simulink model "FeedBack_Linearization"  (R2021b)
(part 6 of 9)

t2824 = ct{938};
t2825 = ct{939};
t2826 = ct{940};
t2827 = ct{941};
t2828 = ct{942};
t2829 = ct{943};
t283 = ct{944};
t2832 = ct{945};
t2833 = ct{946};
t2837 = ct{947};
t2838 = ct{948};
t2839 = ct{949};
t284 = ct{950};
t2840 = ct{951};
t2841 = ct{952};
t2842 = ct{953};
t2844 = ct{954};
t2845 = ct{955};
t2846 = ct{956};
t2847 = ct{957};
t2848 = ct{958};
t285 = ct{959};
t2852 = ct{960};
t2854 = ct{961};
t2855 = ct{962};
t2857 = ct{963};
t2858 = ct{964};
t286 = ct{965};
t2861 = ct{966};
t2862 = ct{967};
t2864 = ct{968};
t2867 = ct{969};
t2868 = ct{970};
t2869 = ct{971};
t287 = ct{972};
t2871 = ct{973};
t2878 = ct{974};
t288 = ct{975};
t2880 = ct{976};
t2881 = ct{977};
t2882 = ct{978};
t2883 = ct{979};
t2884 = ct{980};
t2885 = ct{981};
t2886 = ct{982};
t2887 = ct{983};
t289 = ct{984};
t2891 = ct{985};
t2895 = ct{986};
t2897 = ct{987};
t2898 = ct{988};
t29 = ct{989};
t290 = ct{990};
t2900 = ct{991};
t2901 = ct{992};
t2903 = ct{993};
t2905 = ct{994};
t2907 = ct{995};
t2908 = ct{996};
t2909 = ct{997};
t2911 = ct{998};
t2912 = ct{999};
t2914 = ct{1000};
t2915 = ct{1001};
t2917 = ct{1002};
t2919 = ct{1003};
t2920 = ct{1004};
t2921 = ct{1005};
t2922 = ct{1006};
t2923 = ct{1007};
t2924 = ct{1008};
t2925 = ct{1009};
t2926 = ct{1010};
t2929 = ct{1011};
t293 = ct{1012};
t2930 = ct{1013};
t2931 = ct{1014};
t2935 = ct{1015};
t2936 = ct{1016};
t2937 = ct{1017};
t2939 = ct{1018};
t2940 = ct{1019};
t2941 = ct{1020};
t2942 = ct{1021};
t2943 = ct{1022};
t2944 = ct{1023};
t2945 = ct{1024};
t2946 = ct{1025};
t2947 = ct{1026};
t2948 = ct{1027};
t2949 = ct{1028};
t295 = ct{1029};
t2950 = ct{1030};
t2952 = ct{1031};
t2953 = ct{1032};
t2954 = ct{1033};
t2955 = ct{1034};
t2956 = ct{1035};
t2957 = ct{1036};
t2959 = ct{1037};
t296 = ct{1038};
t2960 = ct{1039};
t2961 = ct{1040};
t2962 = ct{1041};
t2968 = ct{1042};
t2969 = ct{1043};
t297 = ct{1044};
t2970 = ct{1045};
t2972 = ct{1046};
t2973 = ct{1047};
t2974 = ct{1048};
t2976 = ct{1049};
t298 = ct{1050};
t2980 = ct{1051};
t2981 = ct{1052};
t2982 = ct{1053};
t2985 = ct{1054};
t2989 = ct{1055};
t2990 = ct{1056};
t2991 = ct{1057};
t2992 = ct{1058};
t2993 = ct{1059};
t2994 = ct{1060};
t2995 = ct{1061};
t2996 = ct{1062};
t2997 = ct{1063};
t2998 = ct{1064};
t2999 = ct{1065};
t3 = ct{1066};
t30 = ct{1067};
t3001 = ct{1068};
t3003 = ct{1069};
t3005 = ct{1070};
t3007 = ct{1071};
t3008 = ct{1072};
t3009 = ct{1073};
t301 = ct{1074};
t3011 = ct{1075};
t3013 = ct{1076};
t3016 = ct{1077};
t3018 = ct{1078};
t3020 = ct{1079};
t3021 = ct{1080};
t3022 = ct{1081};
t3023 = ct{1082};
t3025 = ct{1083};
t3026 = ct{1084};
t3030 = ct{1085};
t3031 = ct{1086};
t3032 = ct{1087};
t3035 = ct{1088};
t3037 = ct{1089};
t3038 = ct{1090};
t3039 = ct{1091};
t3042 = ct{1092};
t3045 = ct{1093};
t3049 = ct{1094};
t3051 = ct{1095};
t3052 = ct{1096};
t3055 = ct{1097};
t3056 = ct{1098};
t3057 = ct{1099};
t3059 = ct{1100};
t3060 = ct{1101};
t3062 = ct{1102};
t3064 = ct{1103};
t3065 = ct{1104};
t3066 = ct{1105};
t3067 = ct{1106};
t3068 = ct{1107};
t307 = ct{1108};
t3070 = ct{1109};
t3071 = ct{1110};
t3073 = ct{1111};
t3075 = ct{1112};
t3076 = ct{1113};
t3079 = ct{1114};
t308 = ct{1115};
t3080 = ct{1116};
t3082 = ct{1117};
t3083 = ct{1118};
t3084 = ct{1119};
t3085 = ct{1120};
t3086 = ct{1121};
t3088 = ct{1122};
t309 = ct{1123};
t3090 = ct{1124};
t3092 = ct{1125};
t3093 = ct{1126};
t3094 = ct{1127};
t3096 = ct{1128};
t3097 = ct{1129};
t3098 = ct{1130};
t31 = ct{1131};
t310 = ct{1132};
t3101 = ct{1133};
t3102 = ct{1134};
t3103 = ct{1135};
t3104 = ct{1136};
t3108 = ct{1137};
t311 = ct{1138};
t3112 = ct{1139};
t3113 = ct{1140};
t3114 = ct{1141};
t3115 = ct{1142};
t3116 = ct{1143};
t3118 = ct{1144};
t3119 = ct{1145};
t312 = ct{1146};
t3120 = ct{1147};
t3121 = ct{1148};
t3122 = ct{1149};
t3124 = ct{1150};
t3126 = ct{1151};
t3128 = ct{1152};
t3129 = ct{1153};
t313 = ct{1154};
t3130 = ct{1155};
t3131 = ct{1156};
t3132 = ct{1157};
t3133 = ct{1158};
t3138 = ct{1159};
t3139 = ct{1160};
t3140 = ct{1161};
t3141 = ct{1162};
t3142 = ct{1163};
t3143 = ct{1164};
t3147 = ct{1165};
t3148 = ct{1166};
t3149 = ct{1167};
t3152 = ct{1168};
t3153 = ct{1169};
t3154 = ct{1170};
t3155 = ct{1171};
t3156 = ct{1172};
t3159 = ct{1173};
t3161 = ct{1174};
t3162 = ct{1175};
t3163 = ct{1176};
t3165 = ct{1177};
t3166 = ct{1178};
t3167 = ct{1179};
t3168 = ct{1180};
t317 = ct{1181};
t3170 = ct{1182};
t3171 = ct{1183};
t3172 = ct{1184};
t3175 = ct{1185};
t3176 = ct{1186};
t3179 = ct{1187};
t318 = ct{1188};
t3181 = ct{1189};
t3182 = ct{1190};
t3186 = ct{1191};
t3187 = ct{1192};
t319 = ct{1193};
t3190 = ct{1194};
t3191 = ct{1195};
t3192 = ct{1196};
t3193 = ct{1197};
t3194 = ct{1198};
t3195 = ct{1199};
t3196 = ct{1200};
t32 = ct{1201};
t320 = ct{1202};
t3201 = ct{1203};
t3202 = ct{1204};
t3203 = ct{1205};
t3204 = ct{1206};
t3205 = ct{1207};
t3206 = ct{1208};
t3208 = ct{1209};
t3210 = ct{1210};
t3211 = ct{1211};
t3212 = ct{1212};
t3213 = ct{1213};
t3214 = ct{1214};
t3215 = ct{1215};
t3216 = ct{1216};
t3220 = ct{1217};
t3222 = ct{1218};
t3223 = ct{1219};
t3224 = ct{1220};
t3225 = ct{1221};
t3226 = ct{1222};
t3227 = ct{1223};
t3228 = ct{1224};
t3229 = ct{1225};
t3230 = ct{1226};
t3231 = ct{1227};
t3232 = ct{1228};
t3233 = ct{1229};
t3235 = ct{1230};
t3236 = ct{1231};
t3237 = ct{1232};
t3238 = ct{1233};
t3240 = ct{1234};
t3241 = ct{1235};
t3242 = ct{1236};
t3243 = ct{1237};
t3244 = ct{1238};
t3246 = ct{1239};
t3247 = ct{1240};
t3248 = ct{1241};
t3249 = ct{1242};
t3250 = ct{1243};
t3251 = ct{1244};
t3252 = ct{1245};
t3253 = ct{1246};
t3254 = ct{1247};
t3255 = ct{1248};
t3256 = ct{1249};
t3257 = ct{1250};
t3259 = ct{1251};
t3261 = ct{1252};
t3262 = ct{1253};
t3263 = ct{1254};
t3264 = ct{1255};
t3267 = ct{1256};
t3268 = ct{1257};
t3269 = ct{1258};
t327 = ct{1259};
t3272 = ct{1260};
t3273 = ct{1261};
t3274 = ct{1262};
t3275 = ct{1263};
t3276 = ct{1264};
t3277 = ct{1265};
t3279 = ct{1266};
t328 = ct{1267};
t3280 = ct{1268};
t3281 = ct{1269};
t3282 = ct{1270};
t3284 = ct{1271};
t3285 = ct{1272};
t3286 = ct{1273};
t3287 = ct{1274};
t3288 = ct{1275};
t3289 = ct{1276};
t329 = ct{1277};
t3290 = ct{1278};
t3291 = ct{1279};
t3292 = ct{1280};
t3293 = ct{1281};
t3294 = ct{1282};
t3295 = ct{1283};
t3296 = ct{1284};
t3297 = ct{1285};
t33 = ct{1286};
t330 = ct{1287};
t3300 = ct{1288};
t3301 = ct{1289};
t3302 = ct{1290};
t3304 = ct{1291};
t3306 = ct{1292};
t3307 = ct{1293};
t3309 = ct{1294};
t331 = ct{1295};
t3310 = ct{1296};
t3311 = ct{1297};
t3312 = ct{1298};
t3313 = ct{1299};
t3321 = ct{1300};
t3324 = ct{1301};
t3326 = ct{1302};
t3328 = ct{1303};
t3330 = ct{1304};
t3331 = ct{1305};
t3333 = ct{1306};
t3336 = ct{1307};
t3337 = ct{1308};
t3338 = ct{1309};
t3339 = ct{1310};
t3342 = ct{1311};
t3343 = ct{1312};
t3345 = ct{1313};
t3351 = ct{1314};
t3352 = ct{1315};
t3354 = ct{1316};
t3355 = ct{1317};
t3356 = ct{1318};
t3357 = ct{1319};
t3358 = ct{1320};
t3359 = ct{1321};
t3360 = ct{1322};
t3361 = ct{1323};
t3362 = ct{1324};
t3363 = ct{1325};
t3364 = ct{1326};
t3365 = ct{1327};
t3368 = ct{1328};
t3369 = ct{1329};
t3371 = ct{1330};
t3372 = ct{1331};
t3373 = ct{1332};
t3374 = ct{1333};
t3375 = ct{1334};
t3377 = ct{1335};
t3379 = ct{1336};
t338 = ct{1337};
t3381 = ct{1338};
t3383 = ct{1339};
t3385 = ct{1340};
t3386 = ct{1341};
t3393 = ct{1342};
t3394 = ct{1343};
t3395 = ct{1344};
t3396 = ct{1345};
t3398 = ct{1346};
t3399 = ct{1347};
t34 = ct{1348};
t3400 = ct{1349};
t3403 = ct{1350};
t3404 = ct{1351};
t3406 = ct{1352};
t3407 = ct{1353};
t3408 = ct{1354};
t3409 = ct{1355};
t3411 = ct{1356};
t3415 = ct{1357};
t342 = ct{1358};
t3421 = ct{1359};
t3422 = ct{1360};
t3423 = ct{1361};
t3424 = ct{1362};
t3425 = ct{1363};
t3427 = ct{1364};
t3428 = ct{1365};
t3429 = ct{1366};
t3433 = ct{1367};
t3436 = ct{1368};
t3440 = ct{1369};
t3441 = ct{1370};
t3442 = ct{1371};
t3443 = ct{1372};
t3444 = ct{1373};
t3445 = ct{1374};
t3446 = ct{1375};
t3458 = ct{1376};
t346 = ct{1377};
t3462 = ct{1378};
t3464 = ct{1379};
t3465 = ct{1380};
t3467 = ct{1381};
t3468 = ct{1382};
t347 = ct{1383};
t3473 = ct{1384};
t3474 = ct{1385};
t3476 = ct{1386};
t3477 = ct{1387};
t348 = ct{1388};
t3484 = ct{1389};
t3486 = ct{1390};
t3488 = ct{1391};
t349 = ct{1392};
t3490 = ct{1393};
t3497 = ct{1394};
t35 = ct{1395};
t3502 = ct{1396};
t3503 = ct{1397};
t3504 = ct{1398};
t3510 = ct{1399};
t3512 = ct{1400};
t3514 = ct{1401};
t3519 = ct{1402};
t3520 = ct{1403};
t3521 = ct{1404};
t3522 = ct{1405};
t3523 = ct{1406};
t3525 = ct{1407};
t3538 = ct{1408};
t3539 = ct{1409};
t3540 = ct{1410};
t3541 = ct{1411};
t3542 = ct{1412};
t3543 = ct{1413};
t3546 = ct{1414};
t3547 = ct{1415};
t3553 = ct{1416};
t3562 = ct{1417};
t3572 = ct{1418};
t3573 = ct{1419};
t3574 = ct{1420};
t3576 = ct{1421};
t3578 = ct{1422};
t3579 = ct{1423};
t358 = ct{1424};
t3581 = ct{1425};
t3582 = ct{1426};
t3584 = ct{1427};
t3585 = ct{1428};
t3586 = ct{1429};
t3589 = ct{1430};
t3590 = ct{1431};
t3591 = ct{1432};
t3592 = ct{1433};
t3593 = ct{1434};
t3594 = ct{1435};
t3595 = ct{1436};
t3596 = ct{1437};
t3598 = ct{1438};
t3599 = ct{1439};
t36 = ct{1440};
t3600 = ct{1441};
t3610 = ct{1442};
t3619 = ct{1443};
t3620 = ct{1444};
t3622 = ct{1445};
t3623 = ct{1446};
t3628 = ct{1447};
t3631 = ct{1448};
t3633 = ct{1449};
t3634 = ct{1450};
t3635 = ct{1451};
t3636 = ct{1452};
t3637 = ct{1453};
t3640 = ct{1454};
t3641 = ct{1455};
t3666 = ct{1456};
t3667 = ct{1457};
t3668 = ct{1458};
t3669 = ct{1459};
t3670 = ct{1460};
t3671 = ct{1461};
t3672 = ct{1462};
t3673 = ct{1463};
t3674 = ct{1464};
t3679 = ct{1465};
t37 = ct{1466};
t3723 = ct{1467};
t3726 = ct{1468};
t3779 = ct{1469};
t3780 = ct{1470};
t3781 = ct{1471};
t3786 = ct{1472};
t3811 = ct{1473};
t3812 = ct{1474};
t3816 = ct{1475};
t39 = ct{1476};
t4 = ct{1477};
t40 = ct{1478};
t427 = ct{1479};
t428 = ct{1480};
t429 = ct{1481};
t43 = ct{1482};
t431 = ct{1483};
t432 = ct{1484};
t433 = ct{1485};
t434 = ct{1486};
t435 = ct{1487};
t436 = ct{1488};
t438 = ct{1489};
t439 = ct{1490};
t441 = ct{1491};
t442 = ct{1492};
t443 = ct{1493};
t444 = ct{1494};
t446 = ct{1495};
t448 = ct{1496};
t45 = ct{1497};
t450 = ct{1498};
t451 = ct{1499};
t452 = ct{1500};
t453 = ct{1501};
t455 = ct{1502};
t456 = ct{1503};
t457 = ct{1504};
t458 = ct{1505};
t459 = ct{1506};
t46 = ct{1507};
t460 = ct{1508};
t461 = ct{1509};
t463 = ct{1510};
t464 = ct{1511};
t465 = ct{1512};
t466 = ct{1513};
t467 = ct{1514};
t468 = ct{1515};
t469 = ct{1516};
t483 = ct{1517};
t484 = ct{1518};
t49 = ct{1519};
t494 = ct{1520};
t495 = ct{1521};
t496 = ct{1522};
t5 = ct{1523};
t50 = ct{1524};
t51 = ct{1525};
t510 = ct{1526};
t511 = ct{1527};
t512 = ct{1528};
t515 = ct{1529};
t516 = ct{1530};
t517 = ct{1531};
t518 = ct{1532};
t522 = ct{1533};
t523 = ct{1534};
t524 = ct{1535};
t525 = ct{1536};
t526 = ct{1537};
t527 = ct{1538};
t528 = ct{1539};
t529 = ct{1540};
t530 = ct{1541};
t531 = ct{1542};
t533 = ct{1543};
t534 = ct{1544};
t535 = ct{1545};
t536 = ct{1546};
t537 = ct{1547};
t538 = ct{1548};
t542 = ct{1549};
t543 = ct{1550};
t545 = ct{1551};
t546 = ct{1552};
t547 = ct{1553};
t548 = ct{1554};
t549 = ct{1555};
t55 = ct{1556};
t550 = ct{1557};
t551 = ct{1558};
t552 = ct{1559};
t553 = ct{1560};
t554 = ct{1561};
t556 = ct{1562};
t557 = ct{1563};
t558 = ct{1564};
t561 = ct{1565};
t562 = ct{1566};
t563 = ct{1567};
t564 = ct{1568};
t565 = ct{1569};
t566 = ct{1570};
t567 = ct{1571};
t568 = ct{1572};
t569 = ct{1573};
t57 = ct{1574};
t570 = ct{1575};
t571 = ct{1576};
t572 = ct{1577};
t573 = ct{1578};
t574 = ct{1579};
t575 = ct{1580};
t576 = ct{1581};
t577 = ct{1582};
t578 = ct{1583};
t579 = ct{1584};
t58 = ct{1585};
t580 = ct{1586};
t581 = ct{1587};
t582 = ct{1588};
t583 = ct{1589};
t584 = ct{1590};
t585 = ct{1591};
t586 = ct{1592};
t587 = ct{1593};
t588 = ct{1594};
t589 = ct{1595};
t590 = ct{1596};
t591 = ct{1597};
t592 = ct{1598};
t593 = ct{1599};
t594 = ct{1600};
t595 = ct{1601};
t596 = ct{1602};
t597 = ct{1603};
t598 = ct{1604};
t599 = ct{1605};
t6 = ct{1606};
t600 = ct{1607};
t601 = ct{1608};
t602 = ct{1609};
t603 = ct{1610};
t604 = ct{1611};
t605 = ct{1612};
t606 = ct{1613};
t607 = ct{1614};
t608 = ct{1615};
t609 = ct{1616};
t61 = ct{1617};
t612 = ct{1618};
t613 = ct{1619};
t614 = ct{1620};
t615 = ct{1621};
t616 = ct{1622};
t617 = ct{1623};
t618 = ct{1624};
t619 = ct{1625};
t620 = ct{1626};
t621 = ct{1627};
t622 = ct{1628};
t624 = ct{1629};
t626 = ct{1630};
t629 = ct{1631};
t63 = ct{1632};
t631 = ct{1633};
t632 = ct{1634};
t633 = ct{1635};
t634 = ct{1636};
t635 = ct{1637};
t637 = ct{1638};
t639 = ct{1639};
t64 = ct{1640};
t640 = ct{1641};
t642 = ct{1642};
t643 = ct{1643};
t644 = ct{1644};
t646 = ct{1645};
t647 = ct{1646};
t648 = ct{1647};
t649 = ct{1648};
t650 = ct{1649};
t651 = ct{1650};
t652 = ct{1651};
t653 = ct{1652};
t654 = ct{1653};
t656 = ct{1654};
t657 = ct{1655};
t658 = ct{1656};
t660 = ct{1657};
t661 = ct{1658};
t662 = ct{1659};
t663 = ct{1660};
t664 = ct{1661};
t665 = ct{1662};
t667 = ct{1663};
t67 = ct{1664};
t673 = ct{1665};
t676 = ct{1666};
t677 = ct{1667};
t678 = ct{1668};
t685 = ct{1669};
t686 = ct{1670};
t687 = ct{1671};
t688 = ct{1672};
t689 = ct{1673};
t69 = ct{1674};
t691 = ct{1675};
t692 = ct{1676};
t693 = ct{1677};
t694 = ct{1678};
t696 = ct{1679};
t697 = ct{1680};
t698 = ct{1681};
t7 = ct{1682};
t70 = ct{1683};
t701 = ct{1684};
t702 = ct{1685};
t703 = ct{1686};
t704 = ct{1687};
t705 = ct{1688};
t707 = ct{1689};
t708 = ct{1690};
t71 = ct{1691};
t72 = ct{1692};
t721 = ct{1693};
t722 = ct{1694};
t723 = ct{1695};
t724 = ct{1696};
t725 = ct{1697};
t726 = ct{1698};
t728 = ct{1699};
t729 = ct{1700};
t73 = ct{1701};
t730 = ct{1702};
t731 = ct{1703};
t735 = ct{1704};
t74 = ct{1705};
t740 = ct{1706};
t743 = ct{1707};
t75 = ct{1708};
t754 = ct{1709};
t755 = ct{1710};
t756 = ct{1711};
t757 = ct{1712};
t759 = ct{1713};
t76 = ct{1714};
t760 = ct{1715};
t762 = ct{1716};
t769 = ct{1717};
t77 = ct{1718};
t770 = ct{1719};
t773 = ct{1720};
t774 = ct{1721};
t776 = ct{1722};
t777 = ct{1723};
t778 = ct{1724};
t78 = ct{1725};
t782 = ct{1726};
t785 = ct{1727};
t786 = ct{1728};
t787 = ct{1729};
t788 = ct{1730};
t79 = ct{1731};
t791 = ct{1732};
t792 = ct{1733};
t795 = ct{1734};
t796 = ct{1735};
t797 = ct{1736};
t8 = ct{1737};
t80 = ct{1738};
t800 = ct{1739};
t805 = ct{1740};
t806 = ct{1741};
t81 = ct{1742};
t813 = ct{1743};
t814 = ct{1744};
t815 = ct{1745};
t816 = ct{1746};
t817 = ct{1747};
t818 = ct{1748};
t819 = ct{1749};
t82 = ct{1750};
t827 = ct{1751};
t83 = ct{1752};
t831 = ct{1753};
t834 = ct{1754};
t835 = ct{1755};
t836 = ct{1756};
t837 = ct{1757};
t838 = ct{1758};
t839 = ct{1759};
t84 = ct{1760};
t840 = ct{1761};
t841 = ct{1762};
t842 = ct{1763};
t843 = ct{1764};
t845 = ct{1765};
t846 = ct{1766};
t847 = ct{1767};
t85 = ct{1768};
t853 = ct{1769};
t854 = ct{1770};
t855 = ct{1771};
t856 = ct{1772};
t857 = ct{1773};
t859 = ct{1774};
t86 = ct{1775};
t860 = ct{1776};
t863 = ct{1777};
t864 = ct{1778};
t866 = ct{1779};
t867 = ct{1780};
t87 = ct{1781};
t870 = ct{1782};
t871 = ct{1783};
t873 = ct{1784};
t876 = ct{1785};
t877 = ct{1786};
t878 = ct{1787};
t88 = ct{1788};
t880 = ct{1789};
t881 = ct{1790};
t882 = ct{1791};
t884 = ct{1792};
t885 = ct{1793};
t888 = ct{1794};
t889 = ct{1795};
t89 = ct{1796};
t890 = ct{1797};
t891 = ct{1798};
t896 = ct{1799};
t898 = ct{1800};
t899 = ct{1801};
t9 = ct{1802};
t90 = ct{1803};
t900 = ct{1804};
t902 = ct{1805};
t905 = ct{1806};
t907 = ct{1807};
t908 = ct{1808};
t91 = ct{1809};
t911 = ct{1810};
t92 = ct{1811};
t921 = ct{1812};
t922 = ct{1813};
t926 = ct{1814};
t927 = ct{1815};
t928 = ct{1816};
t930 = ct{1817};
t932 = ct{1818};
t933 = ct{1819};
t935 = ct{1820};
t939 = ct{1821};
t94 = ct{1822};
t940 = ct{1823};
t942 = ct{1824};
t946 = ct{1825};
t948 = ct{1826};
t949 = ct{1827};
t952 = ct{1828};
t958 = ct{1829};
t959 = ct{1830};
t961 = ct{1831};
t963 = ct{1832};
t966 = ct{1833};
t969 = ct{1834};
t97 = ct{1835};
t972 = ct{1836};
t973 = ct{1837};
t974 = ct{1838};
t975 = ct{1839};
t982 = ct{1840};
t983 = ct{1841};
t984 = ct{1842};
t987 = ct{1843};
t988 = ct{1844};
t992 = ct{1845};
t994 = ct{1846};
t999 = ct{1847};
t3752 = t3726.*2.9e-4;
t3753 = t3726.*2.900000000000001e-4;
t3754 = t3726.*2.94e-3;
t3764 = t2424+t2589+t3092+t3093+t3114+t3122;
t3777 = t347+t348+t358+t443+t446+t534+t1786+t1946+t1971+t1976+t2193+t2251+t2270+t2614+t2637+t2647+t3013+t3018;
t3778 = t448+t452+t468+t511+t531+t814+t1119+t1644+t1875+t1897+t1899+t2065+t2237+t2242+t2537+t2543+t2560+t2992+t2994;
t3784 = t588+t592+t593+t1166+t1167+t1194+t1200+t1201+t1203+t1663+t1705+t1759+t1841+t1884+t2028+t2047+t2078+t2486+t2539+t2568+t2596+t2598+t3065+t3068;
t3821 = t483+t484+t495+t496+t549+t550+t576+t582+t584+t585+t1807+t1978+t1982+t1988+t2197+t2310+t2311+t2606+t2629+t2646+t2669+t3021+t3023+t3102+t3103+t3116+t3519+t3520;
t3824 = t2440+t2458+t2459+t2551+t2757+t2771+t2812+t2869+t2885+t2909+t2912+t2915+t2921+t3056+t3062+t3220+t3225+t3240+t3244;
t3825 = t2469+t2470+t2472+t2623+t2748+t2775+t2793+t2898+t2901+t2911+t2920+t2937+t2940+t3049+t3057+t3224+t3228+t3236+t3241;
t3826 = t2409+t2474+t2475+t2506+t2766+t2774+t2833+t2847+t2848+t2905+t2908+t2917+t2919+t3064+t3073+t3223+t3227+t3247+t3251;
t2362 = -t2355;
t2371 = -t2367;
t2511 = -t2504;
t2544 = -t2524;
t2889 = -t2881;
t2894 = -t2883;
t2986 = -t2981;
t3002 = -t2993;
t3004 = -t2996;
t3010 = -t3003;
t3012 = -t3008;
t3033 = -t3030;
t3040 = t8.*t3038;
t3041 = t15.*t3038;
t3047 = t8.*t3045;
t3048 = t15.*t3045;
t3099 = t759+t1014+t1913+t2660;
t3151 = -t3143;
t3164 = -t3152;
t3199 = -t3194;
t3260 = -t3257;
t3265 = -t3263;
t3270 = -t3268;
t3283 = -t3280;
t3298 = -t3296;
t3303 = -t3301;
t3315 = t8.*t3312;
t3316 = t15.*t3312;
t3334 = dq7.*t3333.*2.0;
t3340 = -t3312.*(t653-t838);
t3341 = t3333.*(-3.466000000000001e-2);
t3347 = t3333.*3.466000000000001e-2;
t3348 = dq7.*t3333.*(-4.648e-2);
t3353 = dq7.*t3333.*4.648e-2;
t3366 = -t3360;
t3367 = -t3363;
t3370 = -t3369;
t3378 = -t3375;
t3380 = -t3377;
t3387 = t2161+t3321;
t3388 = t3312.*(t653-t838).*(-3.0e-5);
t3389 = t3312.*(t653-t838).*3.0e-5;
t3390 = t3312.*(t653-t838).*(-5.0e-5);
t3391 = t3312.*(t653-t838).*(-5.000000000000004e-4);
t3392 = t3356.*3.0e-5;
t3397 = t3356.*5.0e-5;
t3402 = t3356.*5.000000000000004e-4;
t3410 = t3360.*2.2e-4;
t3412 = t3360.*2.900000000000001e-4;
t3416 = t3360.*7.950000000000001e-3;
t3418 = t2601.*t3312;
t3426 = t946+t1803+t2514+t3153;
t3430 = t8.*t3423;
t3431 = t15.*t3423;
t3448 = -t3442;
t3450 = -t3445;
t3451 = t3377.*4.000000000000028e-5;
t3452 = t3377.*3.0e-5;
t3460 = t1046+t1797+t2665+t3118;
t3463 = t3377.*2.32e-3;
t3469 = t1038+t1787+t2706+t3128;
t3470 = t1039+t1753+t2718+t3129;
t3472 = t1046+t1797+t2690+t3138;
t3478 = -t3423.*(t88-t617);
t3479 = t3423.*(t88-t617);
t3482 = t1472+t1657+t1658+t2837+t2867;
t3483 = t1488+t1613+t1660+t2838+t2871;
t3487 = -t3436.*(t92-t663);
t3489 = t2816.*t3312;
t3492 = t1584+t1650+t1687+t2858+t2884;
t3495 = t3427.*4.9e-4;
t3496 = t3428.*2.019e-2;
t3505 = t1090+t1858+t2744+t3193;
t3507 = t3441.*4.9e-4;
t3508 = t3428.*1.9738e-1;
t3509 = t3442.*2.019e-2;
t3513 = t3446.*3.466000000000001e-2;
t3515 = t3445.*2.324e-2;
t3516 = t3442.*1.9738e-1;
t3532 = t3421.*(-1.089e-2);
t3533 = t3421.*(-2.9e-4);
t3534 = t3421.*(-2.2e-4);
t3535 = t3421.*1.089e-2;
t3536 = t3421.*2.9e-4;
t3537 = t3421.*2.2e-4;
t3544 = t2000.*t3423;
t3549 = -t3436.*(t1529+t15.*(t92-t663));
t3550 = t3436.*(t1529+t15.*(t92-t663));
t3555 = t3484.*9.999999999999998e-6;
t3558 = t3436.*(t92-t663).*(-3.0e-5);
t3559 = t3484.*2.769999999999999e-3;
t3560 = t3436.*(t92-t663).*3.0e-5;
t3561 = t3484.*1.0e-5;
t3563 = t3436.*(t92-t663).*(-5.0e-5);
t3565 = t3436.*(t92-t663).*(-5.000000000000004e-4);
t3567 = t3436.*(t92-t663).*5.000000000000004e-4;
t3605 = t3547.*4.000000000000028e-5;
t3607 = t3547.*5.0e-5;
t3608 = t3547.*2.81e-3;
t3617 = t1626+t2064+t2824+t3326;
t3618 = t1583+t2067+t2826+t3333;
t3621 = -t3312.*(t1487+t2219-t2864+dq6.*t7.*(t88-t617));
t3626 = t2074.*t3619;
t3627 = t2074.*t3620;
t3629 = t3312.*(t1487+t2219-t2864+dq6.*t7.*(t88-t617)).*(-3.0e-5);
t3630 = t3312.*(t1487+t2219-t2864+dq6.*t7.*(t88-t617)).*(-4.000000000000028e-5);
t3632 = t3312.*(t1487+t2219-t2864+dq6.*t7.*(t88-t617)).*(-2.32e-3);
t3639 = t2627.*t3619;
t3680 = -t3619.*(t884+t1578-t2180+t14.*(t639-t1128-t2181+dq5.*t13.*(t86-t652)));
t3681 = t3619.*(t884+t1578-t2180+t14.*(t639-t1128-t2181+dq5.*t13.*(t86-t652)));
t3682 = -t3620.*(t884+t1578-t2180+t14.*(t639-t1128-t2181+dq5.*t13.*(t86-t652)));
t3683 = t3620.*(t884+t1578-t2180+t14.*(t639-t1128-t2181+dq5.*t13.*(t86-t652)));
t3684 = t922+t1557+t2278+t2882+t2973+t3427;
t3688 = t963+t1606+t2245+t2887+t2969+t3441;
t3737 = t3723.*(-2.2e-4);
t3738 = t3723.*(-2.900000000000001e-4);
t3739 = t3723.*2.2e-4;
t3740 = t3723.*2.900000000000001e-4;
t3741 = t3723.*(-7.950000000000001e-3);
t3742 = t3723.*7.950000000000001e-3;
t3769 = t3619.*t3620;
t3787 = t2711+t2777+t2808+t2954+t2959+t3147+t3167+t3179+t3187;
t3788 = t2675+t2806+t2855+t2930+t2939+t3156+t3176+t3208+t3213;
t3790 = t432+t543+t551+t552+t558+t586+t587+t597+t598+t599+t1341+t1342+t1412+t1416+t1417+t1418+t1694+t1704+t1731+t1936+t1939+t2077+t2098+t2141+t2525+t2538+t2572+t2597+t2603+t3096+t3101;
t3791 = t2821+t3059+t3330+t3338+t3510+t3521;
t3798 = t448+t452+t468+t511+t531+t814+t1119+t1975+t2293+t2313+t2319+t2500+t2505+t2628+t3001+t3007+t3026+t3343+t3354;
t3050 = -t3047;
t3106 = t8.*t3099;
t3107 = t15.*t3099;
t3382 = t2119+t3315;
t3384 = t2140+t3316;
t3413 = -t3410;
t3414 = -t3412;
t3417 = -t3416;
t3419 = -t3418;
t3434 = -t3431;
t3437 = t987+t1806+t2516+t3164;
t3457 = -t3452;
t3480 = t1472+t1658+t2867+t3040;
t3481 = t1488+t1613+t2871+t3041;
t3491 = t1584+t1650+t2858+t3048;
t3493 = -t3489;
t3494 = t1619+t1651+t1652+t2862+t2894;
t3498 = -t3496;
t3500 = t3431.*3.466000000000001e-2;
t3501 = t3430.*2.324e-2;
t3506 = t1062+t1854+t2743+t3199;
t3511 = -t3507;
t3518 = -t3516;
t3526 = t3418.*1.089e-2;
t3527 = t3418.*2.9e-4;
t3528 = t3418.*2.2e-4;
t3545 = -t3544;
t3551 = t3479.*(-9.999999999999998e-6);
t3552 = t3479.*9.999999999999998e-6;
t3554 = t3479.*(-1.0e-5);
t3556 = t3479.*(-2.769999999999999e-3);
t3557 = t3479.*2.769999999999999e-3;
t3564 = -t3561;
t3566 = t3489.*3.0e-5;
t3568 = t3489.*5.0e-5;
t3571 = t3489.*5.000000000000004e-4;
t3601 = t3544.*4.000000000000028e-5;
t3602 = t3544.*5.0e-5;
t3604 = t3544.*2.81e-3;
t3606 = -t3605;
t3609 = -t3608;
t3611 = t3550.*(-2.2e-4);
t3612 = t3550.*(-1.089e-2);
t3613 = t3550.*(-2.9e-4);
t3614 = t3550.*2.2e-4;
t3615 = t3550.*1.089e-2;
t3616 = t3550.*2.9e-4;
t3624 = -t3617.*(t1386+t7.*(t88-t617));
t3625 = -t3618.*(t1386+t7.*(t88-t617));
t3638 = t2576.*t3618;
t3642 = t3617.*(t1386+t7.*(t88-t617)).*(-2.900000000000001e-4);
t3643 = t3618.*(t1386+t7.*(t88-t617)).*(-2.900000000000001e-4);
t3644 = t3617.*(t1386+t7.*(t88-t617)).*(-2.2e-4);
t3645 = t3618.*(t1386+t7.*(t88-t617)).*(-2.2e-4);
t3646 = t3617.*(t1386+t7.*(t88-t617)).*2.900000000000001e-4;
t3647 = t3617.*(t1386+t7.*(t88-t617)).*2.2e-4;
t3648 = t3617.*(t1386+t7.*(t88-t617)).*(-7.950000000000001e-3);
t3649 = t3618.*(t1386+t7.*(t88-t617)).*(-7.950000000000001e-3);
t3650 = t3617.*(t1386+t7.*(t88-t617)).*7.950000000000001e-3;
t3651 = t3626.*2.900000000000001e-4;
t3652 = t3626.*2.2e-4;
t3653 = t3626.*7.950000000000001e-3;
t3654 = t3627.*2.900000000000001e-4;
t3655 = t3627.*2.2e-4;
t3658 = t3627.*7.950000000000001e-3;
t3663 = t3639.*2.900000000000001e-4;
t3664 = t3639.*2.9e-4;
t3665 = t3639.*2.94e-3;
t3676 = t2961+t3340+t3362;
t3677 = t3312.*t3617;
t3678 = t3312.*t3618;
t3685 = t999+t1564+t2280+t2889+t2970+t3428;
t3686 = t8.*t3684;
t3687 = t15.*t3684;
t3689 = t961+t1645+t2233+t2886+t2968+t3448;
t3690 = t8.*t3688;
t3691 = t15.*t3688;
t3700 = t3025+t3379+t3380;
t3701 = t3681.*(-1.089e-2);
t3702 = t3681.*(-2.9e-4);
t3703 = t3681.*(-2.2e-4);
t3704 = t3681.*1.089e-2;
t3705 = t3681.*2.9e-4;
t3706 = t3681.*2.2e-4;
t3707 = t3683.*(-2.2e-4);
t3708 = t3683.*(-2.900000000000001e-4);
t3709 = t3683.*2.2e-4;
t3710 = t3683.*2.900000000000001e-4;
t3711 = t3683.*(-7.950000000000001e-3);
t3712 = t3683.*7.950000000000001e-3;
t3724 = -t3684.*(t1386+t7.*(t88-t617));
t3725 = t2074.*t3688;
t3745 = t3684.*(t1386+t7.*(t88-t617)).*(-4.000000000000028e-5);
t3746 = t3684.*(t1386+t7.*(t88-t617)).*(-3.0e-5);
t3747 = t3684.*(t1386+t7.*(t88-t617)).*(-2.32e-3);
t3766 = t3617.*t3618;
t3773 = t3769.*2.900000000000001e-4;
t3774 = t3769.*2.9e-4;
t3775 = t3769.*2.94e-3;
t3776 = t438+t442+t464+t467+t533+t782+t1274+t1678+t1835+t1877+t1900+t2032+t2195+t2200+t2556+t2578+t2599+t2985+t3002;
t3783 = t2586+t3037+t3115+t3119+t3479+t3484;
t3785 = t2447+t2783+t2839+t2852+t2903+t3130+t3151+t3231+t3233;
t3796 = t438+t442+t464+t467+t533+t782+t1274+t1977+t2249+t2290+t2297+t2485+t2487+t2644+t2976+t2982+t3022+t3345+t3347;
t3818 = t2929+t3182+t3222+t3250+t3259+t3389+t3396+t3463+t3467;
t3820 = t2952+t3191+t3212+t3256+t3267+t3390+t3404+t3451+t3462;
t3438 = t1038+t1787+t2643+t3106;
t3439 = t1039+t1753+t2661+t3107;
t3499 = t1619+t1652+t2862+t3050;
t3529 = -t3526;
t3530 = -t3527;
t3531 = -t3528;
t3569 = -t3568;
t3603 = -t3602;
t3656 = -t3654;
t3657 = -t3655;
t3659 = -t3658;
t3660 = t3638.*2.900000000000001e-4;
t3661 = t3638.*2.9e-4;
t3662 = t3638.*2.94e-3;
t3694 = t3677.*2.2e-4;
t3695 = t3678.*2.2e-4;
t3696 = t3677.*2.900000000000001e-4;
t3697 = t3678.*1.089e-2;
t3698 = t3678.*2.9e-4;
t3699 = t3677.*7.950000000000001e-3;
t3713 = t3686.*3.466000000000001e-2;
t3714 = t3687.*2.324e-2;
t3716 = -t3685.*(t653-t838);
t3717 = t3690.*3.466000000000001e-2;
t3718 = t3691.*2.324e-2;
t3720 = -t3689.*(t614+t13.*(t86-t652));
t3721 = t3689.*(t614+t13.*(t86-t652));
t3727 = t3685.*(t653-t838).*(-3.0e-5);
t3728 = t3685.*(t653-t838).*3.0e-5;
t3729 = t3685.*(t653-t838).*(-5.0e-5);
t3730 = t3685.*(t653-t838).*(-5.000000000000004e-4);
t3731 = t3685.*(t653-t838).*5.000000000000004e-4;
t3736 = t2601.*t3685;
t3743 = t2654.*t3689;
t3748 = t3725.*4.000000000000028e-5;
t3749 = t3725.*3.0e-5;
t3750 = t3725.*2.32e-3;
t3751 = t3113+t3419+t3425;
t3770 = t3766.*2.9e-4;
t3771 = t3766.*2.900000000000001e-4;
t3772 = t3766.*2.94e-3;
t3782 = t3365+t3624+t3627;
t3789 = t3385+t3638+t3639;
t3792 = t1608+t2103+t2846+t3334+t3430+t3687;
t3793 = t1647+t2100+t2845+t3328+t3434+t3686;
t3794 = t1642+t2132+t2880+t3331+t3450+t3691;
t3795 = t1680+t2142+t2878+t3337+t3446+t3690;
t3799 = t2074.*(t2132+t2880+t3331+t3450+t3691-t8.*t22.*(t614+t13.*(t86-t652)));
t3817 = t3108+t3139+t3497+t3512+t3545+t3547;
t3819 = t2946+t3196+t3211+t3253+t3262+t3391+t3408+t3457+t3458;
t3822 = t547+t548+t575+t580+t581+t583+t588+t592+t593+t800+t1424+t1726+t1856+t1898+t1934+t2042+t2198+t2231+t2253+t2558+t2581+t2587+t2602+t2991+t2997+t3066+t3075+t3082+t3495+t3498;
t3823 = t545+t546+t557+t577+t578+t579+t589+t590+t591+t816+t1180+t1683+t1938+t1941+t1954+t2105+t2257+t2286+t2316+t2509+t2555+t2559+t2577+t2990+t2995+t3079+t3080+t3084+t3509+t3511;
t3828 = t3339+t3525+t3621+t3622+t3724+t3725;
t3834 = t2767+t2820+t2907+t3070+t3216+t3237+t3238+t3243+t3246+t3254+t3270+t3273+t3378+t3383+t3552+t3555+t3590+t3600;
t3836 = t2895+t2926+t2947+t3016+t3214+t3226+t3279+t3281+t3292+t3298+t3309+t3311+t3367+t3368+t3553+t3554+t3562+t3564;
t3837 = t2844+t2914+t2922+t3055+t3230+t3242+t3264+t3274+t3283+t3284+t3297+t3303+t3370+t3371+t3557+t3559+t3574+t3586;
t3715 = -t3713;
t3719 = -t3718;
t3732 = t3721.*(-3.0e-5);
t3733 = t3721.*(-5.0e-5);
t3734 = t3721.*5.0e-5;
t3735 = t3721.*(-5.000000000000004e-4);
t3744 = -t3743;
t3755 = t3736.*1.089e-2;
t3756 = t3736.*2.9e-4;
t3757 = t3736.*2.2e-4;
t3758 = t3743.*1.089e-2;
t3759 = t3743.*2.9e-4;
t3760 = t3743.*2.2e-4;
t3797 = -t3792.*(t1386+t7.*(t88-t617));
t3800 = t2576.*t3793;
t3801 = t3792.*(t1386+t7.*(t88-t617)).*(-2.2e-4);
t3802 = t3792.*(t1386+t7.*(t88-t617)).*(-2.900000000000001e-4);
t3803 = t2627.*t3795;
t3804 = t3792.*(t1386+t7.*(t88-t617)).*(-7.950000000000001e-3);
t3805 = t3799.*2.2e-4;
t3806 = t3799.*2.900000000000001e-4;
t3807 = t3799.*7.950000000000001e-3;
t3827 = t3149+t3487+t3493+t3503+t3716+t3721;
t3830 = t3289+t3409+t3473+t3529+t3539+t3647+t3657+t3661+t3664;
t3831 = t3294+t3415+t3474+t3531+t3543+t3650+t3659+t3660+t3663;
t3832 = t3291+t3411+t3477+t3530+t3541+t3646+t3656+t3662+t3665;
t3761 = -t3758;
t3762 = -t3759;
t3763 = -t3760;
t3808 = t3800.*2.9e-4;
t3809 = t3800.*2.900000000000001e-4;
t3810 = t3800.*2.94e-3;
t3813 = t3803.*2.9e-4;
t3814 = t3803.*2.900000000000001e-4;
t3815 = t3803.*2.94e-3;
t3829 = t3523+t3550+t3678+t3681+t3736+t3744;
t3833 = t547+t548+t575+t580+t581+t583+t588+t592+t593+t800+t1424+t1998+t2231+t2288+t2309+t2312+t2510+t2511+t2657+t2980+t2986+t3033+t3090+t3353+t3355+t3500+t3501+t3508+t3714+t3715;
t3835 = t545+t546+t557+t577+t578+t579+t589+t590+t591+t816+t1180+t1997+t2316+t2327+t2333+t2339+t2517+t2544+t2633+t3005+t3010+t3032+t3094+t3351+t3352+t3513+t3515+t3518+t3717+t3719;
t3838 = t3522+t3677+t3683+t3723+t3797+t3799;
t3839 = t3623+t3726+t3766+t3769+t3800+t3803;
t3840 = t3275+t3300+t3302+t3381+t3560+t3566+t3572+t3576+t3579+t3598+t3601+t3606+t3632+t3634+t3728+t3732+t3747+t3750;
t3841 = t3276+t3304+t3307+t3374+t3567+t3571+t3573+t3582+t3585+t3591+t3603+t3607+t3629+t3631+t3731+t3735+t3746+t3749;
t3842 = t3282+t3306+t3310+t3373+t3563+t3569+t3578+t3581+t3584+t3589+t3604+t3609+t3630+t3633+t3729+t3734+t3745+t3748;
t3843 = t3592+t3594+t3615+t3635+t3694+t3697+t3704+t3709+t3739+t3752+t3755+t3761+t3770+t3774+t3801+t3805+t3808+t3813;
t3844 = t3593+t3596+t3616+t3637+t3696+t3698+t3705+t3710+t3740+t3754+t3756+t3762+t3772+t3775+t3802+t3806+t3810+t3815;
t3845 = t3595+t3599+t3614+t3636+t3695+t3699+t3706+t3712+t3742+t3753+t3757+t3763+t3771+t3773+t3804+t3807+t3809+t3814;
et1 = t2627.*(t1386+t7.*(t88-t617)).*7.950000000000001e-3+t2654.*(t1386+t7.*(t88-t617)).*2.2e-4;
et2 = t2074.*t2576.*7.950000000000001e-3+t2074.*t2601.*2.2e-4;
et3 = t2601.*t2627.*2.900000000000001e-4-t2576.*t2654.*2.900000000000001e-4;
et4 = dq2.*t3.*t23.*3.199999999999801e-4+dq2.*t3.*t26.*3.199999999999801e-4;
et5 = dq2.*t10.*t23.*(-5.582083966615414e-19)-dq2.*t10.*t26.*5.582083966615414e-19;
et6 = t88.*1.8866e-1+t281-t617.*1.8866e-1-t653.*2.37e-3+t661.*5.000000000000001e-5;
et7 = t835.*5.000000000000001e-5+t838.*2.37e-3;
et8 = t815.*t2147+t831.*t2164-t2148.*(t88-t617)-t2163.*(t86-t652);
et9 = (t2341+t2445.*4.988e-2-t2463-t2612+t2624-t2796+t2813+t2900+t1066.*(t86-t652).*1.11e-3).*(-1.0./2.0);
et10 = t3.*t23.*1.16152294893368e-19+t3.*t26.*1.16152294893368e-19+t10.*t23.*8.909980864224564e-21;
et11 = t10.*t26.*8.909980864224564e-21;
et12 = -t3196-t3253-t3262+t3406+t3452+t2074.*(t878-t1582+t2184+t7.*(t639-t1128-t2181+dq5.*t13.*(t86-t652))).*3.0e-5+t2196.*(t621-t864).*5.0e-5;
et13 = t3312.*(t653-t838).*5.000000000000004e-4+t1207.*(t642+t896-t1137-t2220).*3.0e-5;
et14 = t831.*t1040-t572.*t2163-t604.*t2147+t1066.*(t88-t617);
et15 = (t2365+t2445.*1.12e-3-t2456+t2536-t2653-t2789+t2803+t2868+t1066.*(t86-t652).*8.8e-4).*(-1.0./2.0);
et16 = t572.*t815.*1.11e-3-t604.*t831.*1.12e-3;
et17 = t815.*t831.*4.988e-2-t572.*(t88-t617).*1.12e-3;
et18 = t604.*(t86-t652).*1.11e-3-(t88-t617).*(t86-t652).*4.988e-2;
et19 = t1206.*(t614+t13.*(t86-t652)).*1.2e-4+t831.*t1206.*4.466636216449161e-20;
et20 = (t614+t13.*(t86-t652)).*(t88-t617).*(-9.999999999999998e-6)+t1295.*(t88-t617).*4.466636216449161e-20;
et21 = t831.*(t653-t838).*(-9.999999999999998e-6)-t1295.*(t653-t838).*1.2e-4;
et22 = t29.*(-3.818e-2)+t70.*2.0e-4+t85.*3.818e-2-t88.*5.267999999999999e-2+t281;
et23 = t612.*2.0e-4+t617.*5.267999999999999e-2;
et24 = t32.*3.818e-2+t76.*3.818e-2-t79.*5.267999999999999e-2+t86.*2.0e-4+t271;
et25 = t652.*(-2.0e-4)-t660.*5.267999999999999e-2;
et26 = -t3291+t3365.*2.900000000000001e-4+t3527+t3642+t3654-t3662-t3665+t2654.*(t884+t1578-t2180+t14.*(t639-t1128-t2181+dq5.*t13.*(t86-t652))).*2.9e-4;
et27 = t3336.*(t8.*(t92-t663)+t15.*(t621-t864)).*2.94e-3;
et28 = t571.*t572.*7.299999999999999e-4-t604.*t605.*7.299999999999999e-4;
et29 = t2.*t10.*t571.*7.000000000000022e-5-t9.*t10.*t572.*7.000000000000001e-5;
et30 = t2.*t10.*t604.*(-7.000000000000001e-5)+t9.*t10.*t605.*7.000000000000022e-5;
et31 = dq2.*t3.*t23.*5.582083966615414e-19+dq2.*t3.*t26.*5.582083966615414e-19-dq2.*t10.*t23.*1.0e-4;
et32 = dq2.*t10.*t26.*(-1.0e-4);
et33 = t79.*1.8866e-1+t271+t614.*2.37e-3-t619.*5.000000000000001e-5+t660.*1.8866e-1;
et34 = t6.*(t86-t652).*5.000000000000001e-5+t13.*(t86-t652).*2.37e-3;
et35 = t2000.*(t884+t1578-t2180+t14.*(t639-t1128-t2181+dq5.*t13.*(t86-t652))).*2.32e-3-t3312.*(t614+t13.*(t86-t652)).*3.0e-5;
et36 = t2832.*(t1386+t7.*(t88-t617)).*3.0e-5+t2000.*t2832.*4.000000000000028e-5;
et37 = t2035.*t2816.*(-4.000000000000028e-5)+t2074.*t2816.*3.0e-5;
et38 = t2035.*t3312.*(-2.32e-3)+(t653-t838).*(t878-t1582+t2184+t7.*(t639-t1128-t2181+dq5.*t13.*(t86-t652))).*4.000000000000028e-5;
et39 = (t653-t838).*(t884+t1578-t2180+t14.*(t639-t1128-t2181+dq5.*t13.*(t86-t652))).*3.0e-5;
et40 = (t614+t13.*(t86-t652)).*(t1487+t2219-t2864+dq6.*t7.*(t88-t617)).*4.000000000000028e-5+t2074.*(t1487+t2219-t2864+dq6.*t7.*(t88-t617)).*2.32e-3;
et41 = (t1386+t7.*(t88-t617)).*(t878-t1582+t2184+t7.*(t639-t1128-t2181+dq5.*t13.*(t86-t652))).*(-2.32e-3);
et42 = t2000.*(t614+t13.*(t86-t652)).*4.000000000000028e-5+t2035.*(t1386+t7.*(t88-t617)).*2.32e-3;
et43 = t2000.*t2074.*2.32e-3-t2035.*(t653-t838).*4.000000000000028e-5;
et44 = t2074.*(t653-t838).*3.0e-5+(t614+t13.*(t86-t652)).*(t1386+t7.*(t88-t617)).*3.0e-5;
et45 = t1206.*(t614+t13.*(t86-t652)).*(-9.999999999999998e-6)+t831.*t1206.*1.0e-5;
et46 = (t614+t13.*(t86-t652)).*(t88-t617).*2.769999999999999e-3+t1295.*(t88-t617).*1.0e-5;
et47 = t831.*(t653-t838).*2.769999999999999e-3+t1295.*(t653-t838).*9.999999999999998e-6;
et48 = t572.*t815.*8.8e-4-t604.*t831.*3.844e-2;
et49 = t815.*t831.*1.12e-3-t572.*(t88-t617).*3.844e-2;
et50 = t604.*(t86-t652).*8.8e-4-(t88-t617).*(t86-t652).*1.12e-3;
et51 = -t3289+t3365.*2.2e-4+t3526+t3644+t3655-t3661-t3664+t2654.*(t884+t1578-t2180+t14.*(t639-t1128-t2181+dq5.*t13.*(t86-t652))).*1.089e-2;
et52 = t3336.*(t8.*(t92-t663)+t15.*(t621-t864)).*2.9e-4;
et53 = -t2844-t2914-t2922+t3052+t3229-t3264+t3269+t3280-t3284+t3295+t3301+t3369+t3556-t3559+t3433.*(t614+t13.*(t86-t652)).*9.999999999999998e-6;
et54 = t2832.*(t639-t1128-t2181+dq5.*t13.*(t86-t652)).*9.999999999999998e-6+t2974.*(t92-t663).*9.999999999999998e-6;
et55 = t3422.*(t653-t838).*9.999999999999998e-6;
et56 = t2891+t2923+t2941+t3011-t3226+t3277-t3279-t3292+t3296-t3311+t3363+t3479.*1.0e-5+t3561+t3433.*(t614+t13.*(t86-t652)).*4.466636216449161e-20;
et57 = t2147.*(t639-t1128-t2181+dq5.*t13.*(t86-t652)).*2.840000000000012e-3+t2832.*(t639-t1128-t2181+dq5.*t13.*(t86-t652)).*4.466636216449161e-20;
et58 = t2974.*(t92-t663).*4.466636216449161e-20+t3422.*(t653-t838).*4.466636216449161e-20;
et59 = t831.*t1040.*8.8e-4-t815.*t1066.*1.144e-2;
et60 = t572.*t2163.*(-8.8e-4)+t572.*t2164.*1.144e-2;
et61 = t604.*t2147.*(-8.8e-4)+t604.*t2148.*1.144e-2;
et62 = t815.*t2147.*1.11e-3+t831.*t2164.*1.11e-3;
et63 = t1066.*(t88-t617).*8.8e-4-t1040.*(t86-t652).*1.144e-2;
et64 = t2148.*(t88-t617).*(-1.11e-3)-t2163.*(t86-t652).*1.11e-3;
et65 = t571.*t572.*(-7.000000000000001e-5)+t604.*t605.*7.000000000000001e-5;
et66 = t2.*t10.*t571.*4.999999999999997e-5+t9.*t10.*t572.*2.23e-3;
et67 = t2.*t10.*t604.*2.23e-3+t9.*t10.*t605.*4.999999999999997e-5;
et68 = t2000.*(t884+t1578-t2180+t14.*(t639-t1128-t2181+dq5.*t13.*(t86-t652))).*3.0e-5-t3312.*(t614+t13.*(t86-t652)).*5.000000000000004e-4;
et69 = t2832.*(t1386+t7.*(t88-t617)).*5.000000000000004e-4-t2000.*t2832.*5.0e-5;
et70 = t2035.*t2816.*5.0e-5+t2074.*t2816.*5.000000000000004e-4;
et71 = t2035.*t3312.*(-3.0e-5)-(t653-t838).*(t878-t1582+t2184+t7.*(t639-t1128-t2181+dq5.*t13.*(t86-t652))).*5.0e-5;
et72 = (t653-t838).*(t884+t1578-t2180+t14.*(t639-t1128-t2181+dq5.*t13.*(t86-t652))).*5.000000000000004e-4;
et73 = (t614+t13.*(t86-t652)).*(t1487+t2219-t2864+dq6.*t7.*(t88-t617)).*(-5.0e-5)+t2074.*(t1487+t2219-t2864+dq6.*t7.*(t88-t617)).*3.0e-5;
et74 = (t1386+t7.*(t88-t617)).*(t878-t1582+t2184+t7.*(t639-t1128-t2181+dq5.*t13.*(t86-t652))).*(-3.0e-5);
et75 = t3.*t23.*5.582083966615414e-19+t3.*t26.*5.582083966615414e-19+t10.*t23.*3.199999999999801e-4;
et76 = t10.*t26.*3.199999999999801e-4;
et77 = t231.*5.582083966615414e-19+t232.*5.582083966615414e-19+t622.*3.199999999999801e-4;
et78 = t688.*(-8.909980864224564e-21)+t701.*8.909980864224564e-21+t707.*3.199999999999801e-4;
et79 = t769.*8.909980864224564e-21+t770.*8.909980864224564e-21-t845.*3.199999999999801e-4;
et80 = t867.*3.199999999999801e-4-t873.*8.909980864224564e-21-t905.*8.909980864224564e-21;
et81 = t3.*t10.*t17.*1.781996172844913e-20;
et82 = -t3294+t3365.*7.950000000000001e-3+t3528+t3648+t3658-t3660-t3663+t2654.*(t884+t1578-t2180+t14.*(t639-t1128-t2181+dq5.*t13.*(t86-t652))).*2.2e-4;
et83 = t3336.*(t8.*(t92-t663)+t15.*(t621-t864)).*2.900000000000001e-4;
et84 = t281+t434+t740+t1386.*1.9738e-1-t1604.*3.466000000000001e-2-t2044.*3.466000000000001e-2+t2046.*2.324e-2;
et85 = t7.*(t88-t617).*1.9738e-1-t8.*(t653-t838).*2.324e-2;
et86 = t271+t428+t757+t860.*1.9738e-1-t1526.*1.9738e-1+t1635.*3.466000000000001e-2+t2080.*3.466000000000001e-2;
et87 = t2081.*(-2.324e-2)+t8.*(t614+t13.*(t86-t652)).*2.324e-2;
et88 = t39.*t571.*7.000000000000022e-5-t45.*t572.*7.000000000000001e-5;
et89 = t50.*t572.*(-7.000000000000001e-5)-t61.*t571.*7.000000000000022e-5;
et90 = t39.*t604.*(-7.000000000000001e-5)+t45.*t605.*7.000000000000022e-5;
et91 = t50.*t605.*7.000000000000022e-5+t61.*t604.*7.000000000000001e-5;
et92 = t604.*t1020.*(-7.299999999999999e-4)-t571.*t1066.*7.299999999999999e-4;
et93 = t572.*t1067.*(-7.299999999999999e-4)+t605.*t1040.*7.299999999999999e-4;
et94 = t9.*t10.*t1020.*7.000000000000022e-5+t2.*t10.*t1040.*7.000000000000001e-5;
et95 = t2.*t10.*t1067.*(-7.000000000000022e-5)+t9.*t10.*t1066.*7.000000000000001e-5;
et96 = t2000.*(t884+t1578-t2180+t14.*(t639-t1128-t2181+dq5.*t13.*(t86-t652))).*4.000000000000028e-5+t3312.*(t614+t13.*(t86-t652)).*5.0e-5;
et97 = t2832.*(t1386+t7.*(t88-t617)).*(-5.0e-5)+t2000.*t2832.*2.81e-3;
et98 = t2035.*t2816.*(-2.81e-3)-t2074.*t2816.*5.0e-5;
et99 = t2035.*t3312.*(-4.000000000000028e-5)+(t653-t838).*(t878-t1582+t2184+t7.*(t639-t1128-t2181+dq5.*t13.*(t86-t652))).*2.81e-3;
et100 = (t653-t838).*(t884+t1578-t2180+t14.*(t639-t1128-t2181+dq5.*t13.*(t86-t652))).*(-5.0e-5);
et101 = (t614+t13.*(t86-t652)).*(t1487+t2219-t2864+dq6.*t7.*(t88-t617)).*2.81e-3+t2074.*(t1487+t2219-t2864+dq6.*t7.*(t88-t617)).*4.000000000000028e-5;
et102 = (t1386+t7.*(t88-t617)).*(t878-t1582+t2184+t7.*(t639-t1128-t2181+dq5.*t13.*(t86-t652))).*(-4.000000000000028e-5);
et103 = t2000.*(t614+t13.*(t86-t652)).*(-5.0e-5)+t2035.*(t1386+t7.*(t88-t617)).*3.0e-5;
et104 = t2000.*t2074.*3.0e-5+t2035.*(t653-t838).*5.0e-5;
et105 = t2074.*(t653-t838).*5.000000000000004e-4+(t614+t13.*(t86-t652)).*(t1386+t7.*(t88-t617)).*5.000000000000004e-4;
et106 = t2163.*(t614+t13.*(t86-t652)).*1.0e-5+t2828.*(t614+t13.*(t86-t652)).*4.466636216449161e-20;
et107 = t1206.*t2147.*2.840000000000012e-3+t1295.*t2163.*2.840000000000012e-3;
et108 = t831.*t2816.*(-1.0e-5)+t831.*t2828.*2.840000000000012e-3;
et109 = t1206.*t2832.*(-4.466636216449161e-20)+t1295.*t2816.*4.466636216449161e-20;
et110 = (t88-t617).*(t639-t1128-t2181+dq5.*t13.*(t86-t652)).*2.840000000000012e-3-(t653-t838).*(t639-t1128-t2181+dq5.*t13.*(t86-t652)).*4.466636216449161e-20;
et111 = t2832.*(t88-t617).*(-1.0e-5)+t2147.*(t653-t838).*1.0e-5;
et112 = t2576.*(t884+t1578-t2180+t14.*(t639-t1128-t2181+dq5.*t13.*(t86-t652))).*2.900000000000001e-4;
et113 = t2601.*(t884+t1578-t2180+t14.*(t639-t1128-t2181+dq5.*t13.*(t86-t652))).*2.9e-4+t3619.*(t1386+t7.*(t88-t617)).*2.9e-4;
et114 = t3620.*(t1386+t7.*(t88-t617)).*(-2.900000000000001e-4)-t2074.*t3617.*2.900000000000001e-4;
et115 = t2074.*t3618.*2.9e-4-t2627.*t3312.*2.900000000000001e-4;
et116 = t2654.*t3312.*(-2.9e-4)-t2576.*t3619.*2.94e-3;
et117 = t2601.*t3620.*(-2.94e-3)+t2627.*t3618.*2.94e-3;
et118 = t2654.*t3617.*2.94e-3;
et119 = -t434+t653.*2.75e-2+t686-t838.*2.75e-2-t1374.*4.9e-4+t1386.*2.019e-2-t9.*t10.*(2.1e+1./5.0e+1);
et120 = t7.*(t88-t617).*2.019e-2+t14.*(t88-t617).*4.9e-4;
et121 = t39.*t571.*2.19e-3+t45.*t572.*4.999999999999997e-5;
et122 = t50.*t572.*4.999999999999997e-5-t61.*t571.*2.19e-3;
et123 = t39.*t604.*4.999999999999997e-5+t45.*t605.*2.19e-3;
et124 = t50.*t605.*2.19e-3-t61.*t604.*4.999999999999997e-5;
et125 = t604.*t1020.*(-7.000000000000022e-5)-t571.*t1066.*7.000000000000022e-5;
et126 = t572.*t1067.*(-7.000000000000022e-5)+t605.*t1040.*7.000000000000022e-5;
et127 = t9.*t10.*t1020.*2.19e-3-t2.*t10.*t1040.*4.999999999999997e-5;
et128 = t2.*t10.*t1067.*(-2.19e-3)-t9.*t10.*t1066.*4.999999999999997e-5;
et129 = t2163.*(t614+t13.*(t86-t652)).*2.769999999999999e-3-t2828.*(t614+t13.*(t86-t652)).*9.999999999999998e-6;
et130 = t1206.*t2147.*1.0e-5+t1295.*t2163.*1.0e-5;
et131 = t831.*t2816.*(-2.769999999999999e-3)+t831.*t2828.*1.0e-5;
et132 = t1206.*t2832.*9.999999999999998e-6-t1295.*t2816.*9.999999999999998e-6;
et133 = (t88-t617).*(t639-t1128-t2181+dq5.*t13.*(t86-t652)).*1.0e-5+(t653-t838).*(t639-t1128-t2181+dq5.*t13.*(t86-t652)).*9.999999999999998e-6;
et134 = t2832.*(t88-t617).*(-2.769999999999999e-3)+t2147.*(t653-t838).*2.769999999999999e-3;
et135 = t571.*t572.*7.000000000000022e-5-t604.*t605.*7.000000000000022e-5;
et136 = t2.*t10.*t571.*2.19e-3+t9.*t10.*t572.*4.999999999999997e-5;
et137 = t2.*t10.*t604.*4.999999999999997e-5+t9.*t10.*t605.*2.19e-3;
et138 = t2765+t2818-t2907+t3067+t3215+t3235-t3238-t3246+t3268-t3273+t3375+t3551-t3555+t3433.*(t614+t13.*(t86-t652)).*1.2e-4+t2147.*(t639-t1128-t2181+dq5.*t13.*(t86-t652)).*4.466636216449161e-20;
et139 = t2832.*(t639-t1128-t2181+dq5.*t13.*(t86-t652)).*1.2e-4+t2974.*(t92-t663).*1.2e-4;
et140 = t3422.*(t653-t838).*1.2e-4;
et141 = t2576.*(t884+t1578-t2180+t14.*(t639-t1128-t2181+dq5.*t13.*(t86-t652))).*2.2e-4;
et142 = t2601.*(t884+t1578-t2180+t14.*(t639-t1128-t2181+dq5.*t13.*(t86-t652))).*1.089e-2+t3619.*(t1386+t7.*(t88-t617)).*1.089e-2;
et143 = t3620.*(t1386+t7.*(t88-t617)).*(-2.2e-4)-t2074.*t3617.*2.2e-4;
et144 = t2074.*t3618.*1.089e-2-t2627.*t3312.*2.2e-4;
et145 = t2654.*t3312.*(-1.089e-2)-t2576.*t3619.*2.9e-4;
et146 = t2601.*t3620.*(-2.9e-4)+t2627.*t3618.*2.9e-4;
et147 = t2654.*t3617.*2.9e-4;
et148 = t32.*3.492e-2+t35.*2.25e-3-t73.*2.25e-3+t76.*3.492e-2;
et149 = t2.*t10.*3.9348e-1;
et150 = t29.*3.492e-2+t31.*2.25e-3+t77.*2.25e-3-t85.*3.492e-2;
et151 = t9.*t10.*(-3.9348e-1);
et152 = t231.*1.0e-4+t232.*1.0e-4;
et153 = t622.*5.582083966615414e-19-t688.*1.16152294893368e-19+t701.*1.16152294893368e-19;
et154 = t707.*5.582083966615414e-19+t769.*1.16152294893368e-19+t770.*1.16152294893368e-19;
et155 = t845.*(-5.582083966615414e-19)+t867.*5.582083966615414e-19-t873.*1.16152294893368e-19;
et156 = t905.*(-1.16152294893368e-19)+t3.*t10.*t17.*2.32304589786736e-19;
C = ft_8({dq1,dq2,dq3,dq4,dq5,dq6,dq7,et1,et10,et100,et101,et102,et103,et104,et105,et106,et107,et108,et109,et11,et110,et111,et112,et113,et114,et115,et116,et117,et118,et119,et12,et120,et121,et122,et123,et124,et125,et126,et127,et128,et129,et13,et130,et131,et132,et133,et134,et135,et136,et137,et138,et139,et14,et140,et141,et142,et143,et144,et145,et146,et147,et148,et149,et15,et150,et151,et152,et153,et154,et155,et156,et16,et17,et18,et19,et2,et20,et21,et22,et23,et24,et25,et26,et27,et28,et29,et3,et30,et31,et32,et33,et34,et35,et36,et37,et38,et39,et4,et40,et41,et42,et43,et44,et45,et46,et47,et48,et49,et5,et50,et51,et52,et53,et54,et55,et56,et57,et58,et59,et6,et60,et61,et62,et63,et64,et65,et66,et67,et68,et69,et7,et70,et71,et72,et73,et74,et75,et76,et77,et78,et79,et8,et80,et81,et82,et83,et84,et85,et86,et87,et88,et89,et9,et90,et91,et92,et93,et94,et95,et96,et97,et98,et99,t10,t1001,t1003,t1004,t1007,t1008,t1012,t1015,t1016,t1017,t1018,t1020,t1021,t1022,t1023,t1024,t1025,t1026,t1034,t1036,t1040,t1041,t1044,t105,t1051,t1052,t1053,t1054,t1055,t1056,t1058,t1059,t1060,t1066,t1067,t1069,t107,t1070,t1072,t1075,t1077,t1079,t1081,t1088,t1093,t1094,t1096,t1097,t11,t1110,t1113,t1114,t1115,t112,t1123,t1125,t1126,t1128,t1130,t1132,t1136,t1137,t1138,t114,t1142,t1143,t1146,t1159,t1161,t1172,t1174,t1175,t1177,t1178,t1179,t1189,t119,t1190,t12,t1206,t1207,t1209,t1211,t1212,t1213,t1214,t1215,t1217,t1218,t1219,t122,t1220,t1226,t1231,t1232,t1256,t1267,t1268,t1269,t1273,t1275,t1286,t1295,t1296,t1299,t13,t130,t1304,t1312,t1313,t1315,t1329,t1330,t1339,t1346,t1347,t1350,t1351,t1352,t1360,t1368,t1369,t137,t1374,t1375,t1386,t1387,t1389,t139,t1391,t14,t1423,t1424,t1431,t1435,t144,t1441,t1449,t1455,t1456,t1462,t1467,t1487,t1489,t149,t1497,t1498,t15,t1506,t151,t1513,t1515,t1516,t152,t1526,t1528,t1529,t1543,t1546,t1553,t1554,t1565,t1569,t1574,t1577,t1578,t1579,t1581,t1582,t1591,t16,t160,t1601,t1603,t1604,t1605,t1616,t1622,t1625,t1627,t1633,t1634,t1635,t1636,t1638,t1643,t1644,t1648,t1649,t165,t1654,t1655,t1657,t1658,t1660,t1661,t1662,t1667,t1668,t1672,t1675,t1679,t1681,t1682,t1685,t1686,t1687,t1688,t1697,t17,t1700,t1701,t1702,t1707,t171,t1710,t1711,t1715,t1717,t1718,t1719,t1720,t1721,t1723,t1725,t1726,t1729,t1732,t1734,t1735,t1736,t1737,t1738,t1740,t1742,t1743,t1745,t1746,t1748,t1749,t175,t1750,t1751,t1752,t1753,t1755,t1760,t1762,t1765,t1766,t1769,t1770,t1771,t1772,t1773,t1774,t1775,t1776,t1778,t1779,t1780,t1782,t1790,t1791,t1792,t1795,t1798,t1799,t180,t1800,t1801,t1802,t1804,t1805,t1806,t1811,t1812,t1813,t1814,t1816,t1817,t1819,t182,t1822,t1823,t1830,t1834,t1836,t1837,t1839,t1840,t1842,t1843,t1846,t1849,t185,t1850,t1851,t1852,t1853,t1855,t1856,t1859,t186,t1860,t1861,t1863,t1864,t1865,t1866,t1867,t187,t1871,t1872,t1873,t1874,t1875,t1876,t1880,t1881,t1883,t1885,t1886,t1888,t1889,t189,t1890,t1892,t1893,t1896,t1898,t1901,t1902,t1903,t1905,t1907,t1908,t1909,t1911,t1912,t1913,t1914,t1917,t1918,t1919,t1924,t1927,t1928,t1931,t1932,t1934,t1940,t1942,t1944,t1945,t1949,t1950,t1951,t1952,t1953,t1955,t1957,t1959,t1960,t1962,t1963,t1969,t1970,t1974,t1976,t1980,t1984,t1985,t1986,t1993,t2,t2000,t2001,t2002,t2003,t2006,t2008,t2009,t2010,t2011,t2018,t2022,t2026,t2029,t2033,t2034,t2035,t2036,t2041,t2042,t2044,t2045,t2046,t2049,t2051,t2054,t2056,t2058,t2060,t2065,t2066,t2071,t2072,t2073,t2074,t2075,t2076,t208,t2080,t2081,t2085,t2088,t2089,t2090,t2095,t2096,t2108,t2109,t2111,t2115,t2119,t2125,t2130,t2139,t2147,t2148,t2149,t2151,t2152,t2163,t2164,t2165,t2171,t2173,t2177,t2179,t2180,t2181,t2182,t2183,t2184,t2187,t2196,t2198,t2203,t2205,t2206,t2207,t2208,t221,t2212,t2215,t2217,t2219,t2220,t2224,t2227,t2228,t223,t2231,t2240,t2246,t2253,t2256,t2258,t2259,t2261,t2262,t2263,t2264,t2266,t2269,t2289,t2296,t23,t230,t2300,t2301,t231,t2315,t232,t2323,t2326,t2330,t234,t2341,t2343,t235,t2350,t2351,t2352,t2355,t2356,t2357,t2358,t2359,t236,t2360,t2362,t2363,t2365,t2366,t2367,t2369,t237,t2370,t2371,t2372,t2374,t2375,t2376,t2379,t238,t2380,t2382,t2383,t2384,t2385,t2387,t2388,t239,t2392,t2393,t2395,t2399,t24,t240,t2400,t2402,t2404,t2407,t241,t2411,t2418,t242,t2429,t243,t2435,t2439,t244,t2443,t2444,t2445,t2447,t2455,t2456,t2460,t2462,t2463,t2464,t2466,t2467,t2471,t2473,t2477,t2482,t2483,t2488,t2494,t2496,t25,t250,t2501,t2503,t2507,t251,t2513,t2514,t2516,t252,t2521,t2522,t2523,t253,t2533,t2534,t2536,t2537,t254,t2541,t2554,t2558,t2560,t2561,t2563,t2569,t2570,t2571,t2576,t258,t2581,t2584,t2585,t2587,t259,t2590,t2591,t26,t2601,t2602,t2604,t2609,t2610,t2611,t2612,t2613,t2614,t2615,t2617,t2618,t2620,t2621,t2622,t2624,t2627,t2630,t2631,t2634,t2635,t2637,t2638,t2640,t2641,t2642,t2643,t2647,t2648,t2651,t2652,t2653,t2654,t2655,t2656,t2659,t2661,t2662,t2663,t2664,t2665,t2666,t2667,t267,t2670,t2671,t2672,t2674,t2675,t2677,t2679,t268,t2680,t2681,t2684,t2685,t2687,t2689,t269,t2690,t2691,t2692,t2693,t2694,t2697,t2698,t2699,t27,t270,t2700,t2701,t2703,t2707,t2708,t271,t2710,t2711,t2714,t2717,t2718,t272,t2720,t2721,t2722,t2723,t2726,t2727,t2728,t2729,t273,t2732,t2734,t2735,t2737,t2738,t2739,t274,t2740,t2741,t2742,t2743,t2744,t2747,t275,t2751,t2753,t2754,t2756,t276,t2765,t277,t2776,t2780,t2781,t2783,t2788,t2789,t279,t2790,t2791,t2792,t2794,t2795,t2796,t2797,t2798,t2799,t28,t280,t2801,t2803,t2804,t2807,t2810,t2811,t2813,t2814,t2816,t2817,t2818,t282,t2823,t2825,t2827,t2828,t2829,t283,t2832,t2837,t2838,t2839,t284,t2840,t2841,t2842,t2844,t285,t2854,t2857,t286,t2861,t2864,t2868,t287,t288,t2883,t2884,t289,t2891,t2897,t29,t290,t2900,t2907,t2914,t2922,t2923,t2924,t2925,t293,t2930,t2931,t2935,t2936,t2939,t2941,t2942,t2943,t2944,t2945,t2946,t2948,t2949,t295,t2950,t2953,t2954,t2955,t2956,t2957,t296,t2960,t2961,t2962,t297,t2972,t2974,t298,t2989,t2991,t2996,t2997,t2998,t2999,t3,t30,t3008,t3009,t301,t3011,t3020,t3031,t3035,t3038,t3039,t3040,t3041,t3042,t3045,t3047,t3048,t3051,t3052,t3060,t3066,t3067,t307,t3071,t3075,t3076,t308,t3082,t3083,t3085,t3086,t3088,t309,t3092,t3097,t3098,t3099,t31,t310,t3104,t3106,t3107,t311,t3112,t3113,t312,t3120,t3121,t3122,t3124,t3126,t3128,t3129,t313,t3130,t3131,t3132,t3133,t3140,t3141,t3142,t3143,t3148,t3152,t3153,t3154,t3155,t3159,t3161,t3162,t3163,t3165,t3166,t3168,t317,t3170,t3171,t3172,t3175,t3179,t318,t3181,t3186,t319,t3190,t3192,t3193,t3194,t3195,t3196,t32,t320,t3201,t3202,t3203,t3204,t3205,t3206,t3210,t3215,t3226,t3229,t3232,t3235,t3238,t3246,t3248,t3249,t3252,t3253,t3255,t3257,t3260,t3261,t3262,t3263,t3264,t3268,t3269,t327,t3272,t3273,t3277,t3279,t328,t3280,t3284,t3285,t3286,t3287,t3288,t3289,t329,t3290,t3291,t3292,t3293,t3294,t3295,t3296,t33,t330,t3301,t331,t3311,t3312,t3313,t3315,t3316,t3321,t3324,t3336,t3340,t3342,t3356,t3357,t3358,t3359,t3360,t3361,t3362,t3363,t3364,t3365,t3366,t3369,t3372,t3375,t3377,t338,t3382,t3384,t3386,t3388,t3392,t3393,t3394,t3395,t3397,t3398,t3399,t34,t3400,t3402,t3403,t3406,t3407,t3411,t3413,t3414,t3417,t3418,t342,t3421,t3422,t3424,t3426,t3429,t3433,t3436,t3437,t3438,t3440,t3443,t3444,t3452,t346,t3460,t3464,t3465,t3468,t3470,t3476,t3479,t3480,t3481,t3482,t3483,t3486,t3488,t3489,t349,t3490,t3491,t3492,t3495,t3498,t35,t3502,t3504,t3506,t3514,t3526,t3527,t3528,t3535,t3536,t3537,t3538,t3540,t3542,t3544,t3546,t3547,t3551,t3555,t3556,t3559,t3561,t36,t3610,t3617,t3618,t3619,t3620,t3625,t3626,t3627,t3628,t3640,t3641,t3642,t3643,t3644,t3645,t3646,t3648,t3649,t3651,t3652,t3653,t3654,t3655,t3658,t3660,t3661,t3662,t3663,t3664,t3665,t3666,t3667,t3668,t3669,t3670,t3671,t3672,t3673,t3674,t3679,t3685,t37,t3720,t3751,t3776,t3779,t3780,t3781,t3782,t3783,t3784,t3786,t3788,t3789,t3790,t3796,t3798,t3811,t3812,t3816,t3818,t3820,t3821,t3823,t3824,t3825,t3826,t3828,t3829,t3833,t3835,t3838,t3839,t3840,t3841,t3842,t3843,t3844,t3845,t39,t4,t40,t427,t428,t429,t43,t431,t433,t435,t436,t439,t441,t444,t448,t45,t450,t451,t452,t453,t455,t456,t457,t458,t459,t46,t460,t461,t463,t465,t466,t469,t49,t494,t5,t50,t51,t510,t512,t515,t516,t517,t518,t522,t523,t524,t525,t526,t527,t528,t529,t530,t535,t536,t537,t538,t542,t547,t548,t55,t553,t554,t556,t561,t562,t563,t564,t565,t566,t567,t568,t569,t57,t570,t571,t572,t573,t574,t58,t580,t581,t583,t594,t595,t596,t6,t600,t601,t602,t603,t604,t605,t606,t607,t608,t609,t61,t612,t613,t614,t615,t616,t617,t618,t619,t620,t621,t622,t624,t626,t629,t63,t631,t632,t633,t634,t635,t637,t639,t64,t640,t642,t643,t644,t646,t647,t648,t649,t650,t651,t652,t653,t654,t656,t657,t658,t660,t661,t662,t663,t664,t665,t667,t67,t673,t676,t677,t678,t685,t687,t688,t689,t69,t691,t692,t693,t694,t696,t697,t698,t7,t70,t701,t702,t703,t704,t705,t707,t708,t71,t72,t721,t722,t723,t724,t725,t726,t728,t729,t73,t730,t731,t735,t74,t743,t75,t754,t755,t756,t757,t76,t760,t762,t769,t77,t770,t773,t774,t776,t777,t778,t78,t785,t786,t787,t788,t79,t791,t792,t795,t796,t797,t8,t80,t800,t805,t806,t81,t813,t815,t817,t818,t819,t82,t827,t83,t831,t834,t835,t836,t837,t838,t839,t84,t840,t841,t842,t843,t845,t846,t847,t85,t853,t854,t855,t856,t857,t859,t86,t860,t863,t864,t866,t867,t87,t870,t871,t873,t876,t877,t878,t88,t880,t881,t882,t884,t885,t888,t889,t89,t890,t891,t896,t898,t899,t9,t90,t900,t902,t905,t907,t908,t91,t911,t92,t921,t926,t927,t928,t930,t932,t933,t935,t939,t94,t940,t942,t948,t949,t952,t958,t959,t966,t969,t97,t972,t973,t974,t975,t982,t983,t984,t987,t988,t992,t994});
end
function C = ft_8(ct)
dq1 = ct{1};
dq2 = ct{2};
dq3 = ct{3};
dq4 = ct{4};
dq5 = ct{5};
dq6 = ct{6};
dq7 = ct{7};
et1 = ct{8};
et10 = ct{9};
et100 = ct{10};
et101 = ct{11};
et102 = ct{12};
et103 = ct{13};
et104 = ct{14};
et105 = ct{15};
et106 = ct{16};
et107 = ct{17};
et108 = ct{18};
et109 = ct{19};
et11 = ct{20};
et110 = ct{21};
et111 = ct{22};
et112 = ct{23};
et113 = ct{24};
et114 = ct{25};
et115 = ct{26};
et116 = ct{27};
et117 = ct{28};
et118 = ct{29};
et119 = ct{30};
et12 = ct{31};
et120 = ct{32};
et121 = ct{33};
et122 = ct{34};
et123 = ct{35};
et124 = ct{36};
et125 = ct{37};
et126 = ct{38};
et127 = ct{39};
et128 = ct{40};
et129 = ct{41};
et13 = ct{42};
et130 = ct{43};
et131 = ct{44};
et132 = ct{45};
et133 = ct{46};
et134 = ct{47};
et135 = ct{48};
et136 = ct{49};
et137 = ct{50};
et138 = ct{51};
et139 = ct{52};
et14 = ct{53};
et140 = ct{54};
et141 = ct{55};
et142 = ct{56};
et143 = ct{57};
et144 = ct{58};
et145 = ct{59};
et146 = ct{60};
et147 = ct{61};
et148 = ct{62};
et149 = ct{63};
et15 = ct{64};
et150 = ct{65};
et151 = ct{66};
et152 = ct{67};
et153 = ct{68};
et154 = ct{69};
et155 = ct{70};
et156 = ct{71};
et16 = ct{72};
et17 = ct{73};
et18 = ct{74};
et19 = ct{75};
et2 = ct{76};
et20 = ct{77};
et21 = ct{78};
et22 = ct{79};
et23 = ct{80};
et24 = ct{81};
et25 = ct{82};
et26 = ct{83};
et27 = ct{84};
et28 = ct{85};
et29 = ct{86};
et3 = ct{87};
et30 = ct{88};
et31 = ct{89};
et32 = ct{90};
et33 = ct{91};
et34 = ct{92};
et35 = ct{93};
et36 = ct{94};
et37 = ct{95};
et38 = ct{96};
et39 = ct{97};
et4 = ct{98};
et40 = ct{99};
et41 = ct{100};
et42 = ct{101};
et43 = ct{102};
et44 = ct{103};
et45 = ct{104};
et46 = ct{105};
et47 = ct{106};
et48 = ct{107};
et49 = ct{108};
et5 = ct{109};
et50 = ct{110};
et51 = ct{111};
et52 = ct{112};
et53 = ct{113};
et54 = ct{114};
et55 = ct{115};
et56 = ct{116};
et57 = ct{117};
et58 = ct{118};
et59 = ct{119};
et6 = ct{120};
et60 = ct{121};
et61 = ct{122};
et62 = ct{123};
et63 = ct{124};
et64 = ct{125};
et65 = ct{126};
et66 = ct{127};
et67 = ct{128};
et68 = ct{129};
et69 = ct{130};
et7 = ct{131};
et70 = ct{132};
et71 = ct{133};
et72 = ct{134};
et73 = ct{135};
et74 = ct{136};
et75 = ct{137};
et76 = ct{138};
et77 = ct{139};
et78 = ct{140};
et79 = ct{141};
et8 = ct{142};
et80 = ct{143};
et81 = ct{144};
et82 = ct{145};
et83 = ct{146};
et84 = ct{147};
et85 = ct{148};
et86 = ct{149};
et87 = ct{150};
et88 = ct{151};
et89 = ct{152};
et9 = ct{153};
et90 = ct{154};
et91 = ct{155};
et92 = ct{156};
et93 = ct{157};
et94 = ct{158};
et95 = ct{159};
et96 = ct{160};
et97 = ct{161};
et98 = ct{162};
et99 = ct{163};
t10 = ct{164};
t1001 = ct{165};
t1003 = ct{166};
t1004 = ct{167};
t1007 = ct{168};
t1008 = ct{169};
t1012 = ct{170};
t1015 = ct{171};
t1016 = ct{172};
t1017 = ct{173};
t1018 = ct{174};
t1020 = ct{175};
t1021 = ct{176};
t1022 = ct{177};
t1023 = ct{178};
t1024 = ct{179};
t1025 = ct{180};
t1026 = ct{181};
t1034 = ct{182};
t1036 = ct{183};
t1040 = ct{184};
t1041 = ct{185};
t1044 = ct{186};
t105 = ct{187};
t1051 = ct{188};
t1052 = ct{189};
t1053 = ct{190};
t1054 = ct{191};
t1055 = ct{192};
t1056 = ct{193};
t1058 = ct{194};
t1059 = ct{195};
t1060 = ct{196};
t1066 = ct{197};
t1067 = ct{198};
t1069 = ct{199};
t107 = ct{200};
t1070 = ct{201};
t1072 = ct{202};
t1075 = ct{203};
t1077 = ct{204};
t1079 = ct{205};
t1081 = ct{206};
t1088 = ct{207};
t1093 = ct{208};
t1094 = ct{209};
t1096 = ct{210};
t1097 = ct{211};
t11 = ct{212};
t1110 = ct{213};
t1113 = ct{214};
t1114 = ct{215};
t1115 = ct{216};
t112 = ct{217};
t1123 = ct{218};
t1125 = ct{219};
t1126 = ct{220};
t1128 = ct{221};
t1130 = ct{222};
t1132 = ct{223};
t1136 = ct{224};
t1137 = ct{225};
t1138 = ct{226};
t114 = ct{227};
t1142 = ct{228};
t1143 = ct{229};
t1146 = ct{230};
t1159 = ct{231};
t1161 = ct{232};
t1172 = ct{233};
t1174 = ct{234};
t1175 = ct{235};
t1177 = ct{236};
t1178 = ct{237};
t1179 = ct{238};
t1189 = ct{239};
t119 = ct{240};
t1190 = ct{241};
t12 = ct{242};
t1206 = ct{243};
t1207 = ct{244};
t1209 = ct{245};
t1211 = ct{246};
t1212 = ct{247};
t1213 = ct{248};
t1214 = ct{249};
t1215 = ct{250};
t1217 = ct{251};
t1218 = ct{252};
t1219 = ct{253};
t122 = ct{254};
t1220 = ct{255};
t1226 = ct{256};
t1231 = ct{257};
t1232 = ct{258};
t1256 = ct{259};
t1267 = ct{260};
t1268 = ct{261};
t1269 = ct{262};
t1273 = ct{263};
t1275 = ct{264};
t1286 = ct{265};
t1295 = ct{266};
t1296 = ct{267};
t1299 = ct{268};
t13 = ct{269};
t130 = ct{270};
t1304 = ct{271};
t1312 = ct{272};
t1313 = ct{273};
t1315 = ct{274};
t1329 = ct{275};
t1330 = ct{276};
t1339 = ct{277};
t1346 = ct{278};
t1347 = ct{279};
t1350 = ct{280};
t1351 = ct{281};
t1352 = ct{282};
t1360 = ct{283};
t1368 = ct{284};
t1369 = ct{285};
t137 = ct{286};
t1374 = ct{287};
t1375 = ct{288};
t1386 = ct{289};
t1387 = ct{290};
t1389 = ct{291};
t139 = ct{292};
t1391 = ct{293};
t14 = ct{294};
t1423 = ct{295};
t1424 = ct{296};
t1431 = ct{297};
t1435 = ct{298};
t144 = ct{299};
t1441 = ct{300};
t1449 = ct{301};
t1455 = ct{302};
t1456 = ct{303};
t1462 = ct{304};
t1467 = ct{305};
t1487 = ct{306};
t1489 = ct{307};
t149 = ct{308};
t1497 = ct{309};
t1498 = ct{310};
t15 = ct{311};
t1506 = ct{312};
t151 = ct{313};
t1513 = ct{314};
t1515 = ct{315};
t1516 = ct{316};
t152 = ct{317};
t1526 = ct{318};
t1528 = ct{319};
t1529 = ct{320};
t1543 = ct{321};
t1546 = ct{322};
t1553 = ct{323};
t1554 = ct{324};
t1565 = ct{325};
t1569 = ct{326};
t1574 = ct{327};
t1577 = ct{328};
t1578 = ct{329};
t1579 = ct{330};
t1581 = ct{331};
t1582 = ct{332};
t1591 = ct{333};
t16 = ct{334};
t160 = ct{335};
t1601 = ct{336};
t1603 = ct{337};
t1604 = ct{338};
t1605 = ct{339};
t1616 = ct{340};
t1622 = ct{341};
t1625 = ct{342};
t1627 = ct{343};
t1633 = ct{344};
t1634 = ct{345};
t1635 = ct{346};
t1636 = ct{347};
t1638 = ct{348};
t1643 = ct{349};
t1644 = ct{350};
t1648 = ct{351};
t1649 = ct{352};
t165 = ct{353};
t1654 = ct{354};
t1655 = ct{355};
t1657 = ct{356};
t1658 = ct{357};
t1660 = ct{358};
t1661 = ct{359};
t1662 = ct{360};
t1667 = ct{361};
t1668 = ct{362};
t1672 = ct{363};
t1675 = ct{364};
t1679 = ct{365};
t1681 = ct{366};
t1682 = ct{367};
t1685 = ct{368};
t1686 = ct{369};
t1687 = ct{370};
t1688 = ct{371};
t1697 = ct{372};
t17 = ct{373};
t1700 = ct{374};
t1701 = ct{375};
t1702 = ct{376};
t1707 = ct{377};
t171 = ct{378};
t1710 = ct{379};
t1711 = ct{380};
t1715 = ct{381};
t1717 = ct{382};
t1718 = ct{383};
t1719 = ct{384};
t1720 = ct{385};
t1721 = ct{386};
t1723 = ct{387};
t1725 = ct{388};
t1726 = ct{389};
t1729 = ct{390};
t1732 = ct{391};
t1734 = ct{392};
t1735 = ct{393};
t1736 = ct{394};
t1737 = ct{395};
t1738 = ct{396};
t1740 = ct{397};
t1742 = ct{398};
t1743 = ct{399};
t1745 = ct{400};
t1746 = ct{401};
t1748 = ct{402};
t1749 = ct{403};
t175 = ct{404};
t1750 = ct{405};
t1751 = ct{406};
t1752 = ct{407};
t1753 = ct{408};
t1755 = ct{409};
t1760 = ct{410};
t1762 = ct{411};
t1765 = ct{412};
t1766 = ct{413};
t1769 = ct{414};
t1770 = ct{415};
t1771 = ct{416};
t1772 = ct{417};
t1773 = ct{418};
t1774 = ct{419};
t1775 = ct{420};
t1776 = ct{421};
t1778 = ct{422};
t1779 = ct{423};
t1780 = ct{424};
t1782 = ct{425};
t1790 = ct{426};
t1791 = ct{427};
t1792 = ct{428};
t1795 = ct{429};
t1798 = ct{430};
t1799 = ct{431};
t180 = ct{432};
t1800 = ct{433};
t1801 = ct{434};
t1802 = ct{435};
t1804 = ct{436};
t1805 = ct{437};
t1806 = ct{438};
t1811 = ct{439};
t1812 = ct{440};
t1813 = ct{441};
t1814 = ct{442};
t1816 = ct{443};
t1817 = ct{444};
t1819 = ct{445};
t182 = ct{446};
t1822 = ct{447};
t1823 = ct{448};
t1830 = ct{449};
t1834 = ct{450};
t1836 = ct{451};
t1837 = ct{452};
t1839 = ct{453};
t1840 = ct{454};
t1842 = ct{455};
t1843 = ct{456};
t1846 = ct{457};
t1849 = ct{458};
t185 = ct{459};
t1850 = ct{460};
t1851 = ct{461};
t1852 = ct{462};
t1853 = ct{463};
t1855 = ct{464};
t1856 = ct{465};
t1859 = ct{466};
t186 = ct{467};
t1860 = ct{468};
t1861 = ct{469};
t1863 = ct{470};
t1864 = ct{471};
t1865 = ct{472};
t1866 = ct{473};
t1867 = ct{474};
t187 = ct{475};
t1871 = ct{476};
t1872 = ct{477};
t1873 = ct{478};
t1874 = ct{479};
t1875 = ct{480};
t1876 = ct{481};
t1880 = ct{482};
t1881 = ct{483};
t1883 = ct{484};
t1885 = ct{485};
t1886 = ct{486};
t1888 = ct{487};
t1889 = ct{488};
t189 = ct{489};
t1890 = ct{490};
t1892 = ct{491};
t1893 = ct{492};
t1896 = ct{493};
t1898 = ct{494};
t1901 = ct{495};
t1902 = ct{496};
t1903 = ct{497};
t1905 = ct{498};
t1907 = ct{499};
t1908 = ct{500};
t1909 = ct{501};
t1911 = ct{502};
t1912 = ct{503};
t1913 = ct{504};
t1914 = ct{505};
t1917 = ct{506};
t1918 = ct{507};
t1919 = ct{508};
t1924 = ct{509};
t1927 = ct{510};
t1928 = ct{511};
t1931 = ct{512};
t1932 = ct{513};
t1934 = ct{514};
t1940 = ct{515};
t1942 = ct{516};
t1944 = ct{517};
t1945 = ct{518};
t1949 = ct{519};
t1950 = ct{520};
t1951 = ct{521};
t1952 = ct{522};
t1953 = ct{523};
t1955 = ct{524};
t1957 = ct{525};
t1959 = ct{526};
t1960 = ct{527};
t1962 = ct{528};
t1963 = ct{529};
t1969 = ct{530};
t1970 = ct{531};
t1974 = ct{532};
t1976 = ct{533};
t1980 = ct{534};
t1984 = ct{535};
t1985 = ct{536};
t1986 = ct{537};
t1993 = ct{538};
t2 = ct{539};
t2000 = ct{540};
t2001 = ct{541};
t2002 = ct{542};
t2003 = ct{543};
t2006 = ct{544};
t2008 = ct{545};
t2009 = ct{546};
t2010 = ct{547};
t2011 = ct{548};
t2018 = ct{549};
t2022 = ct{550};
t2026 = ct{551};
t2029 = ct{552};
t2033 = ct{553};
t2034 = ct{554};
t2035 = ct{555};
t2036 = ct{556};
t2041 = ct{557};
t2042 = ct{558};
t2044 = ct{559};
t2045 = ct{560};
t2046 = ct{561};
t2049 = ct{562};
t2051 = ct{563};
t2054 = ct{564};
t2056 = ct{565};
t2058 = ct{566};
t2060 = ct{567};
t2065 = ct{568};
t2066 = ct{569};
t2071 = ct{570};
t2072 = ct{571};
t2073 = ct{572};
t2074 = ct{573};
t2075 = ct{574};
t2076 = ct{575};
t208 = ct{576};
t2080 = ct{577};
t2081 = ct{578};
t2085 = ct{579};
t2088 = ct{580};
t2089 = ct{581};
t2090 = ct{582};
t2095 = ct{583};
t2096 = ct{584};
t2108 = ct{585};
t2109 = ct{586};
t2111 = ct{587};
t2115 = ct{588};
t2119 = ct{589};
t2125 = ct{590};
t2130 = ct{591};
t2139 = ct{592};
t2147 = ct{593};
t2148 = ct{594};
t2149 = ct{595};
t2151 = ct{596};
t2152 = ct{597};
t2163 = ct{598};
t2164 = ct{599};
t2165 = ct{600};
t2171 = ct{601};
t2173 = ct{602};
t2177 = ct{603};
t2179 = ct{604};
t2180 = ct{605};
t2181 = ct{606};
t2182 = ct{607};
t2183 = ct{608};
t2184 = ct{609};
t2187 = ct{610};
t2196 = ct{611};
t2198 = ct{612};
t2203 = ct{613};
t2205 = ct{614};
t2206 = ct{615};
t2207 = ct{616};
t2208 = ct{617};
t221 = ct{618};
t2212 = ct{619};
t2215 = ct{620};
t2217 = ct{621};
t2219 = ct{622};
t2220 = ct{623};
t2224 = ct{624};
t2227 = ct{625};
t2228 = ct{626};
t223 = ct{627};
t2231 = ct{628};
t2240 = ct{629};
t2246 = ct{630};
t2253 = ct{631};
t2256 = ct{632};
t2258 = ct{633};
t2259 = ct{634};
t2261 = ct{635};
t2262 = ct{636};
t2263 = ct{637};
t2264 = ct{638};
t2266 = ct{639};
t2269 = ct{640};
t2289 = ct{641};
t2296 = ct{642};
t23 = ct{643};
t230 = ct{644};
t2300 = ct{645};
t2301 = ct{646};
t231 = ct{647};
t2315 = ct{648};
t232 = ct{649};
t2323 = ct{650};
t2326 = ct{651};
t2330 = ct{652};
t234 = ct{653};
t2341 = ct{654};
t2343 = ct{655};
t235 = ct{656};
t2350 = ct{657};
t2351 = ct{658};
t2352 = ct{659};
t2355 = ct{660};
t2356 = ct{661};
t2357 = ct{662};
t2358 = ct{663};
t2359 = ct{664};
t236 = ct{665};
t2360 = ct{666};
t2362 = ct{667};
t2363 = ct{668};
t2365 = ct{669};
t2366 = ct{670};
t2367 = ct{671};
t2369 = ct{672};
t237 = ct{673};
t2370 = ct{674};
t2371 = ct{675};
t2372 = ct{676};
t2374 = ct{677};
t2375 = ct{678};
t2376 = ct{679};
t2379 = ct{680};
t238 = ct{681};
t2380 = ct{682};
t2382 = ct{683};
t2383 = ct{684};
t2384 = ct{685};
t2385 = ct{686};
t2387 = ct{687};
t2388 = ct{688};
t239 = ct{689};
t2392 = ct{690};
t2393 = ct{691};
t2395 = ct{692};
t2399 = ct{693};
t24 = ct{694};
t240 = ct{695};
t2400 = ct{696};
t2402 = ct{697};
t2404 = ct{698};
t2407 = ct{699};
t241 = ct{700};
t2411 = ct{701};
t2418 = ct{702};
t242 = ct{703};
t2429 = ct{704};
t243 = ct{705};
t2435 = ct{706};
t2439 = ct{707};
t244 = ct{708};
t2443 = ct{709};
t2444 = ct{710};
t2445 = ct{711};
t2447 = ct{712};
t2455 = ct{713};
t2456 = ct{714};
t2460 = ct{715};
t2462 = ct{716};
t2463 = ct{717};
t2464 = ct{718};
t2466 = ct{719};
t2467 = ct{720};
t2471 = ct{721};
t2473 = ct{722};
t2477 = ct{723};
t2482 = ct{724};
t2483 = ct{725};
t2488 = ct{726};
t2494 = ct{727};
t2496 = ct{728};
t25 = ct{729};
t250 = ct{730};
t2501 = ct{731};
t2503 = ct{732};
t2507 = ct{733};
t251 = ct{734};
t2513 = ct{735};
t2514 = ct{736};
t2516 = ct{737};
t252 = ct{738};
t2521 = ct{739};
t2522 = ct{740};
t2523 = ct{741};
t253 = ct{742};
t2533 = ct{743};
t2534 = ct{744};
t2536 = ct{745};
t2537 = ct{746};
t254 = ct{747};
t2541 = ct{748};
t2554 = ct{749};
t2558 = ct{750};
t2560 = ct{751};
t2561 = ct{752};
t2563 = ct{753};
t2569 = ct{754};
t2570 = ct{755};
t2571 = ct{756};
t2576 = ct{757};
t258 = ct{758};
t2581 = ct{759};
t2584 = ct{760};
t2585 = ct{761};
t2587 = ct{762};
t259 = ct{763};
t2590 = ct{764};
t2591 = ct{765};
t26 = ct{766};
t2601 = ct{767};
t2602 = ct{768};
t2604 = ct{769};
t2609 = ct{770};
t2610 = ct{771};
t2611 = ct{772};
t2612 = ct{773};
t2613 = ct{774};
t2614 = ct{775};
t2615 = ct{776};
t2617 = ct{777};
t2618 = ct{778};
t2620 = ct{779};
t2621 = ct{780};
t2622 = ct{781};
t2624 = ct{782};
t2627 = ct{783};
t2630 = ct{784};
t2631 = ct{785};
t2634 = ct{786};
t2635 = ct{787};
t2637 = ct{788};
t2638 = ct{789};
t2640 = ct{790};
t2641 = ct{791};
t2642 = ct{792};
t2643 = ct{793};
t2647 = ct{794};
t2648 = ct{795};
t2651 = ct{796};
t2652 = ct{797};
t2653 = ct{798};
t2654 = ct{799};
t2655 = ct{800};
t2656 = ct{801};
t2659 = ct{802};
t2661 = ct{803};
t2662 = ct{804};
t2663 = ct{805};
t2664 = ct{806};
t2665 = ct{807};
t2666 = ct{808};
t2667 = ct{809};
t267 = ct{810};
t2670 = ct{811};
t2671 = ct{812};
t2672 = ct{813};
t2674 = ct{814};
t2675 = ct{815};
t2677 = ct{816};
t2679 = ct{817};
t268 = ct{818};
t2680 = ct{819};
t2681 = ct{820};
t2684 = ct{821};
t2685 = ct{822};
t2687 = ct{823};
t2689 = ct{824};
t269 = ct{825};
t2690 = ct{826};
t2691 = ct{827};
t2692 = ct{828};
t2693 = ct{829};
t2694 = ct{830};
t2697 = ct{831};
t2698 = ct{832};
t2699 = ct{833};
t27 = ct{834};
t270 = ct{835};
t2700 = ct{836};
t2701 = ct{837};
t2703 = ct{838};
t2707 = ct{839};
t2708 = ct{840};
t271 = ct{841};
t2710 = ct{842};
t2711 = ct{843};
t2714 = ct{844};
t2717 = ct{845};
t2718 = ct{846};
t272 = ct{847};
t2720 = ct{848};
t2721 = ct{849};
t2722 = ct{850};
t2723 = ct{851};
t2726 = ct{852};
t2727 = ct{853};
t2728 = ct{854};
t2729 = ct{855};
t273 = ct{856};
t2732 = ct{857};
t2734 = ct{858};
t2735 = ct{859};
t2737 = ct{860};
t2738 = ct{861};
t2739 = ct{862};
t274 = ct{863};
t2740 = ct{864};
t2741 = ct{865};
t2742 = ct{866};
t2743 = ct{867};
t2744 = ct{868};
t2747 = ct{869};
t275 = ct{870};
t2751 = ct{871};
t2753 = ct{872};
t2754 = ct{873};
t2756 = ct{874};
t276 = ct{875};
t2765 = ct{876};
t277 = ct{877};
t2776 = ct{878};
t2780 = ct{879};
t2781 = ct{880};
t2783 = ct{881};
t2788 = ct{882};
t2789 = ct{883};
t279 = ct{884};
t2790 = ct{885};
t2791 = ct{886};
t2792 = ct{887};
t2794 = ct{888};
t2795 = ct{889};
t2796 = ct{890};
t2797 = ct{891};
t2798 = ct{892};
t2799 = ct{893};
t28 = ct{894};
t280 = ct{895};
t2801 = ct{896};
t2803 = ct{897};
t2804 = ct{898};
t2807 = ct{899};
t2810 = ct{900};
t2811 = ct{901};
t2813 = ct{902};
t2814 = ct{903};
t2816 = ct{904};
t2817 = ct{905};
t2818 = ct{906};
t282 = ct{907};
t2823 = ct{908};
t2825 = ct{909};
t2827 = ct{910};
t2828 = ct{911};
t2829 = ct{912};
t283 = ct{913};
t2832 = ct{914};
t2837 = ct{915};
t2838 = ct{916};
t2839 = ct{917};
t284 = ct{918};
t2840 = ct{919};
t2841 = ct{920};
t2842 = ct{921};
t2844 = ct{922};
t285 = ct{923};
t2854 = ct{924};
t2857 = ct{925};
t286 = ct{926};
t2861 = ct{927};
t2864 = ct{928};
t2868 = ct{929};
t287 = ct{930};
t288 = ct{931};
t2883 = ct{932};
t2884 = ct{933};
t289 = ct{934};
t2891 = ct{935};
t2897 = ct{936};
t29 = ct{937};
t290 = ct{938};
t2900 = ct{939};
t2907 = ct{940};
t2914 = ct{941};
t2922 = ct{942};
t2923 = ct{943};
t2924 = ct{944};
t2925 = ct{945};
t293 = ct{946};
t2930 = ct{947};
t2931 = ct{948};
t2935 = ct{949};
t2936 = ct{950};
t2939 = ct{951};
t2941 = ct{952};
t2942 = ct{953};
t2943 = ct{954};
t2944 = ct{955};
t2945 = ct{956};
t2946 = ct{957};
t2948 = ct{958};
t2949 = ct{959};
t295 = ct{960};
t2950 = ct{961};
t2953 = ct{962};
t2954 = ct{963};
t2955 = ct{964};
t2956 = ct{965};
t2957 = ct{966};
t296 = ct{967};
t2960 = ct{968};
t2961 = ct{969};
t2962 = ct{970};
t297 = ct{971};
t2972 = ct{972};
t2974 = ct{973};
t298 = ct{974};
t2989 = ct{975};
t2991 = ct{976};
t2996 = ct{977};
t2997 = ct{978};
t2998 = ct{979};
t2999 = ct{980};
t3 = ct{981};
t30 = ct{982};
t3008 = ct{983};
t3009 = ct{984};
t301 = ct{985};
t3011 = ct{986};
t3020 = ct{987};
t3031 = ct{988};
t3035 = ct{989};
t3038 = ct{990};
t3039 = ct{991};
t3040 = ct{992};
t3041 = ct{993};
t3042 = ct{994};
t3045 = ct{995};
t3047 = ct{996};
t3048 = ct{997};
t3051 = ct{998};
t3052 = ct{999};
t3060 = ct{1000};
t3066 = ct{1001};
t3067 = ct{1002};
t307 = ct{1003};
t3071 = ct{1004};
t3075 = ct{1005};
t3076 = ct{1006};
t308 = ct{1007};
t3082 = ct{1008};
t3083 = ct{1009};
t3085 = ct{1010};
t3086 = ct{1011};
t3088 = ct{1012};
t309 = ct{1013};
t3092 = ct{1014};
t3097 = ct{1015};
t3098 = ct{1016};
t3099 = ct{1017};
t31 = ct{1018};
t310 = ct{1019};
t3104 = ct{1020};
t3106 = ct{1021};
t3107 = ct{1022};
t311 = ct{1023};
t3112 = ct{1024};
t3113 = ct{1025};
t312 = ct{1026};
t3120 = ct{1027};
t3121 = ct{1028};
t3122 = ct{1029};
t3124 = ct{1030};
t3126 = ct{1031};
t3128 = ct{1032};
t3129 = ct{1033};
t313 = ct{1034};
t3130 = ct{1035};
t3131 = ct{1036};
t3132 = ct{1037};
t3133 = ct{1038};
t3140 = ct{1039};
t3141 = ct{1040};
t3142 = ct{1041};
t3143 = ct{1042};
t3148 = ct{1043};
t3152 = ct{1044};
t3153 = ct{1045};
t3154 = ct{1046};
t3155 = ct{1047};
t3159 = ct{1048};
t3161 = ct{1049};
t3162 = ct{1050};
t3163 = ct{1051};
t3165 = ct{1052};
t3166 = ct{1053};
t3168 = ct{1054};
t317 = ct{1055};
t3170 = ct{1056};
t3171 = ct{1057};
t3172 = ct{1058};
t3175 = ct{1059};
t3179 = ct{1060};
t318 = ct{1061};
t3181 = ct{1062};
t3186 = ct{1063};
t319 = ct{1064};
t3190 = ct{1065};
t3192 = ct{1066};
t3193 = ct{1067};
t3194 = ct{1068};
t3195 = ct{1069};
t3196 = ct{1070};
t32 = ct{1071};
t320 = ct{1072};
t3201 = ct{1073};
t3202 = ct{1074};
t3203 = ct{1075};
t3204 = ct{1076};
t3205 = ct{1077};
t3206 = ct{1078};
t3210 = ct{1079};
t3215 = ct{1080};
t3226 = ct{1081};
t3229 = ct{1082};
t3232 = ct{1083};
t3235 = ct{1084};
t3238 = ct{1085};
t3246 = ct{1086};
t3248 = ct{1087};
t3249 = ct{1088};
t3252 = ct{1089};
t3253 = ct{1090};
t3255 = ct{1091};
t3257 = ct{1092};
t3260 = ct{1093};
t3261 = ct{1094};
t3262 = ct{1095};
t3263 = ct{1096};
t3264 = ct{1097};
t3268 = ct{1098};
t3269 = ct{1099};
t327 = ct{1100};
t3272 = ct{1101};
t3273 = ct{1102};
t3277 = ct{1103};
t3279 = ct{1104};
t328 = ct{1105};
t3280 = ct{1106};
t3284 = ct{1107};
t3285 = ct{1108};
t3286 = ct{1109};
t3287 = ct{1110};
t3288 = ct{1111};
t3289 = ct{1112};
t329 = ct{1113};
t3290 = ct{1114};
t3291 = ct{1115};
t3292 = ct{1116};
t3293 = ct{1117};
t3294 = ct{1118};
t3295 = ct{1119};
t3296 = ct{1120};
t33 = ct{1121};
t330 = ct{1122};
t3301 = ct{1123};
t331 = ct{1124};
t3311 = ct{1125};
t3312 = ct{1126};
t3313 = ct{1127};
t3315 = ct{1128};
t3316 = ct{1129};
t3321 = ct{1130};
t3324 = ct{1131};
t3336 = ct{1132};
t3340 = ct{1133};
t3342 = ct{1134};
t3356 = ct{1135};
t3357 = ct{1136};
t3358 = ct{1137};
t3359 = ct{1138};
t3360 = ct{1139};
t3361 = ct{1140};
t3362 = ct{1141};
t3363 = ct{1142};
t3364 = ct{1143};
t3365 = ct{1144};
t3366 = ct{1145};
t3369 = ct{1146};
t3372 = ct{1147};
t3375 = ct{1148};
t3377 = ct{1149};
t338 = ct{1150};
t3382 = ct{1151};
t3384 = ct{1152};
t3386 = ct{1153};
t3388 = ct{1154};
t3392 = ct{1155};
t3393 = ct{1156};
t3394 = ct{1157};
t3395 = ct{1158};
t3397 = ct{1159};
t3398 = ct{1160};
t3399 = ct{1161};
t34 = ct{1162};
t3400 = ct{1163};
t3402 = ct{1164};
t3403 = ct{1165};
t3406 = ct{1166};
t3407 = ct{1167};
t3411 = ct{1168};
t3413 = ct{1169};
t3414 = ct{1170};
t3417 = ct{1171};
t3418 = ct{1172};
t342 = ct{1173};
t3421 = ct{1174};
t3422 = ct{1175};
t3424 = ct{1176};
t3426 = ct{1177};
t3429 = ct{1178};
t3433 = ct{1179};
t3436 = ct{1180};
t3437 = ct{1181};
t3438 = ct{1182};
t3440 = ct{1183};
t3443 = ct{1184};
t3444 = ct{1185};
t3452 = ct{1186};
t346 = ct{1187};
t3460 = ct{1188};
t3464 = ct{1189};
t3465 = ct{1190};
t3468 = ct{1191};
t3470 = ct{1192};
t3476 = ct{1193};
t3479 = ct{1194};
t3480 = ct{1195};
t3481 = ct{1196};
t3482 = ct{1197};
t3483 = ct{1198};
t3486 = ct{1199};
t3488 = ct{1200};
t3489 = ct{1201};
t349 = ct{1202};
t3490 = ct{1203};
t3491 = ct{1204};
t3492 = ct{1205};
t3495 = ct{1206};
t3498 = ct{1207};
t35 = ct{1208};
t3502 = ct{1209};
t3504 = ct{1210};
t3506 = ct{1211};
t3514 = ct{1212};
t3526 = ct{1213};
t3527 = ct{1214};
t3528 = ct{1215};
t3535 = ct{1216};
t3536 = ct{1217};
t3537 = ct{1218};
t3538 = ct{1219};
t3540 = ct{1220};
t3542 = ct{1221};
t3544 = ct{1222};
t3546 = ct{1223};
t3547 = ct{1224};
t3551 = ct{1225};
t3555 = ct{1226};
t3556 = ct{1227};
t3559 = ct{1228};
t3561 = ct{1229};
t36 = ct{1230};
t3610 = ct{1231};
t3617 = ct{1232};
t3618 = ct{1233};
t3619 = ct{1234};
t3620 = ct{1235};
t3625 = ct{1236};
t3626 = ct{1237};
t3627 = ct{1238};
t3628 = ct{1239};
t3640 = ct{1240};
t3641 = ct{1241};
t3642 = ct{1242};
t3643 = ct{1243};
t3644 = ct{1244};
t3645 = ct{1245};
t3646 = ct{1246};
t3648 = ct{1247};
t3649 = ct{1248};
t3651 = ct{1249};
t3652 = ct{1250};
t3653 = ct{1251};
t3654 = ct{1252};
t3655 = ct{1253};
t3658 = ct{1254};
t3660 = ct{1255};
t3661 = ct{1256};
t3662 = ct{1257};
t3663 = ct{1258};
t3664 = ct{1259};
t3665 = ct{1260};
t3666 = ct{1261};
t3667 = ct{1262};
t3668 = ct{1263};
t3669 = ct{1264};
t3670 = ct{1265};
t3671 = ct{1266};
t3672 = ct{1267};
t3673 = ct{1268};
t3674 = ct{1269};
t3679 = ct{1270};
t3685 = ct{1271};
t37 = ct{1272};
t3720 = ct{1273};
t3751 = ct{1274};
t3776 = ct{1275};
t3779 = ct{1276};
t3780 = ct{1277};
t3781 = ct{1278};
t3782 = ct{1279};
t3783 = ct{1280};
t3784 = ct{1281};
t3786 = ct{1282};
t3788 = ct{1283};
t3789 = ct{1284};
t3790 = ct{1285};
t3796 = ct{1286};
t3798 = ct{1287};
t3811 = ct{1288};
t3812 = ct{1289};
t3816 = ct{1290};
t3818 = ct{1291};
t3820 = ct{1292};
t3821 = ct{1293};
t3823 = ct{1294};
t3824 = ct{1295};
t3825 = ct{1296};
t3826 = ct{1297};
t3828 = ct{1298};
t3829 = ct{1299};
t3833 = ct{1300};
t3835 = ct{1301};
t3838 = ct{1302};
t3839 = ct{1303};
t3840 = ct{1304};
t3841 = ct{1305};
t3842 = ct{1306};
t3843 = ct{1307};
t3844 = ct{1308};
t3845 = ct{1309};
t39 = ct{1310};
t4 = ct{1311};
t40 = ct{1312};
t427 = ct{1313};
t428 = ct{1314};
t429 = ct{1315};
t43 = ct{1316};
t431 = ct{1317};
t433 = ct{1318};
t435 = ct{1319};
t436 = ct{1320};
t439 = ct{1321};
t441 = ct{1322};
t444 = ct{1323};
t448 = ct{1324};
t45 = ct{1325};
t450 = ct{1326};
t451 = ct{1327};
t452 = ct{1328};
t453 = ct{1329};
t455 = ct{1330};
t456 = ct{1331};
t457 = ct{1332};
t458 = ct{1333};
t459 = ct{1334};
t46 = ct{1335};
t460 = ct{1336};
t461 = ct{1337};
t463 = ct{1338};
t465 = ct{1339};
t466 = ct{1340};
t469 = ct{1341};
t49 = ct{1342};
t494 = ct{1343};
t5 = ct{1344};
t50 = ct{1345};
t51 = ct{1346};
t510 = ct{1347};
t512 = ct{1348};
t515 = ct{1349};
t516 = ct{1350};
t517 = ct{1351};
t518 = ct{1352};
t522 = ct{1353};
t523 = ct{1354};
t524 = ct{1355};
t525 = ct{1356};
t526 = ct{1357};
t527 = ct{1358};
t528 = ct{1359};
t529 = ct{1360};
t530 = ct{1361};
t535 = ct{1362};
t536 = ct{1363};
t537 = ct{1364};
t538 = ct{1365};
t542 = ct{1366};
t547 = ct{1367};
t548 = ct{1368};
t55 = ct{1369};
t553 = ct{1370};
t554 = ct{1371};
t556 = ct{1372};
t561 = ct{1373};
t562 = ct{1374};
t563 = ct{1375};
t564 = ct{1376};
t565 = ct{1377};
t566 = ct{1378};
t567 = ct{1379};
t568 = ct{1380};
t569 = ct{1381};
t57 = ct{1382};
t570 = ct{1383};
t571 = ct{1384};
t572 = ct{1385};
t573 = ct{1386};
t574 = ct{1387};
t58 = ct{1388};
t580 = ct{1389};
t581 = ct{1390};
t583 = ct{1391};
t594 = ct{1392};
t595 = ct{1393};
t596 = ct{1394};
t6 = ct{1395};
t600 = ct{1396};
t601 = ct{1397};
t602 = ct{1398};
t603 = ct{1399};
t604 = ct{1400};
t605 = ct{1401};
t606 = ct{1402};
t607 = ct{1403};
t608 = ct{1404};
t609 = ct{1405};
t61 = ct{1406};
t612 = ct{1407};
t613 = ct{1408};
t614 = ct{1409};
t615 = ct{1410};
t616 = ct{1411};
t617 = ct{1412};
t618 = ct{1413};
t619 = ct{1414};
t620 = ct{1415};
t621 = ct{1416};
t622 = ct{1417};
t624 = ct{1418};
t626 = ct{1419};
t629 = ct{1420};
t63 = ct{1421};
t631 = ct{1422};
t632 = ct{1423};
t633 = ct{1424};
t634 = ct{1425};
t635 = ct{1426};
t637 = ct{1427};
t639 = ct{1428};
t64 = ct{1429};
t640 = ct{1430};
t642 = ct{1431};
t643 = ct{1432};
t644 = ct{1433};
t646 = ct{1434};
t647 = ct{1435};
t648 = ct{1436};
t649 = ct{1437};
t650 = ct{1438};
t651 = ct{1439};
t652 = ct{1440};
t653 = ct{1441};
t654 = ct{1442};
t656 = ct{1443};
t657 = ct{1444};
t658 = ct{1445};
t660 = ct{1446};
t661 = ct{1447};
t662 = ct{1448};
t663 = ct{1449};
t664 = ct{1450};
t665 = ct{1451};
t667 = ct{1452};
t67 = ct{1453};
t673 = ct{1454};
t676 = ct{1455};
t677 = ct{1456};
t678 = ct{1457};
t685 = ct{1458};
t687 = ct{1459};
t688 = ct{1460};
t689 = ct{1461};
t69 = ct{1462};
t691 = ct{1463};
t692 = ct{1464};
t693 = ct{1465};
t694 = ct{1466};
t696 = ct{1467};
t697 = ct{1468};
t698 = ct{1469};
t7 = ct{1470};
t70 = ct{1471};
t701 = ct{1472};
t702 = ct{1473};
t703 = ct{1474};
t704 = ct{1475};
t705 = ct{1476};
t707 = ct{1477};
t708 = ct{1478};
t71 = ct{1479};
t72 = ct{1480};
t721 = ct{1481};
t722 = ct{1482};
t723 = ct{1483};
t724 = ct{1484};
t725 = ct{1485};
t726 = ct{1486};
t728 = ct{1487};
t729 = ct{1488};
t73 = ct{1489};
t730 = ct{1490};
t731 = ct{1491};
t735 = ct{1492};
t74 = ct{1493};
t743 = ct{1494};
t75 = ct{1495};
t754 = ct{1496};
t755 = ct{1497};
t756 = ct{1498};
t757 = ct{1499};
t76 = ct{1500};
t760 = ct{1501};
t762 = ct{1502};
t769 = ct{1503};
t77 = ct{1504};
t770 = ct{1505};
t773 = ct{1506};
t774 = ct{1507};
t776 = ct{1508};
t777 = ct{1509};
t778 = ct{1510};
t78 = ct{1511};
t785 = ct{1512};
t786 = ct{1513};
t787 = ct{1514};
t788 = ct{1515};
t79 = ct{1516};
t791 = ct{1517};
t792 = ct{1518};
t795 = ct{1519};
t796 = ct{1520};
t797 = ct{1521};
t8 = ct{1522};
t80 = ct{1523};
t800 = ct{1524};
t805 = ct{1525};
t806 = ct{1526};
t81 = ct{1527};
t813 = ct{1528};
t815 = ct{1529};
t817 = ct{1530};
t818 = ct{1531};
t819 = ct{1532};
t82 = ct{1533};
t827 = ct{1534};
t83 = ct{1535};
t831 = ct{1536};
t834 = ct{1537};
t835 = ct{1538};
t836 = ct{1539};
t837 = ct{1540};
t838 = ct{1541};
t839 = ct{1542};
t84 = ct{1543};
t840 = ct{1544};
t841 = ct{1545};
t842 = ct{1546};
t843 = ct{1547};
t845 = ct{1548};
t846 = ct{1549};
t847 = ct{1550};
t85 = ct{1551};
t853 = ct{1552};
t854 = ct{1553};
t855 = ct{1554};
t856 = ct{1555};
t857 = ct{1556};
t859 = ct{1557};
t86 = ct{1558};
t860 = ct{1559};
t863 = ct{1560};
t864 = ct{1561};
t866 = ct{1562};
t867 = ct{1563};
t87 = ct{1564};
t870 = ct{1565};
t871 = ct{1566};
t873 = ct{1567};
t876 = ct{1568};
t877 = ct{1569};
t878 = ct{1570};
t88 = ct{1571};
t880 = ct{1572};
t881 = ct{1573};
t882 = ct{1574};
t884 = ct{1575};
t885 = ct{1576};
t888 = ct{1577};
t889 = ct{1578};
t89 = ct{1579};
t890 = ct{1580};
t891 = ct{1581};
t896 = ct{1582};
t898 = ct{1583};
t899 = ct{1584};
t9 = ct{1585};
t90 = ct{1586};
t900 = ct{1587};
t902 = ct{1588};
t905 = ct{1589};
t907 = ct{1590};
t908 = ct{1591};
t91 = ct{1592};
t911 = ct{1593};
t92 = ct{1594};
t921 = ct{1595};
t926 = ct{1596};
t927 = ct{1597};
t928 = ct{1598};
t930 = ct{1599};
t932 = ct{1600};
t933 = ct{1601};
t935 = ct{1602};
t939 = ct{1603};
t94 = ct{1604};
t940 = ct{1605};
t942 = ct{1606};
t948 = ct{1607};
t949 = ct{1608};
t952 = ct{1609};
t958 = ct{1610};
t959 = ct{1611};
t966 = ct{1612};
t969 = ct{1613};
t97 = ct{1614};
t972 = ct{1615};
t973 = ct{1616};
t974 = ct{1617};
t975 = ct{1618};
t982 = ct{1619};
t983 = ct{1620};
t984 = ct{1621};
t987 = ct{1622};
t988 = ct{1623};
t992 = ct{1624};
t994 = ct{1625};
et157 = t271+t428+t614.*2.75e-2+t757-t860.*2.019e-2-t863.*4.9e-4-t1515.*4.9e-4;
et158 = t1526.*2.019e-2+t13.*(t86-t652).*2.75e-2;
et159 = dq2.*t3.*t23.*8.909980864224564e-21+dq2.*t3.*t26.*8.909980864224564e-21-dq2.*t10.*t23.*1.16152294893368e-19;
et160 = dq2.*t10.*t26.*(-1.16152294893368e-19);
et161 = t2627.*(t1386+t7.*(t88-t617)).*2.2e-4+t2654.*(t1386+t7.*(t88-t617)).*1.089e-2;
et162 = t2074.*t2576.*2.2e-4+t2074.*t2601.*1.089e-2;
et163 = t2601.*t2627.*2.9e-4-t2576.*t2654.*2.9e-4;
et164 = t2000.*(t614+t13.*(t86-t652)).*2.81e-3+t2035.*(t1386+t7.*(t88-t617)).*4.000000000000028e-5;
et165 = t2000.*t2074.*4.000000000000028e-5-t2035.*(t653-t838).*2.81e-3;
et166 = t2074.*(t653-t838).*(-5.0e-5)-(t614+t13.*(t86-t652)).*(t1386+t7.*(t88-t617)).*5.0e-5;
et167 = t3.*t23.*1.0e-4+t3.*t26.*1.0e-4;
et168 = t10.*t23.*5.582083966615414e-19+t10.*t26.*5.582083966615414e-19;
et169 = t2163.*(t614+t13.*(t86-t652)).*(-9.999999999999998e-6)+t2828.*(t614+t13.*(t86-t652)).*1.2e-4;
et170 = t1206.*t2147.*4.466636216449161e-20+t1295.*t2163.*4.466636216449161e-20+t831.*t2816.*9.999999999999998e-6;
et171 = t831.*t2828.*4.466636216449161e-20-t1206.*t2832.*1.2e-4;
et172 = t1295.*t2816.*1.2e-4+(t88-t617).*(t639-t1128-t2181+dq5.*t13.*(t86-t652)).*4.466636216449161e-20;
et173 = (t653-t838).*(t639-t1128-t2181+dq5.*t13.*(t86-t652)).*(-1.2e-4)+t2832.*(t88-t617).*9.999999999999998e-6;
et174 = t2147.*(t653-t838).*(-9.999999999999998e-6);
et175 = t2576.*(t884+t1578-t2180+t14.*(t639-t1128-t2181+dq5.*t13.*(t86-t652))).*7.950000000000001e-3;
et176 = t2601.*(t884+t1578-t2180+t14.*(t639-t1128-t2181+dq5.*t13.*(t86-t652))).*2.2e-4+t3619.*(t1386+t7.*(t88-t617)).*2.2e-4;
et177 = t3620.*(t1386+t7.*(t88-t617)).*(-7.950000000000001e-3)-t2074.*t3617.*7.950000000000001e-3;
et178 = t2074.*t3618.*2.2e-4-t2627.*t3312.*7.950000000000001e-3;
et179 = t2654.*t3312.*(-2.2e-4)-t2576.*t3619.*2.900000000000001e-4;
et180 = t2601.*t3620.*(-2.900000000000001e-4)+t2627.*t3618.*2.900000000000001e-4;
et181 = t2654.*t3617.*2.900000000000001e-4;
et182 = t1206.*(t614+t13.*(t86-t652)).*4.466636216449161e-20+t831.*t1206.*2.840000000000012e-3;
et183 = (t614+t13.*(t86-t652)).*(t88-t617).*1.0e-5+t1295.*(t88-t617).*2.840000000000012e-3;
et184 = t831.*(t653-t838).*1.0e-5-t1295.*(t653-t838).*4.466636216449161e-20;
et185 = t831.*t1040.*3.844e-2-t815.*t1066.*8.8e-4;
et186 = t572.*t2163.*(-3.844e-2)+t572.*t2164.*8.8e-4;
et187 = t604.*t2147.*(-3.844e-2)+t604.*t2148.*8.8e-4;
et188 = t815.*t2147.*1.12e-3+t831.*t2164.*1.12e-3;
et189 = t1066.*(t88-t617).*3.844e-2-t1040.*(t86-t652).*8.8e-4;
et190 = t2148.*(t88-t617).*(-1.12e-3)-t2163.*(t86-t652).*1.12e-3;
et191 = -t2711+t2801-t2954+t2956-t3179+t3181+t2165.*(t92-t663).*4.466636216449161e-20+t2816.*(t88-t617).*1.0e-5;
et192 = t2828.*(t653-t838).*4.466636216449161e-20;
et193 = t39.*t571.*4.999999999999997e-5+t45.*t572.*2.23e-3;
et194 = t50.*t572.*2.23e-3-t61.*t571.*4.999999999999997e-5;
et195 = t39.*t604.*2.23e-3+t45.*t605.*4.999999999999997e-5;
et196 = t50.*t605.*4.999999999999997e-5-t61.*t604.*2.23e-3;
et197 = t604.*t1020.*7.000000000000001e-5+t571.*t1066.*7.000000000000001e-5;
et198 = t572.*t1067.*7.000000000000001e-5-t605.*t1040.*7.000000000000001e-5;
et199 = t9.*t10.*t1020.*4.999999999999997e-5-t2.*t10.*t1040.*2.23e-3;
et200 = t2.*t10.*t1067.*(-4.999999999999997e-5)-t9.*t10.*t1066.*2.23e-3;
et201 = t572.*t815.*1.144e-2-t604.*t831.*8.8e-4;
et202 = t815.*t831.*1.11e-3-t572.*(t88-t617).*8.8e-4;
et203 = t604.*(t86-t652).*1.144e-2-(t88-t617).*(t86-t652).*1.11e-3;
et204 = t2828.*(t614+t13.*(t86-t652))-t1206.*t2832+t1295.*t2816-(t653-t838).*(t639-t1128-t2181+dq5.*t13.*(t86-t652));
et205 = (-t2447-t2783-t2839+t2841+t3126+t3143+t3232+t2165.*(t92-t663).*1.2e-4+t2828.*(t653-t838).*1.2e-4)./2.0;
et206 = t2627.*(t1386+t7.*(t88-t617)).*2.900000000000001e-4+t2654.*(t1386+t7.*(t88-t617)).*2.9e-4;
et207 = t2074.*t2576.*2.900000000000001e-4+t2074.*t2601.*2.9e-4;
et208 = t2601.*t2627.*2.94e-3-t2576.*t2654.*2.94e-3;
et209 = t815.*t1066-t572.*t2164-t604.*t2148+t1040.*(t86-t652);
et210 = (t2388+t2445.*1.11e-3-t2467+t2496-t2693-t2798+t2810+t2829+t1066.*(t86-t652).*1.144e-2)./2.0;
et211 = t831.*t1040.*1.12e-3-t815.*t1066.*1.11e-3;
et212 = t572.*t2163.*(-1.12e-3)+t572.*t2164.*1.11e-3;
et213 = t604.*t2147.*(-1.12e-3)+t604.*t2148.*1.11e-3;
et214 = t815.*t2147.*4.988e-2+t831.*t2164.*4.988e-2;
et215 = t1066.*(t88-t617).*1.12e-3-t1040.*(t86-t652).*1.11e-3;
et216 = t2148.*(t88-t617).*(-4.988e-2)-t2163.*(t86-t652).*4.988e-2;
et217 = t3838.*(et1+et2+et3).*(-1.0./2.0)+(t1025.*(et4+et5))./2.0-t3248.*(t9.*(-3.55e-3)+t2.*t3.*7.669999999999999e-3+t2.*t10.*1.6669e-1).*4.50275;
et218 = t3249.*(t2.*3.55e-3+t3.*t9.*7.669999999999999e-3+t9.*t10.*1.6669e-1).*4.50275+t3786.*(et6+et7).*(3.41e+2./1.0e+2)+et8.*et9+(t3826.*(t815.*t831-(t88-t617).*(t86-t652)))./2.0-(t2756.*(et10+et11))./2.0;
et219 = (-t3312.*(t614+t13.*(t86-t652))+t2832.*(t1386+t7.*(t88-t617))+t2074.*t2816+(t653-t838).*(t884+t1578-t2180+t14.*(t639-t1128-t2181+dq5.*t13.*(t86-t652)))).*(et12+et13).*(-1.0./2.0)+et14.*et15+((t2056-t2360-t2788-t2807+t3051+t2962.*(t88-t617)).*(et16+et17+et18))./2.0-((et19+et20+et21).*(t2817+t3324+t3433.*(t614+t13.*(t86-t652))+t2832.*(t639-t1128-t2181+dq5.*t13.*(t86-t652))+t2974.*(t92-t663)+t3422.*(t653-t838)))./2.0+t3781.*(et22+et23).*2.61155;
et220 = t3780.*(et24+et25).*(-2.61155)-(t3668.*(t604.*t1020+t571.*t1066+t572.*t1067-t605.*t1040))./2.0+((t2576.*t3619+t2601.*t3620-t2627.*t3618-t2654.*t3617).*(et26+et27))./2.0-(t3818.*(t2000.*(t884+t1578-t2180+t14.*(t639-t1128-t2181+dq5.*t13.*(t86-t652)))-t2035.*t3312+t2074.*(t1487+t2219-t2864+dq6.*t7.*(t88-t617))-(t1386+t7.*(t88-t617)).*(t878-t1582+t2184+t7.*(t639-t1128-t2181+dq5.*t13.*(t86-t652)))))./2.0-(t3372.*(et28+et29+et30))./2.0+(t624.*(et31+et32))./2.0-t3784.*(et33+et34).*(3.41e+2./1.0e+2);
et221 = (t3377+t2074.*(t878-t1582+t2184+t7.*(t639-t1128-t2181+dq5.*t13.*(t86-t652)))+t1207.*(t642+t896-t1137-t2220)).*(et35+et36+et37+et38+et39+et40+et41).*(-1.0./2.0)-(t3828.*(et42+et43+et44))./2.0-(t3783.*(et45+et46+et47))./2.0+(t3666.*(et48+et49+et50))./2.0-((t2601.*(t884+t1578-t2180+t14.*(t639-t1128-t2181+dq5.*t13.*(t86-t652)))+t3619.*(t1386+t7.*(t88-t617))+t2074.*t3618-t2654.*t3312).*(et51+et52))./2.0+(((t614+t13.*(t86-t652)).*(t88-t617)+t831.*(t653-t838)).*(et53+et54+et55))./2.0;
et222 = (t831.*t1206+t1295.*(t88-t617)).*(et56+et57+et58).*(-1.0./2.0)-((t859-t1791+t1066.*(t86-t652)).*(et59+et60+et61+et62+et63+et64))./2.0+(t3364.*(et65+et66+et67))./2.0-((-t2961+t3358+t3312.*(t653-t838)).*(et68+et69+et70+et71+et72+et73+et74))./2.0-(t2296.*(et75+et76))./2.0+(t3440.*(dq2.*t3.*t23+dq2.*t3.*t26))./2.0-(t3443.*(dq2.*t10.*t23+dq2.*t10.*t26))./2.0-((t10.*t23+t10.*t26).*(et77+et78+et79+et80+et81))./2.0-(t3788.*(t2163.*(t614+t13.*(t86-t652))-t831.*t2816-t2832.*(t88-t617)+t2147.*(t653-t838)))./2.0;
et223 = ((-t2576.*(t884+t1578-t2180+t14.*(t639-t1128-t2181+dq5.*t13.*(t86-t652)))+t3620.*(t1386+t7.*(t88-t617))+t2074.*t3617+t2627.*t3312).*(et82+et83))./2.0+t3835.*(et84+et85).*3.5432e-1-t3833.*(et86+et87).*3.5432e-1-(t2533.*(et88+et89+et90+et91+et92+et93+et94+et95))./2.0-(t3610.*(et96+et97+et98+et99+et100+et101+et102))./2.0-((et103+et104+et105).*(t3140+t3489+t3720+t2832.*(t884+t1578-t2180+t14.*(t639-t1128-t2181+dq5.*t13.*(t86-t652)))+t3436.*(t92-t663)+t3685.*(t653-t838)))./2.0-(t3272.*(et106+et107+et108+et109+et110+et111))./2.0;
et224 = (t3789.*(et112+et113+et114+et115+et116+et117+et118))./2.0-(t3840.*(t2035.*(t1386+t7.*(t88-t617))+t2000.*t2074))./2.0-(t3845.*(t2627.*(t1386+t7.*(t88-t617))+t2074.*t2576))./2.0-(t3843.*(t2654.*(t1386+t7.*(t88-t617))+t2074.*t2601))./2.0-t3823.*(et119+et120).*3.38795+(t1866.*(et121+et122+et123+et124+et125+et126+et127+et128))./2.0+((t2370-t2949+t2816.*(t88-t617)).*(et129+et130+et131+et132+et133+et134))./2.0-(t2943.*(et135+et136+et137))./2.0-((t1206.*(t614+t13.*(t86-t652))-t1295.*(t653-t838)).*(et138+et139+et140))./2.0;
et225 = (-t3113+t3418+t2654.*(t884+t1578-t2180+t14.*(t639-t1128-t2181+dq5.*t13.*(t86-t652)))).*(et141+et142+et143+et144+et145+et146+et147).*(-1.0./2.0)+t3673.*(et148+et149).*2.4552-t3672.*(et150+et151).*2.4552-(t3841.*(t2074.*(t653-t838)+(t614+t13.*(t86-t652)).*(t1386+t7.*(t88-t617))))./2.0+(t3812.*(t9.*t10.*t572+t2.*t10.*t604))./2.0-(t3816.*(t2.*t10.*t571+t9.*t10.*t605))./2.0-((t3.*t23+t3.*t26).*(et152+et153+et154+et155+et156))./2.0;
et226 = t3820.*(t2000.*t2832-t2035.*t2816+(t653-t838).*(t878-t1582+t2184+t7.*(t639-t1128-t2181+dq5.*t13.*(t86-t652)))+(t614+t13.*(t86-t652)).*(t1487+t2219-t2864+dq6.*t7.*(t88-t617))).*(-1.0./2.0)-(t3811.*(t571.*t572-t604.*t605))./2.0-(t3844.*(t2601.*t2627-t2576.*t2654))./2.0-(et157+et158).*(t221.*(2.1e+1./5.0e+1)+t223.*(2.1e+1./5.0e+1)-t542+t547+t548-t554+t580+t581+t583+t800+t1424+t1726+t1856+t1898+t1934+t2042+t2198+t2231+t2253+t2558+t2581+t2587+t2602+t2991+t2997+t3066+t3075+t3082+t3495+t3498).*3.38795;
et227 = t3669.*(t39.*t571+t45.*t605+t50.*t605+t185.*t571+t9.*t10.*t1020-t2.*t10.*t1067).*(-1.0./2.0)+(t3667.*(t45.*t572+t50.*t572+t39.*t604+t185.*t604-t2.*t10.*t1040-t9.*t10.*t1066))./2.0+(t1256.*(et159+et160))./2.0-(t3829.*(et161+et162+et163))./2.0-((t3502+t3544-t3547+t2972.*(t621-t864)+t2196.*(t642+t896-t1137-t2220)+t2816.*(t1487+t2219-t2864+dq6.*t7.*(t88-t617))).*(et164+et165+et166))./2.0-(t3842.*(t2000.*(t614+t13.*(t86-t652))-t2035.*(t653-t838)))./2.0-(t702.*(et167+et168))./2.0+((t3031+t2165.*(t92-t663)+t2828.*(t653-t838)).*(et169+et170+et171+et172+et173+et174))./2.0;
et228 = t3782.*(et175+et176+et177+et178+et179+et180+et181).*(-1.0./2.0)-((t2407+t2563+t3085-t3092-t3122+t2147.*(t639-t1128-t2181+dq5.*t13.*(t86-t652))).*(et182+et183+et184))./2.0+(t3060.*(et185+et186+et187+et188+et189+et190))./2.0+((t1206.*t2147+t1295.*t2163+t831.*t2828+(t88-t617).*(t639-t1128-t2181+dq5.*t13.*(t86-t652))).*(et191+et192))./2.0-(t2384.*(et193+et194+et195+et196+et197+et198+et199+et200))./2.0-(t3546.*(et201+et202+et203))./2.0+et204.*et205-(t3839.*(et206+et207+et208))./2.0-(t3824.*(t604.*t831+t572.*(t88-t617)))./2.0+(t3825.*(t572.*t815+t604.*(t86-t652)))./2.0+et209.*et210-(t3192.*(et211+et212+et213+et214+et215+et216))./2.0;
et229 = t16.*cos(t1026).*sin(t1026).*5.8743807581e-5+t16.*cos(t1058).*sin(t1058).*5.8743807581e-5;
et230 = -t3196-t3253-t3262+t3406+t3452+t2074.*(t878-t1582+t2184+t7.*(t639-t1128-t2181+dq5.*t13.*(t86-t652))).*3.0e-5+t2196.*(t621-t864).*5.0e-5;
et231 = t3312.*(t653-t838).*5.000000000000004e-4+t1207.*(t642+t896-t1137-t2220).*3.0e-5;
et232 = t450+t453+t469+t510+t530+t596+t854.*2.75e-2-t973+t1455+t1740+t1775+t1782+t1909.*2.019e-2+t1913.*4.9e-4-t1918.*2.75e-2+t1974+t1986;
et233 = t2640.*(-4.9e-4)+t2642.*2.019e-2;
et234 = -t3291+t3365.*2.900000000000001e-4+t3527+t3642+t3654-t3662-t3665+t2654.*(t884+t1578-t2180+t14.*(t639-t1128-t2181+dq5.*t13.*(t86-t652))).*2.9e-4;
et235 = t3336.*(t8.*(t92-t663)+t15.*(t621-t864)).*2.94e-3;
et236 = t3205+t2000.*(t284+t287+t290-t329-t805-t1951).*2.81e-3+t1681.*(t884+t1578-t2180+t14.*(t639-t1128-t2181+dq5.*t13.*(t86-t652))).*4.000000000000028e-5;
et237 = t3124.*(t614+t13.*(t86-t652)).*5.0e-5-t3121.*(t1386+t7.*(t88-t617)).*4.000000000000028e-5;
et238 = t1296.*t2196.*5.0e-5-t1654.*t2816.*5.0e-5;
et239 = t1649.*t2832.*5.0e-5+t2035.*t2671.*2.81e-3;
et240 = t1685.*t3312.*(-4.000000000000028e-5)-(t243-t786).*(t878-t1582+t2184+t7.*(t639-t1128-t2181+dq5.*t13.*(t86-t652))).*2.81e-3;
et241 = t2854.*(t92-t663).*5.0e-5+t2177.*(t621-t864).*2.81e-3;
et242 = t3120.*(t653-t838).*5.0e-5-(t665+t7.*(t90-t615)).*(t631-t885+t1132-t2224).*4.000000000000028e-5;
et243 = t817.*(t642+t896-t1137-t2220).*(-2.81e-3)-t2074.*(t755+t1012-t1905-t2692).*4.000000000000028e-5;
et244 = (t252-t791).*(t1487+t2219-t2864+dq6.*t7.*(t88-t617)).*(-2.81e-3);
et245 = -t3294+t3365.*7.950000000000001e-3+t3528+t3648+t3658-t3660-t3663+t2654.*(t884+t1578-t2180+t14.*(t639-t1128-t2181+dq5.*t13.*(t86-t652))).*2.2e-4;
et246 = t3336.*(t8.*(t92-t663)+t15.*(t621-t864)).*2.900000000000001e-4;
et247 = t1217+t51.*t607+t58.*t607+t633.*t1040-t632.*t1066-t572.*t1852-t604.*t1896;
et248 = (t2365+t2445.*1.12e-3-t2456+t2536-t2653-t2789+t2803+t2868+t1066.*(t86-t652).*8.8e-4).*(-1.0./2.0);
et249 = t573.*t574.*(-1.12e-3)-t572.*t632.*3.844e-2;
et250 = t604.*t633.*3.844e-2+t676.*t831.*1.12e-3;
et251 = t677.*(t88-t617).*1.12e-3+t3.*t11.*t606.*8.8e-4;
et252 = t10.*t11.*t607.*(-3.844e-2)+t10.*t35.*t815.*8.8e-4;
et253 = t10.*t31.*(t86-t652).*8.8e-4;
et254 = t4.*t27.*(-4.999999999999997e-5)+t11.*t24.*2.23e-3;
et255 = t11.*t23.*t27.*2.23e-3+t11.*t26.*t27.*2.23e-3;
et256 = t3.*t9.*t571.*(-4.999999999999997e-5)+t2.*t3.*t605.*4.999999999999997e-5;
et257 = t10.*t29.*t572.*7.000000000000001e-5-t10.*t32.*t604.*7.000000000000001e-5;
et258 = t3.*t4.*t10.*t11.*(-7.000000000000001e-5);
et259 = -t2630.*(t614+t13.*(t86-t652))+t817.*t2165-(t243-t786).*(t639-t1128-t2181+dq5.*t13.*(t86-t652))+t2149.*(t92-t663)+t2828.*(t252-t791)+t2609.*(t653-t838);
et260 = (-t2447-t2783-t2839+t2841+t3126+t3143+t3232+t2165.*(t92-t663).*1.2e-4+t2828.*(t653-t838).*1.2e-4).*(-1.0./2.0);
et261 = t2471+t2622-t569.*t574.*1.11e-3+t603.*t606.*1.11e-3;
et262 = t815.*t818.*1.11e-3-t607.*t1069.*4.988e-2;
et263 = t677.*t1040.*(-1.11e-3)+t676.*t1066.*1.11e-3;
et264 = t572.*t1823.*1.12e-3+t604.*t1860.*1.12e-3;
et265 = t831.*t1855.*4.988e-2+t632.*t2148.*4.988e-2;
et266 = t633.*t2164.*4.988e-2+t842.*(t86-t652).*1.11e-3;
et267 = t1864.*(t88-t617).*4.988e-2-t3.*t11.*t1070.*1.12e-3;
et268 = t10.*t31.*t2147.*1.12e-3+t10.*t35.*t2163.*1.12e-3;
et269 = t34.*1.8866e-1-t81.*1.8866e-1+t83.*2.37e-3-t90.*5.000000000000001e-5+t105;
et270 = t615.*5.000000000000001e-5+t620.*2.37e-3;
et271 = t74.*1.8866e-1+t241.*1.8866e-1-t243.*2.37e-3+t251.*5.000000000000001e-5+t267;
et272 = t785.*5.000000000000001e-5+t786.*2.37e-3;
et273 = t80.*1.8866e-1+t250.*1.8866e-1-t252.*2.37e-3+t258.*5.000000000000001e-5+t272;
et274 = t787.*5.000000000000001e-5+t791.*2.37e-3;
et275 = t2471+t2622+t43.*t606.*1.11e-3-t51.*t607.*1.12e-3;
et276 = t58.*t607.*(-1.12e-3)-t64.*t606.*1.11e-3;
et277 = t137.*t815.*1.11e-3+t144.*t815.*1.11e-3;
et278 = t151.*t815.*1.11e-3+t574.*t1070.*4.988e-2;
et279 = t633.*t1040.*(-1.12e-3)+t632.*t1066.*1.12e-3;
et280 = t572.*t1852.*1.12e-3+t604.*t1896.*1.12e-3;
et281 = t831.*t1885.*4.988e-2+t676.*t2147.*4.988e-2;
et282 = t677.*t2163.*4.988e-2+t112.*(t86-t652).*1.11e-3;
et283 = t119.*(t86-t652).*1.11e-3-t171.*(t86-t652).*1.11e-3;
et284 = t1892.*(t88-t617).*4.988e-2+t3.*t11.*t1069.*1.11e-3;
et285 = t10.*t31.*t2148.*1.11e-3+t10.*t35.*t2164.*1.11e-3;
et286 = -t2844-t2914-t2922+t3052+t3229-t3264+t3269+t3280-t3284+t3295+t3301+t3369+t3556-t3559+t3433.*(t614+t13.*(t86-t652)).*9.999999999999998e-6;
et287 = t2832.*(t639-t1128-t2181+dq5.*t13.*(t86-t652)).*9.999999999999998e-6+t2974.*(t92-t663).*9.999999999999998e-6;
et288 = t3422.*(t653-t838).*9.999999999999998e-6;
et289 = t243.*(-2.75e-2)+t267+t427+t553-t722.*2.019e-2-t723.*4.9e-4+t786.*2.75e-2;
et290 = t1003.*4.9e-4-t1004.*2.019e-2;
et291 = t252.*(-2.75e-2)+t272+t429+t556-t724.*2.019e-2-t728.*4.9e-4+t791.*2.75e-2;
et292 = t1007.*4.9e-4-t1008.*2.019e-2;
et293 = t2060-t10.*t51.*9.999999999999995e-5-t11.*t208.*7.000000000000022e-5;
et294 = t37.*t571.*(-2.19e-3)+t63.*t571.*2.19e-3;
et295 = t46.*t605.*(-2.19e-3)-t49.*t605.*2.19e-3;
et296 = t97.*t572.*(-7.000000000000022e-5)+t107.*t604.*7.000000000000022e-5;
et297 = t139.*t572.*7.000000000000022e-5+t114.*t604.*7.000000000000022e-5;
et298 = t149.*t572.*7.000000000000022e-5-t175.*t604.*7.000000000000022e-5;
et299 = dq3.*t4.*t24.*4.999999999999997e-5+dq3.*t11.*t27.*2.19e-3;
et300 = t4.*t11.*t69.*7.000000000000022e-5+t10.*t23.*t51.*9.999999999999995e-5;
et301 = t10.*t26.*t51.*9.999999999999995e-5+t2.*t3.*t1020.*2.19e-3;
et302 = t3.*t9.*t1067.*2.19e-3-t10.*t32.*t1040.*7.000000000000022e-5;
et303 = t10.*t29.*t1066.*7.000000000000022e-5+dq3.*t3.*t10.*t25.*7.000000000000022e-5;
et304 = dq3.*t3.*t10.*t28.*(-7.000000000000022e-5)+dq3.*t4.*t23.*t27.*4.999999999999997e-5;
et305 = dq3.*t4.*t26.*t27.*4.999999999999997e-5;
et306 = t2060-t10.*t569.*4.999999999999997e-5+t3.*t603.*4.999999999999997e-5;
et307 = t571.*t600.*(-2.19e-3)-t568.*t605.*2.19e-3;
et308 = t572.*t840.*7.000000000000022e-5+t604.*t841.*7.000000000000022e-5;
et309 = t10.*t11.*t570.*(-7.000000000000022e-5)+t10.*t32.*t567.*2.19e-3;
et310 = t3.*t11.*t602.*7.000000000000022e-5+t10.*t29.*t601.*2.19e-3;
et311 = t9.*t10.*t818.*4.999999999999997e-5+t2.*t10.*t842.*4.999999999999997e-5;
et312 = t3.*t9.*t1040.*(-4.999999999999997e-5)+t10.*t31.*t1020.*7.000000000000022e-5;
et313 = t2.*t3.*t1066.*4.999999999999997e-5+t10.*t35.*t1067.*7.000000000000022e-5;
et314 = t2443+t2780+t2897+t2672.*(t614+t13.*(t86-t652)).*1.2e-4+t632.*(t639-t1128-t2181+dq5.*t13.*(t86-t652)).*4.466636216449161e-20;
et315 = (t88-t617).*(t284+t287+t290-t329-t805-t1951).*(-9.999999999999998e-6)+t817.*t1070.*9.999999999999998e-6;
et316 = t607.*t2165.*4.466636216449161e-20-t1206.*t1896.*4.466636216449161e-20-t1295.*t1852.*4.466636216449161e-20;
et317 = t633.*t2828.*(-4.466636216449161e-20)+t831.*t2671.*9.999999999999998e-6;
et318 = t940.*t2832.*(-1.2e-4)+t959.*t2816.*1.2e-4;
et319 = t2196.*(t90-t615).*1.2e-4-t2147.*(t243-t786).*9.999999999999998e-6;
et320 = t2163.*(t252-t791).*(-9.999999999999998e-6)-t2659.*(t653-t838).*1.2e-4;
et321 = t273.*2.0e-4+t275.*2.0e-4+t282.*5.267999999999999e-2+t285.*5.267999999999999e-2;
et322 = t312.*(-2.0e-4)-t328.*5.267999999999999e-2+t469+t530+t1299+t1347+t1350+t1351+t1389+t1391+t1431+t1441+t1543+t1546+t1605;
et323 = t270.*(-2.0e-4)-t274.*5.267999999999999e-2+t283.*2.0e-4+t288.*2.0e-4;
et324 = t307.*5.267999999999999e-2+t311.*5.267999999999999e-2+t535+t536+t1312+t1313+t1315+t1352+t1467+t1497+t1498+t1506+t1553+t1554+t1577;
et325 = -t3289+t3365.*2.2e-4+t3526+t3644+t3655-t3661-t3664+t2654.*(t884+t1578-t2180+t14.*(t639-t1128-t2181+dq5.*t13.*(t86-t652))).*1.089e-2;
et326 = t3336.*(t8.*(t92-t663)+t15.*(t621-t864)).*2.9e-4;
et327 = t450+t453+t469+t510+t530-t561-t562+t566+t596+t1837-t1952.*1.9738e-1+t2034-t2045+t2355+t2367-t2680.*1.9738e-1+t2718.*2.324e-2;
et328 = t3128.*(-3.466000000000001e-2)+t3129.*2.324e-2+t15.*(t284+t287+t290-t329-t805-t1951).*3.466000000000001e-2;
et329 = dq7.*t8.*(t252-t791).*3.466000000000001e-2;
et330 = t2717+t2776+t2794-t2672.*(t614+t13.*(t86-t652)).*4.466636216449161e-20-t632.*(t639-t1128-t2181+dq5.*t13.*(t86-t652)).*2.840000000000012e-3;
et331 = (t88-t617).*(t284+t287+t290-t329-t805-t1951).*(-1.0e-5)+t817.*t1070.*1.0e-5;
et332 = t607.*t2165.*(-2.840000000000012e-3)+t1206.*t1896.*2.840000000000012e-3;
et333 = t1295.*t1852.*2.840000000000012e-3+t633.*t2828.*2.840000000000012e-3;
et334 = t831.*t2671.*1.0e-5+t940.*t2832.*4.466636216449161e-20-t959.*t2816.*4.466636216449161e-20;
et335 = t2196.*(t90-t615).*(-4.466636216449161e-20)-t2147.*(t243-t786).*1.0e-5;
et336 = t2163.*(t252-t791).*(-1.0e-5)+t2659.*(t653-t838).*4.466636216449161e-20;
et337 = t94+t105+t494+t658.*1.9738e-1+t834.*2.324e-2+t837.*3.466000000000001e-2+t1634.*3.466000000000001e-2;
et338 = t15.*(t665+t7.*(t90-t615)).*(-2.324e-2)-t14.*(t90-t615).*1.9738e-1;
et339 = t2009+t10.*t569.*2.23e-3-t3.*t603.*2.23e-3;
et340 = t571.*t600.*4.999999999999997e-5+t568.*t605.*4.999999999999997e-5;
et341 = t572.*t840.*7.000000000000001e-5+t604.*t841.*7.000000000000001e-5;
et342 = t10.*t11.*t570.*(-7.000000000000001e-5)-t10.*t32.*t567.*4.999999999999997e-5;
et343 = t3.*t11.*t602.*7.000000000000001e-5-t10.*t29.*t601.*4.999999999999997e-5;
et344 = t9.*t10.*t818.*(-2.23e-3)-t2.*t10.*t842.*2.23e-3;
et345 = t3.*t9.*t1040.*2.23e-3+t10.*t31.*t1020.*7.000000000000001e-5;
et346 = t2.*t3.*t1066.*(-2.23e-3)+t10.*t35.*t1067.*7.000000000000001e-5;
et347 = t284.*2.75e-2+t287.*2.75e-2+t290.*2.75e-2+t450+t453+t469+t510+t530-t561-t562+t566+t596+t1455+t1740+t1775+t1782-t1951.*2.75e-2;
et348 = t1952.*2.019e-2+t1955.*4.9e-4+t1974+t1986+t2680.*2.019e-2-t2685.*4.9e-4;
et349 = t573.*t574.*(-1.11e-3)-t572.*t632.*8.8e-4;
et350 = t604.*t633.*8.8e-4+t676.*t831.*1.11e-3;
et351 = t677.*(t88-t617).*1.11e-3+t3.*t11.*t606.*1.144e-2;
et352 = t10.*t11.*t607.*(-8.8e-4)+t10.*t35.*t815.*1.144e-2;
et353 = t10.*t31.*(t86-t652).*1.144e-2;
et354 = t34.*(-5.267999999999999e-2)+t36.*2.0e-4+t75.*2.0e-4+t81.*5.267999999999999e-2+t105;
et355 = t3.*t11.*3.818e-2;
et356 = -t3206+t2000.*(t284+t287+t290-t329-t805-t1951).*5.0e-5-t1681.*(t884+t1578-t2180+t14.*(t639-t1128-t2181+dq5.*t13.*(t86-t652))).*3.0e-5;
et357 = t3124.*(t614+t13.*(t86-t652)).*5.000000000000004e-4+t3121.*(t1386+t7.*(t88-t617)).*3.0e-5;
et358 = t1296.*t2196.*5.000000000000004e-4-t1654.*t2816.*5.000000000000004e-4;
et359 = t1649.*t2832.*5.000000000000004e-4+t2035.*t2671.*5.0e-5;
et360 = t1685.*t3312.*3.0e-5-(t243-t786).*(t878-t1582+t2184+t7.*(t639-t1128-t2181+dq5.*t13.*(t86-t652))).*5.0e-5;
et361 = t2854.*(t92-t663).*5.000000000000004e-4+t2177.*(t621-t864).*5.0e-5;
et362 = t3120.*(t653-t838).*5.000000000000004e-4+(t665+t7.*(t90-t615)).*(t631-t885+t1132-t2224).*3.0e-5;
et363 = t817.*(t642+t896-t1137-t2220).*(-5.0e-5)+t2074.*(t755+t1012-t1905-t2692).*3.0e-5;
et364 = (t252-t791).*(t1487+t2219-t2864+dq6.*t7.*(t88-t617)).*(-5.0e-5);
et365 = t282.*1.8866e-1-t284.*2.37e-3+t285.*1.8866e-1-t287.*2.37e-3-t290.*2.37e-3;
et366 = t308.*5.000000000000001e-5+t310.*5.000000000000001e-5+t313.*5.000000000000001e-5-t328.*1.8866e-1+t459+t538+t1138+t1174+t1177+t1232+t1346+t1513+t1725+t1813;
et367 = t1949.*5.000000000000001e-5+t1951.*2.37e-3;
et368 = t274.*(-1.8866e-1)+t276.*2.37e-3+t277.*2.37e-3-t286.*5.000000000000001e-5;
et369 = t289.*(-5.000000000000001e-5)+t307.*1.8866e-1-t309.*2.37e-3+t311.*1.8866e-1;
et370 = t327.*5.000000000000001e-5+t465+t466+t1142+t1143+t1146+t1275+t1423+t1565+t1752+t1790-t1944.*5.000000000000001e-5-t1945.*2.37e-3;
et371 = -t3196-t3253-t3262+t3406+t3452+t2074.*(t878-t1582+t2184+t7.*(t639-t1128-t2181+dq5.*t13.*(t86-t652))).*3.0e-5+t2196.*(t621-t864).*5.0e-5;
et372 = t3312.*(t653-t838).*5.000000000000004e-4+t1207.*(t642+t896-t1137-t2220).*3.0e-5;
et373 = t2765+t2818-t2907+t3067+t3215+t3235-t3238-t3246+t3268-t3273+t3375+t3551-t3555+t3433.*(t614+t13.*(t86-t652)).*1.2e-4+t2147.*(t639-t1128-t2181+dq5.*t13.*(t86-t652)).*4.466636216449161e-20;
et374 = t2832.*(t639-t1128-t2181+dq5.*t13.*(t86-t652)).*1.2e-4+t2974.*(t92-t663).*1.2e-4;
et375 = t3422.*(t653-t838).*1.2e-4;
et376 = -t1980+t10.*t569.*7.000000000000001e-5-t3.*t603.*7.000000000000001e-5;
et377 = t571.*t600.*(-7.000000000000022e-5)-t568.*t605.*7.000000000000022e-5;
et378 = t572.*t840.*7.299999999999999e-4+t604.*t841.*7.299999999999999e-4;
et379 = t10.*t11.*t570.*(-7.299999999999999e-4)+t10.*t32.*t567.*7.000000000000022e-5;
et380 = t3.*t11.*t602.*7.299999999999999e-4+t10.*t29.*t601.*7.000000000000022e-5;
et381 = t9.*t10.*t818.*(-7.000000000000001e-5)-t2.*t10.*t842.*7.000000000000001e-5;
et382 = t3.*t9.*t1040.*7.000000000000001e-5+t10.*t31.*t1020.*7.299999999999999e-4;
et383 = t2.*t3.*t1066.*(-7.000000000000001e-5)+t10.*t35.*t1067.*7.299999999999999e-4;
et384 = t940.*(t614+t13.*(t86-t652)).*(-9.999999999999998e-6)+t573.*t817.*2.769999999999999e-3;
et385 = t607.*t827.*1.0e-5-t633.*t1206.*1.0e-5;
et386 = t632.*t1295.*1.0e-5+t831.*(t243-t786).*2.769999999999999e-3;
et387 = t959.*(t653-t838).*9.999999999999998e-6+(t90-t615).*(t92-t663).*9.999999999999998e-6;
et388 = (t88-t617).*(t252-t791).*2.769999999999999e-3;
et389 = t2473+t2494+t43.*t606.*1.144e-2-t51.*t607.*8.8e-4;
et390 = t58.*t607.*(-8.8e-4)-t64.*t606.*1.144e-2;
et391 = t137.*t815.*1.144e-2+t144.*t815.*1.144e-2;
et392 = t151.*t815.*1.144e-2+t574.*t1070.*1.11e-3;
et393 = t633.*t1040.*(-8.8e-4)+t632.*t1066.*8.8e-4;
et394 = t572.*t1852.*8.8e-4+t604.*t1896.*8.8e-4;
et395 = t831.*t1885.*1.11e-3+t676.*t2147.*1.11e-3;
et396 = t677.*t2163.*1.11e-3+t112.*(t86-t652).*1.144e-2;
et397 = t119.*(t86-t652).*1.144e-2-t171.*(t86-t652).*1.144e-2;
et398 = t1892.*(t88-t617).*1.11e-3+t3.*t11.*t1069.*1.144e-2;
et399 = t10.*t31.*t2148.*1.144e-2+t10.*t35.*t2164.*1.144e-2;
et400 = t4.*t27.*7.000000000000022e-5+t11.*t24.*7.000000000000001e-5;
et401 = t11.*t23.*t27.*7.000000000000001e-5+t11.*t26.*t27.*7.000000000000001e-5;
et402 = t3.*t9.*t571.*7.000000000000022e-5-t2.*t3.*t605.*7.000000000000022e-5;
et403 = t10.*t29.*t572.*7.299999999999999e-4-t10.*t32.*t604.*7.299999999999999e-4;
et404 = t3.*t4.*t10.*t11.*(-7.299999999999999e-4);
et405 = t1296.*(t1529+t15.*(t92-t663)).*(-2.2e-4)-t2075.*(t8.*(t92-t663)+t15.*(t621-t864)).*2.900000000000001e-4;
et406 = t1207.*t2036.*7.950000000000001e-3+t1654.*t2601.*2.2e-4;
et407 = t1649.*t2654.*(-2.2e-4)+t2074.*t2343.*7.950000000000001e-3;
et408 = t2323.*t2576.*(-2.900000000000001e-4)+t2326.*t2627.*2.900000000000001e-4;
et409 = (t1386+t7.*(t88-t617)).*(t1745+t8.*(t252-t791)).*7.950000000000001e-3;
et410 = t2473+t2494-t569.*t574.*1.144e-2+t603.*t606.*1.144e-2;
et411 = t815.*t818.*1.144e-2-t607.*t1069.*1.11e-3;
et412 = t677.*t1040.*(-1.144e-2)+t676.*t1066.*1.144e-2;
et413 = t572.*t1823.*8.8e-4+t604.*t1860.*8.8e-4;
et414 = t831.*t1855.*1.11e-3+t632.*t2148.*1.11e-3;
et415 = t633.*t2164.*1.11e-3+t842.*(t86-t652).*1.144e-2;
et416 = t1864.*(t88-t617).*1.11e-3-t3.*t11.*t1070.*8.8e-4;
et417 = t10.*t31.*t2147.*8.8e-4+t10.*t35.*t2163.*8.8e-4;
et418 = -t2009-t10.*t51.*4.46e-3+t11.*t208.*7.000000000000001e-5;
et419 = t37.*t571.*(-4.999999999999997e-5)+t63.*t571.*4.999999999999997e-5;
et420 = t46.*t605.*(-4.999999999999997e-5)-t49.*t605.*4.999999999999997e-5;
et421 = t97.*t572.*7.000000000000001e-5-t107.*t604.*7.000000000000001e-5;
et422 = t139.*t572.*(-7.000000000000001e-5)-t114.*t604.*7.000000000000001e-5;
et423 = t149.*t572.*(-7.000000000000001e-5)+t175.*t604.*7.000000000000001e-5;
et424 = dq3.*t4.*t24.*2.23e-3+dq3.*t11.*t27.*4.999999999999997e-5;
et425 = t4.*t11.*t69.*(-7.000000000000001e-5)+t10.*t23.*t51.*4.46e-3;
et426 = t10.*t26.*t51.*4.46e-3+t2.*t3.*t1020.*4.999999999999997e-5;
et427 = t3.*t9.*t1067.*4.999999999999997e-5+t10.*t32.*t1040.*7.000000000000001e-5;
et428 = t10.*t29.*t1066.*(-7.000000000000001e-5)-dq3.*t3.*t10.*t25.*7.000000000000001e-5;
et429 = dq3.*t3.*t10.*t28.*7.000000000000001e-5+dq3.*t4.*t23.*t27.*2.23e-3;
et430 = dq3.*t4.*t26.*t27.*2.23e-3;
et431 = t1207.*(t665+t7.*(t90-t615)).*(-2.32e-3)-t1649.*(t614+t13.*(t86-t652)).*3.0e-5;
et432 = t1685.*(t1386+t7.*(t88-t617)).*2.32e-3+t1681.*t2074.*2.32e-3;
et433 = t1296.*(t92-t663).*(-3.0e-5)+t817.*(t621-t864).*4.000000000000028e-5;
et434 = t2000.*(t252-t791).*(-4.000000000000028e-5)+t2035.*(t243-t786).*4.000000000000028e-5;
et435 = t1654.*(t653-t838).*3.0e-5;
et436 = -t3394+t3465-t2343.*(t884+t1578-t2180+t14.*(t639-t1128-t2181+dq5.*t13.*(t86-t652))).*2.2e-4+t2854.*(t1529+t15.*(t92-t663)).*1.089e-2;
et437 = t3470.*(t1386+t7.*(t88-t617)).*2.2e-4+t3312.*(t1745+t8.*(t252-t791)).*2.2e-4;
et438 = t1296.*t3336.*1.089e-2+t1649.*t3619.*1.089e-2;
et439 = t1654.*t3618.*(-1.089e-2)+t2601.*t3120.*1.089e-2;
et440 = t2654.*t3124.*1.089e-2-t2323.*t3617.*2.9e-4;
et441 = t2326.*t3620.*2.9e-4+t2576.*(t1755-t3128+t15.*(t284+t287+t290-t329-t805-t1951)+dq7.*t8.*(t252-t791)).*2.9e-4;
et442 = t2075.*(t958-t2263+dq7.*t1601+t15.*(t642+t896-t1137-t2220)).*(-2.9e-4)+t2074.*(t1036+t1771-t2690+t15.*(t755+t1012-t1905-t2692)).*2.2e-4;
et443 = t2627.*(t1034-t1750+t2691+t8.*(t755+t1012-t1905-t2692)).*2.9e-4-t2036.*(t631-t885+t1132-t2224).*2.2e-4;
et444 = -t2711+t2801-t2954+t2956-t3179+t3181+t2165.*(t92-t663).*4.466636216449161e-20+t2816.*(t88-t617).*1.0e-5;
et445 = t2828.*(t653-t838).*4.466636216449161e-20;
et446 = t83.*2.75e-2+t94+t105+t494+t620.*2.75e-2-t658.*2.019e-2-t665.*4.9e-4;
et447 = t7.*(t90-t615).*(-4.9e-4)+t14.*(t90-t615).*2.019e-2;
et448 = t2464+t2534-t569.*t574.*8.8e-4+t603.*t606.*8.8e-4;
et449 = t815.*t818.*8.8e-4-t607.*t1069.*1.12e-3;
et450 = t677.*t1040.*(-8.8e-4)+t676.*t1066.*8.8e-4;
et451 = t572.*t1823.*3.844e-2+t604.*t1860.*3.844e-2;
et452 = t831.*t1855.*1.12e-3+t632.*t2148.*1.12e-3;
et453 = t633.*t2164.*1.12e-3+t842.*(t86-t652).*8.8e-4;
et454 = t1864.*(t88-t617).*1.12e-3-t3.*t11.*t1070.*3.844e-2;
et455 = t10.*t31.*t2147.*3.844e-2+t10.*t35.*t2163.*3.844e-2;
et456 = t940.*(t614+t13.*(t86-t652)).*4.466636216449161e-20+t573.*t817.*1.0e-5;
et457 = t607.*t827.*2.840000000000012e-3-t633.*t1206.*2.840000000000012e-3;
et458 = t632.*t1295.*2.840000000000012e-3+t831.*(t243-t786).*1.0e-5;
et459 = t959.*(t653-t838).*(-4.466636216449161e-20)-(t90-t615).*(t92-t663).*4.466636216449161e-20;
et460 = (t88-t617).*(t252-t791).*1.0e-5;
et461 = t573.*t574.*(-4.988e-2)-t572.*t632.*1.12e-3;
et462 = t604.*t633.*1.12e-3+t676.*t831.*4.988e-2;
et463 = t677.*(t88-t617).*4.988e-2+t3.*t11.*t606.*1.11e-3;
et464 = t10.*t11.*t607.*(-1.12e-3)+t10.*t35.*t815.*1.11e-3;
et465 = t10.*t31.*(t86-t652).*1.11e-3;
et466 = t2717+t2776+t2794-t2630.*(t614+t13.*(t86-t652)).*4.466636216449161e-20-t607.*t2196.*1.0e-5+t817.*t2165.*4.466636216449161e-20;
et467 = t1206.*t1860.*2.840000000000012e-3+t940.*t2147.*2.840000000000012e-3;
et468 = t1295.*t1823.*2.840000000000012e-3+t959.*t2163.*2.840000000000012e-3;
et469 = t633.*t2816.*1.0e-5+t831.*t2631.*1.0e-5;
et470 = t632.*t2832.*(-1.0e-5)-(t243-t786).*(t639-t1128-t2181+dq5.*t13.*(t86-t652)).*4.466636216449161e-20;
et471 = t1070.*(t90-t615).*(-2.840000000000012e-3)+t2610.*(t88-t617).*1.0e-5;
et472 = t2828.*(t252-t791).*4.466636216449161e-20+t2609.*(t653-t838).*4.466636216449161e-20;
et473 = -t3291+t3365.*2.900000000000001e-4+t3527+t3642+t3654-t3662-t3665+t2654.*(t884+t1578-t2180+t14.*(t639-t1128-t2181+dq5.*t13.*(t86-t652))).*2.9e-4;
et474 = t3336.*(t8.*(t92-t663)+t15.*(t621-t864)).*2.94e-3;
et475 = t1207.*(t665+t7.*(t90-t615)).*3.0e-5+t1649.*(t614+t13.*(t86-t652)).*5.000000000000004e-4;
et476 = t1685.*(t1386+t7.*(t88-t617)).*(-3.0e-5)-t1681.*t2074.*3.0e-5;
et477 = t1296.*(t92-t663).*5.000000000000004e-4+t817.*(t621-t864).*5.0e-5;
et478 = t2000.*(t252-t791).*(-5.0e-5)+t2035.*(t243-t786).*5.0e-5;
et479 = t1654.*(t653-t838).*(-5.000000000000004e-4);
et480 = t3286+t3393-t2326.*(t884+t1578-t2180+t14.*(t639-t1128-t2181+dq5.*t13.*(t86-t652))).*2.9e-4-t3618.*(t1745+t8.*(t252-t791)).*2.94e-3;
et481 = t3313.*(t8.*(t92-t663)+t15.*(t621-t864)).*2.94e-3-(t1386+t7.*(t88-t617)).*(t1753+t2661+t3107-dq7.*t15.*(t252-t791)).*2.900000000000001e-4;
et482 = t1649.*t3620.*(-2.900000000000001e-4)+t1654.*t3617.*2.900000000000001e-4;
et483 = t2036.*t3336.*(-2.94e-3)+t2074.*t3460.*2.900000000000001e-4;
et484 = t2323.*t3312.*2.9e-4-t2601.*t3098.*2.9e-4;
et485 = t2654.*t3104.*(-2.9e-4)+t2343.*t3619.*2.94e-3;
et486 = t2576.*t3438.*2.94e-3+t1296.*(t958-t2263+dq7.*t1601+t15.*(t642+t896-t1137-t2220)).*2.900000000000001e-4;
et487 = t2627.*(t1034-t1750+t2667+t8.*(t755+t1012-t1873-t2664)).*(-2.94e-3)+t2075.*(t631-t885+t1132-t2224).*2.9e-4;
et488 = -t3289+t3365.*2.2e-4+t3526+t3644+t3655-t3661-t3664+t2654.*(t884+t1578-t2180+t14.*(t639-t1128-t2181+dq5.*t13.*(t86-t652))).*1.089e-2;
et489 = t3336.*(t8.*(t92-t663)+t15.*(t621-t864)).*2.9e-4;
et490 = t3287+t3399-t2326.*(t884+t1578-t2180+t14.*(t639-t1128-t2181+dq5.*t13.*(t86-t652))).*2.2e-4-t3618.*(t1745+t8.*(t252-t791)).*2.900000000000001e-4;
et491 = t3313.*(t8.*(t92-t663)+t15.*(t621-t864)).*2.900000000000001e-4-(t1386+t7.*(t88-t617)).*(t1753+t2661+t3107-dq7.*t15.*(t252-t791)).*7.950000000000001e-3;
et492 = t1649.*t3620.*(-7.950000000000001e-3)+t1654.*t3617.*7.950000000000001e-3;
et493 = t2036.*t3336.*(-2.900000000000001e-4)+t2074.*t3460.*7.950000000000001e-3;
et494 = t2323.*t3312.*2.2e-4-t2601.*t3098.*2.2e-4;
et495 = t2654.*t3104.*(-2.2e-4)+t2343.*t3619.*2.900000000000001e-4;
et496 = t2576.*t3438.*2.900000000000001e-4+t1296.*(t958-t2263+dq7.*t1601+t15.*(t642+t896-t1137-t2220)).*7.950000000000001e-3;
et497 = t2627.*(t1034-t1750+t2667+t8.*(t755+t1012-t1873-t2664)).*(-2.900000000000001e-4)+t2075.*(t631-t885+t1132-t2224).*2.2e-4;
et498 = -t1217+t572.*t1823+t604.*t1860-t3.*t11.*t1070+t10.*t31.*t2147+t10.*t35.*t2163;
et499 = (t2365+t2445.*1.12e-3-t2456+t2536-t2653-t2789+t2803+t2868+t1066.*(t86-t652).*8.8e-4).*(-1.0./2.0);
et500 = -t569.*t574+t603.*t606+t815.*t818-t677.*t1040+t676.*t1066+t842.*(t86-t652);
et501 = (t2388+t2445.*1.11e-3-t2467+t2496-t2693-t2798+t2810+t2829+t1066.*(t86-t652).*1.144e-2).*(-1.0./2.0);
et502 = t2924-t3210-t2000.*(t284+t287+t290-t329-t805-t1951).*4.000000000000028e-5-t1681.*(t884+t1578-t2180+t14.*(t639-t1128-t2181+dq5.*t13.*(t86-t652))).*2.32e-3;
et503 = t3124.*(t614+t13.*(t86-t652)).*3.0e-5+t3121.*(t1386+t7.*(t88-t617)).*2.32e-3;
et504 = t1296.*t2196.*3.0e-5-t1654.*t2816.*3.0e-5;
et505 = t1649.*t2832.*3.0e-5-t2035.*t2671.*4.000000000000028e-5;
et506 = t1685.*t3312.*2.32e-3+(t243-t786).*(t878-t1582+t2184+t7.*(t639-t1128-t2181+dq5.*t13.*(t86-t652))).*4.000000000000028e-5;
et507 = t2854.*(t92-t663).*3.0e-5+t3120.*(t653-t838).*3.0e-5;
et508 = (t665+t7.*(t90-t615)).*(t631-t885+t1132-t2224).*2.32e-3+t817.*(t642+t896-t1137-t2220).*4.000000000000028e-5;
et509 = t2074.*(t755+t1012-t1905-t2692).*2.32e-3+(t252-t791).*(t1487+t2219-t2864+dq6.*t7.*(t88-t617)).*4.000000000000028e-5;
et510 = -t3206+t1649.*(t878-t1582+t2184+t7.*(t639-t1128-t2181+dq5.*t13.*(t86-t652))).*3.0e-5-t2196.*(t665+t7.*(t90-t615)).*5.0e-5;
et511 = t3104.*(t614+t13.*(t86-t652)).*5.000000000000004e-4+t3099.*(t1386+t7.*(t88-t617)).*3.0e-5;
et512 = t1685.*t2816.*5.0e-5-t1681.*t2832.*5.0e-5;
et513 = t2000.*t2610.*(-5.0e-5)+t2035.*t2631.*5.0e-5;
et514 = (t243-t786).*(t884+t1578-t2180+t14.*(t639-t1128-t2181+dq5.*t13.*(t86-t652))).*(-5.000000000000004e-4)+t2854.*(t92-t663).*5.000000000000004e-4;
et515 = t2177.*(t621-t864).*5.0e-5+t3312.*(t252-t791).*5.000000000000004e-4;
et516 = t3098.*(t653-t838).*5.000000000000004e-4-t817.*(t631-t885+t1132-t2224).*5.000000000000004e-4;
et517 = t1296.*(t642+t896-t1137-t2220).*(-3.0e-5)+t2074.*(t755+t1012-t1873-t2664).*3.0e-5;
et518 = t1654.*(t1487+t2219-t2864+dq6.*t7.*(t88-t617)).*3.0e-5;
et519 = t2891+t2923+t2941+t3011-t3226+t3277-t3279-t3292+t3296-t3311+t3363+t3479.*1.0e-5+t3561+t3433.*(t614+t13.*(t86-t652)).*4.466636216449161e-20;
et520 = t2147.*(t639-t1128-t2181+dq5.*t13.*(t86-t652)).*2.840000000000012e-3+t2832.*(t639-t1128-t2181+dq5.*t13.*(t86-t652)).*4.466636216449161e-20;
et521 = t2974.*(t92-t663).*4.466636216449161e-20+t3422.*(t653-t838).*4.466636216449161e-20;
et522 = t439+t441+t444+t465+t466+t564+t565+t594+t595+t1834+t1901.*1.9738e-1+t2029+t2033+t2054+t2358+t2366-t2690.*2.324e-2-t2691.*3.466000000000001e-2;
et523 = t2694.*(-1.9738e-1)-t8.*(t755+t1012-t1905-t2692).*3.466000000000001e-2+t15.*(t755+t1012-t1905-t2692).*2.324e-2;
et524 = t272+t429+t556+t724.*1.9738e-1+t1008.*1.9738e-1+t1743.*3.466000000000001e-2-t1745.*2.324e-2;
et525 = t8.*(t252-t791).*(-2.324e-2)-t15.*(t252-t791).*3.466000000000001e-2;
et526 = t2681+t2791+t2827+t2672.*(t614+t13.*(t86-t652)).*9.999999999999998e-6-t632.*(t639-t1128-t2181+dq5.*t13.*(t86-t652)).*1.0e-5;
et527 = (t88-t617).*(t284+t287+t290-t329-t805-t1951).*(-2.769999999999999e-3)+t817.*t1070.*2.769999999999999e-3;
et528 = t607.*t2165.*(-1.0e-5)+t1206.*t1896.*1.0e-5;
et529 = t1295.*t1852.*1.0e-5+t633.*t2828.*1.0e-5;
et530 = t831.*t2671.*2.769999999999999e-3-t940.*t2832.*9.999999999999998e-6;
et531 = t959.*t2816.*9.999999999999998e-6+t2196.*(t90-t615).*9.999999999999998e-6;
et532 = t2147.*(t243-t786).*(-2.769999999999999e-3)-t2163.*(t252-t791).*2.769999999999999e-3;
et533 = t2659.*(t653-t838).*(-9.999999999999998e-6);
et534 = t24.*4.200000000000139e-4+t23.*t27.*4.200000000000139e-4;
et535 = t26.*t27.*4.200000000000139e-4;
et536 = t940.*(t614+t13.*(t86-t652)).*(-1.2e-4)+t573.*t817.*9.999999999999998e-6;
et537 = t607.*t827.*(-4.466636216449161e-20)+t633.*t1206.*4.466636216449161e-20-t632.*t1295.*4.466636216449161e-20;
et538 = t831.*(t243-t786).*9.999999999999998e-6+t959.*(t653-t838).*1.2e-4;
et539 = (t90-t615).*(t92-t663).*1.2e-4+(t88-t617).*(t252-t791).*9.999999999999998e-6;
et540 = t231.*1.16152294893368e-19+t232.*1.16152294893368e-19+t622.*8.909980864224564e-21;
et541 = t688.*(-4.200000000000139e-4)+t701.*4.200000000000139e-4;
et542 = t707.*8.909980864224564e-21+t769.*4.200000000000139e-4;
et543 = t770.*4.200000000000139e-4-t845.*8.909980864224564e-21+t867.*8.909980864224564e-21;
et544 = t873.*(-4.200000000000139e-4)-t905.*4.200000000000139e-4;
et545 = t3.*t10.*t17.*8.400000000000278e-4;
et546 = t1207.*(t665+t7.*(t90-t615)).*(-4.000000000000028e-5)+t1649.*(t614+t13.*(t86-t652)).*5.0e-5;
et547 = t1685.*(t1386+t7.*(t88-t617)).*4.000000000000028e-5+t1681.*t2074.*4.000000000000028e-5;
et548 = t1296.*(t92-t663).*5.0e-5+t817.*(t621-t864).*2.81e-3;
et549 = t2000.*(t252-t791).*(-2.81e-3)+t2035.*(t243-t786).*2.81e-3;
et550 = t1654.*(t653-t838).*(-5.0e-5);
et551 = t276.*2.75e-2+t277.*2.75e-2-t309.*2.75e-2+t439+t441+t444+t465+t466+t564+t565+t594+t595+t1449+t1735+t1773+t1780-t1901.*2.019e-2;
et552 = t1905.*(-4.9e-4)-t1945.*2.75e-2+t1970+t1984-t2692.*4.9e-4+t2694.*2.019e-2;
et553 = t2464+t2534+t43.*t606.*8.8e-4-t51.*t607.*3.844e-2;
et554 = t58.*t607.*(-3.844e-2)-t64.*t606.*8.8e-4;
et555 = t137.*t815.*8.8e-4+t144.*t815.*8.8e-4;
et556 = t151.*t815.*8.8e-4+t574.*t1070.*1.12e-3;
et557 = t633.*t1040.*(-3.844e-2)+t632.*t1066.*3.844e-2;
et558 = t572.*t1852.*3.844e-2+t604.*t1896.*3.844e-2;
et559 = t831.*t1885.*1.12e-3+t676.*t2147.*1.12e-3;
et560 = t677.*t2163.*1.12e-3+t112.*(t86-t652).*8.8e-4;
et561 = t119.*(t86-t652).*8.8e-4-t171.*(t86-t652).*8.8e-4;
et562 = t1892.*(t88-t617).*1.12e-3+t3.*t11.*t1069.*8.8e-4;
et563 = t10.*t31.*t2148.*8.8e-4+t10.*t35.*t2164.*8.8e-4;
et564 = t1980-t10.*t51.*1.4e-4+t11.*t208.*7.299999999999999e-4;
et565 = t37.*t571.*7.000000000000022e-5-t63.*t571.*7.000000000000022e-5;
et566 = t46.*t605.*7.000000000000022e-5+t49.*t605.*7.000000000000022e-5;
et567 = t97.*t572.*7.299999999999999e-4-t107.*t604.*7.299999999999999e-4;
et568 = t139.*t572.*(-7.299999999999999e-4)-t114.*t604.*7.299999999999999e-4;
et569 = t149.*t572.*(-7.299999999999999e-4)+t175.*t604.*7.299999999999999e-4;
et570 = dq3.*t4.*t24.*7.000000000000001e-5-dq3.*t11.*t27.*7.000000000000022e-5;
et571 = t4.*t11.*t69.*(-7.299999999999999e-4)+t10.*t23.*t51.*1.4e-4;
et572 = t10.*t26.*t51.*1.4e-4-t2.*t3.*t1020.*7.000000000000022e-5;
et573 = t3.*t9.*t1067.*(-7.000000000000022e-5)+t10.*t32.*t1040.*7.299999999999999e-4;
et574 = t10.*t29.*t1066.*(-7.299999999999999e-4)-dq3.*t3.*t10.*t25.*7.299999999999999e-4;
et575 = dq3.*t3.*t10.*t28.*7.299999999999999e-4+dq3.*t4.*t23.*t27.*7.000000000000001e-5;
et576 = dq3.*t4.*t26.*t27.*7.000000000000001e-5;
et577 = t1736+t9.*t568.*5.582083966615414e-19+t2.*t600.*5.582083966615414e-19-dq1.*t10.*t23.*1.0e-4;
et578 = dq1.*t10.*t26.*(-1.0e-4)+t2.*t3.*t568.*1.16152294893368e-19+t9.*t10.*t567.*1.16152294893368e-19;
et579 = t3.*t9.*t600.*(-1.16152294893368e-19)+t2.*t10.*t601.*1.16152294893368e-19;
et580 = t1627-t607.*t1069+t831.*t1855+t632.*t2148+t633.*t2164+t1864.*(t88-t617);
et581 = (t2341+t2445.*4.988e-2-t2463-t2612+t2624-t2796+t2813+t2900+t1066.*(t86-t652).*1.11e-3).*(-1.0./2.0);
et582 = t1627+t574.*t1070+t831.*t1885+t676.*t2147+t677.*t2163+t1892.*(t88-t617);
et583 = (t2341+t2445.*4.988e-2-t2463-t2612+t2624-t2796+t2813+t2900+t1066.*(t86-t652).*1.11e-3)./2.0;
et584 = t74.*5.267999999999999e-2-t78.*2.0e-4+t240.*2.0e-4+t241.*5.267999999999999e-2-t267;
et585 = t10.*t31.*3.818e-2;
et586 = t80.*5.267999999999999e-2-t87.*2.0e-4+t242.*2.0e-4+t250.*5.267999999999999e-2-t272;
et587 = t10.*t35.*3.818e-2;
et588 = t439+t441+t444+t465+t466+t595+t972+t1834+t1871.*1.9738e-1+t2029+t2033+t2054+t2358+t2366-t2665.*2.324e-2-t2666.*1.9738e-1;
et589 = t2667.*(-3.466000000000001e-2)-t8.*(t755+t1012-t1873-t2664).*3.466000000000001e-2+t15.*(t755+t1012-t1873-t2664).*2.324e-2;
et590 = t1296.*(t1529+t15.*(t92-t663)).*(-2.9e-4)-t2075.*(t8.*(t92-t663)+t15.*(t621-t864)).*2.94e-3;
et591 = t1207.*t2036.*2.900000000000001e-4+t1654.*t2601.*2.9e-4;
et592 = t1649.*t2654.*(-2.9e-4)+t2074.*t2343.*2.900000000000001e-4;
et593 = t2323.*t2576.*(-2.94e-3)+t2326.*t2627.*2.94e-3;
et594 = (t1386+t7.*(t88-t617)).*(t1745+t8.*(t252-t791)).*2.900000000000001e-4;
et595 = t2388+t2445.*1.11e-3-t2467+t2496-t2693-t2798+t2810+t2829+t1066.*(t86-t652).*1.144e-2;
et596 = (t43.*t606+t187.*t606+t137.*t815+t144.*t815+t151.*t815+t112.*(t86-t652)+t119.*(t86-t652)+t338.*(t86-t652)+t3.*t11.*t1069+t10.*t31.*t2148+t10.*t35.*t2164)./2.0;
et597 = t3285+t3394-t2326.*(t884+t1578-t2180+t14.*(t639-t1128-t2181+dq5.*t13.*(t86-t652))).*1.089e-2-t3618.*(t1745+t8.*(t252-t791)).*2.9e-4;
et598 = t3313.*(t8.*(t92-t663)+t15.*(t621-t864)).*2.9e-4-(t1386+t7.*(t88-t617)).*(t1753+t2661+t3107-dq7.*t15.*(t252-t791)).*2.2e-4;
et599 = t1649.*t3620.*(-2.2e-4)+t1654.*t3617.*2.2e-4;
et600 = t2036.*t3336.*(-2.9e-4)+t2074.*t3460.*2.2e-4;
et601 = t2323.*t3312.*1.089e-2-t2601.*t3098.*1.089e-2;
et602 = t2654.*t3104.*(-1.089e-2)+t2343.*t3619.*2.9e-4;
et603 = t2576.*t3438.*2.9e-4+t1296.*(t958-t2263+dq7.*t1601+t15.*(t642+t896-t1137-t2220)).*2.2e-4;
et604 = t2627.*(t1034-t1750+t2667+t8.*(t755+t1012-t1873-t2664)).*(-2.9e-4)+t2075.*(t631-t885+t1132-t2224).*1.089e-2;
et605 = -t2711+t2801-t2954+t2956-t3179+t3181+t2165.*(t92-t663).*4.466636216449161e-20+t2816.*(t88-t617).*1.0e-5;
et606 = t2828.*(t653-t838).*4.466636216449161e-20;
et607 = t2018+t9.*t568.*8.909980864224564e-21+t2.*t600.*8.909980864224564e-21-dq1.*t10.*t23.*1.16152294893368e-19;
et608 = dq1.*t10.*t26.*(-1.16152294893368e-19)+t2.*t3.*t568.*4.200000000000139e-4;
et609 = t9.*t10.*t567.*4.200000000000139e-4-t3.*t9.*t600.*4.200000000000139e-4;
et610 = t2.*t10.*t601.*4.200000000000139e-4;
et611 = t439+t441+t444+t465+t466+t595+t890.*2.75e-2+t972+t1449+t1735+t1773+t1780-t1871.*2.019e-2-t1873.*4.9e-4-t1907.*2.75e-2+t1970+t1984;
et612 = t2664.*(-4.9e-4)+t2666.*2.019e-2;
et613 = t4.*t27.*(-2.19e-3)+t11.*t24.*4.999999999999997e-5;
et614 = t11.*t23.*t27.*4.999999999999997e-5+t11.*t26.*t27.*4.999999999999997e-5;
et615 = t3.*t9.*t571.*(-2.19e-3)+t2.*t3.*t605.*2.19e-3;
et616 = t10.*t29.*t572.*(-7.000000000000022e-5)+t10.*t32.*t604.*7.000000000000022e-5;
et617 = t3.*t4.*t10.*t11.*7.000000000000022e-5;
et618 = t2924-t3210+t1649.*(t878-t1582+t2184+t7.*(t639-t1128-t2181+dq5.*t13.*(t86-t652))).*2.32e-3+t2196.*(t665+t7.*(t90-t615)).*4.000000000000028e-5;
et619 = t3104.*(t614+t13.*(t86-t652)).*3.0e-5+t3099.*(t1386+t7.*(t88-t617)).*2.32e-3;
et620 = t1685.*t2816.*(-4.000000000000028e-5)+t1681.*t2832.*4.000000000000028e-5;
et621 = t2000.*t2610.*4.000000000000028e-5-t2035.*t2631.*4.000000000000028e-5;
et622 = (t243-t786).*(t884+t1578-t2180+t14.*(t639-t1128-t2181+dq5.*t13.*(t86-t652))).*(-3.0e-5)+t2854.*(t92-t663).*3.0e-5;
et623 = t3312.*(t252-t791).*3.0e-5+t3098.*(t653-t838).*3.0e-5;
et624 = t817.*(t631-t885+t1132-t2224).*(-3.0e-5)-t1296.*(t642+t896-t1137-t2220).*2.32e-3;
et625 = t2074.*(t755+t1012-t1873-t2664).*2.32e-3+t1654.*(t1487+t2219-t2864+dq6.*t7.*(t88-t617)).*2.32e-3;
et626 = t435+t459+t524+t526+t538+t563+t973+t1850+t1909.*1.9738e-1+t2011+t2045+t2049+t2362+t2371+t2641.*2.324e-2+t2642.*1.9738e-1+t2643.*3.466000000000001e-2;
et627 = t3106.*3.466000000000001e-2-t3107.*2.324e-2;
et628 = -t3294+t3365.*7.950000000000001e-3+t3528+t3648+t3658-t3660-t3663+t2654.*(t884+t1578-t2180+t14.*(t639-t1128-t2181+dq5.*t13.*(t86-t652))).*2.2e-4;
et629 = t3336.*(t8.*(t92-t663)+t15.*(t621-t864)).*2.900000000000001e-4;
et630 = t2681+t2791+t2827+t2630.*(t614+t13.*(t86-t652)).*9.999999999999998e-6-t607.*t2196.*2.769999999999999e-3;
et631 = t817.*t2165.*(-9.999999999999998e-6)+t1206.*t1860.*1.0e-5;
et632 = t940.*t2147.*1.0e-5+t1295.*t1823.*1.0e-5;
et633 = t959.*t2163.*1.0e-5+t633.*t2816.*2.769999999999999e-3;
et634 = t831.*t2631.*2.769999999999999e-3-t632.*t2832.*2.769999999999999e-3;
et635 = (t243-t786).*(t639-t1128-t2181+dq5.*t13.*(t86-t652)).*9.999999999999998e-6-t1070.*(t90-t615).*1.0e-5;
et636 = t2610.*(t88-t617).*2.769999999999999e-3-t2828.*(t252-t791).*9.999999999999998e-6;
et637 = t2609.*(t653-t838).*(-9.999999999999998e-6);
et638 = t1751+t9.*t568.*3.199999999999801e-4+t2.*t600.*3.199999999999801e-4;
et639 = dq1.*t10.*t23.*(-5.582083966615414e-19)-dq1.*t10.*t26.*5.582083966615414e-19+t2.*t3.*t568.*8.909980864224564e-21;
et640 = t9.*t10.*t567.*8.909980864224564e-21-t3.*t9.*t600.*8.909980864224564e-21+t2.*t10.*t601.*8.909980864224564e-21;
et641 = t459+t538-t854.*2.37e-3+t856.*5.000000000000001e-5+t899.*1.8866e-1+t1138+t1174+t1177+t1232+t1346+t1513+t1725+t1813+t1912.*5.000000000000001e-5;
et642 = t1918.*2.37e-3;
et643 = t465+t466+t889.*1.8866e-1+t890.*2.37e-3-t900.*5.000000000000001e-5+t1142+t1143+t1146+t1275+t1423+t1565+t1752+t1790-t1903.*5.000000000000001e-5;
et644 = t1907.*(-2.37e-3);
et645 = -t3399+t3464-t2343.*(t884+t1578-t2180+t14.*(t639-t1128-t2181+dq5.*t13.*(t86-t652))).*7.950000000000001e-3+t2854.*(t1529+t15.*(t92-t663)).*2.2e-4;
et646 = t3470.*(t1386+t7.*(t88-t617)).*7.950000000000001e-3+t3312.*(t1745+t8.*(t252-t791)).*7.950000000000001e-3;
et647 = t1296.*t3336.*2.2e-4+t1649.*t3619.*2.2e-4;
et648 = t1654.*t3618.*(-2.2e-4)+t2601.*t3120.*2.2e-4;
et649 = t2654.*t3124.*2.2e-4-t2323.*t3617.*2.900000000000001e-4;
et650 = t2326.*t3620.*2.900000000000001e-4+t2576.*(t1755-t3128+t15.*(t284+t287+t290-t329-t805-t1951)+dq7.*t8.*(t252-t791)).*2.900000000000001e-4;
et651 = t2075.*(t958-t2263+dq7.*t1601+t15.*(t642+t896-t1137-t2220)).*(-2.900000000000001e-4)+t2074.*(t1036+t1771-t2690+t15.*(t755+t1012-t1905-t2692)).*7.950000000000001e-3;
et652 = t2627.*(t1034-t1750+t2691+t8.*(t755+t1012-t1905-t2692)).*2.900000000000001e-4-t2036.*(t631-t885+t1132-t2224).*7.950000000000001e-3;
et653 = t267+t427+t553+t722.*1.9738e-1+t1004.*1.9738e-1-t1044.*2.324e-2+t1732.*3.466000000000001e-2;
et654 = t1737.*(-2.324e-2)-t15.*(t243-t786).*3.466000000000001e-2;
et655 = -t2443-t2780-t2630.*(t614+t13.*(t86-t652)).*1.2e-4+t607.*t2196.*9.999999999999998e-6;
et656 = t817.*t2165.*1.2e-4+t1206.*t1860.*4.466636216449161e-20+t940.*t2147.*4.466636216449161e-20;
C = ft_9({dq1,dq2,dq3,dq4,dq5,dq6,dq7,et217,et218,et219,et220,et221,et222,et223,et224,et225,et226,et227,et228,et229,et230,et231,et232,et233,et234,et235,et236,et237,et238,et239,et240,et241,et242,et243,et244,et245,et246,et247,et248,et249,et250,et251,et252,et253,et254,et255,et256,et257,et258,et259,et260,et261,et262,et263,et264,et265,et266,et267,et268,et269,et270,et271,et272,et273,et274,et275,et276,et277,et278,et279,et280,et281,et282,et283,et284,et285,et286,et287,et288,et289,et290,et291,et292,et293,et294,et295,et296,et297,et298,et299,et300,et301,et302,et303,et304,et305,et306,et307,et308,et309,et310,et311,et312,et313,et314,et315,et316,et317,et318,et319,et320,et321,et322,et323,et324,et325,et326,et327,et328,et329,et330,et331,et332,et333,et334,et335,et336,et337,et338,et339,et340,et341,et342,et343,et344,et345,et346,et347,et348,et349,et350,et351,et352,et353,et354,et355,et356,et357,et358,et359,et360,et361,et362,et363,et364,et365,et366,et367,et368,et369,et370,et371,et372,et373,et374,et375,et376,et377,et378,et379,et380,et381,et382,et383,et384,et385,et386,et387,et388,et389,et390,et391,et392,et393,et394,et395,et396,et397,et398,et399,et400,et401,et402,et403,et404,et405,et406,et407,et408,et409,et410,et411,et412,et413,et414,et415,et416,et417,et418,et419,et420,et421,et422,et423,et424,et425,et426,et427,et428,et429,et430,et431,et432,et433,et434,et435,et436,et437,et438,et439,et440,et441,et442,et443,et444,et445,et446,et447,et448,et449,et450,et451,et452,et453,et454,et455,et456,et457,et458,et459,et460,et461,et462,et463,et464,et465,et466,et467,et468,et469,et470,et471,et472,et473,et474,et475,et476,et477,et478,et479,et480,et481,et482,et483,et484,et485,et486,et487,et488,et489,et490,et491,et492,et493,et494,et495,et496,et497,et498,et499,et500,et501,et502,et503,et504,et505,et506,et507,et508,et509,et510,et511,et512,et513,et514,et515,et516,et517,et518,et519,et520,et521,et522,et523,et524,et525,et526,et527,et528,et529,et530,et531,et532,et533,et534,et535,et536,et537,et538,et539,et540,et541,et542,et543,et544,et545,et546,et547,et548,et549,et550,et551,et552,et553,et554,et555,et556,et557,et558,et559,et560,et561,et562,et563,et564,et565,et566,et567,et568,et569,et570,et571,et572,et573,et574,et575,et576,et577,et578,et579,et580,et581,et582,et583,et584,et585,et586,et587,et588,et589,et590,et591,et592,et593,et594,et595,et596,et597,et598,et599,et600,et601,et602,et603,et604,et605,et606,et607,et608,et609,et610,et611,et612,et613,et614,et615,et616,et617,et618,et619,et620,et621,et622,et623,et624,et625,et626,et627,et628,et629,et630,et631,et632,et633,et634,et635,et636,et637,et638,et639,et640,et641,et642,et643,et644,et645,et646,et647,et648,et649,et650,et651,et652,et653,et654,et655,et656,t10,t1001,t1012,t1015,t1016,t1017,t1018,t1020,t1021,t1022,t1023,t1024,t1025,t1034,t1036,t1040,t1041,t1051,t1052,t1053,t1054,t1055,t1056,t1059,t1060,t1066,t1067,t1069,t107,t1070,t1072,t1075,t1077,t1079,t1081,t1088,t1093,t1094,t1096,t1097,t11,t1110,t1113,t1114,t1115,t1123,t1125,t1126,t1128,t1130,t1132,t1136,t1137,t114,t1159,t1161,t1172,t1175,t1178,t1179,t1189,t1190,t12,t1206,t1207,t1209,t1211,t1212,t1213,t1214,t1215,t1218,t1219,t122,t1220,t1226,t1231,t1256,t1267,t1268,t1269,t1273,t1286,t1295,t1296,t1299,t13,t130,t1304,t1312,t1313,t1315,t1329,t1330,t1339,t1347,t1350,t1351,t1352,t1360,t1368,t1369,t1374,t1375,t1386,t1387,t1389,t139,t1391,t14,t1424,t1431,t1435,t1441,t1456,t1462,t1467,t1487,t1489,t149,t1497,t1498,t15,t1506,t1515,t1516,t152,t1526,t1528,t1529,t1543,t1546,t1553,t1554,t1569,t1574,t1577,t1578,t1579,t1581,t1582,t1591,t160,t1601,t1603,t1604,t1605,t1616,t1622,t1625,t1633,t1635,t1636,t1638,t1643,t1644,t1648,t1649,t165,t1654,t1655,t1657,t1658,t1660,t1661,t1662,t1667,t1668,t1672,t1675,t1679,t1681,t1682,t1685,t1686,t1687,t1688,t1697,t17,t1700,t1701,t1702,t1707,t1710,t1711,t1715,t1717,t1718,t1719,t1720,t1721,t1723,t1726,t1729,t1734,t1736,t1738,t1742,t1745,t1746,t1748,t1749,t1750,t1751,t1753,t1755,t1760,t1762,t1765,t1766,t1769,t1770,t1771,t1772,t1774,t1776,t1778,t1779,t1791,t1792,t1795,t1798,t1799,t180,t1800,t1801,t1802,t1804,t1805,t1806,t1811,t1812,t1814,t1816,t1817,t1819,t182,t1822,t1823,t1830,t1836,t1839,t1840,t1842,t1843,t1846,t1849,t1851,t1852,t1853,t1856,t1859,t186,t1860,t1861,t1863,t1865,t1866,t1867,t1872,t1873,t1874,t1875,t1876,t1880,t1881,t1883,t1886,t1888,t1889,t189,t1890,t1893,t1896,t1898,t1902,t1905,t1908,t1911,t1914,t1917,t1919,t1924,t1927,t1928,t1931,t1932,t1934,t1940,t1942,t1950,t1951,t1953,t1957,t1959,t1960,t1962,t1963,t1969,t1976,t1985,t1993,t2,t2000,t2001,t2002,t2003,t2006,t2008,t2010,t2018,t2022,t2026,t2035,t2036,t2041,t2042,t2044,t2046,t2051,t2056,t2058,t2065,t2066,t2071,t2072,t2073,t2074,t2075,t2076,t208,t2080,t2081,t2085,t2088,t2089,t2090,t2095,t2096,t2108,t2109,t2111,t2115,t2119,t2125,t2130,t2139,t2147,t2148,t2149,t2151,t2152,t2163,t2164,t2165,t2171,t2173,t2177,t2179,t2180,t2181,t2182,t2183,t2184,t2187,t2196,t2198,t2203,t2205,t2206,t2207,t2208,t221,t2212,t2215,t2217,t2219,t2220,t2224,t2227,t2228,t223,t2231,t2240,t2246,t2253,t2256,t2258,t2259,t2261,t2262,t2263,t2264,t2266,t2269,t2289,t2296,t23,t230,t2300,t2301,t2315,t2323,t2326,t2330,t234,t2341,t2343,t235,t2350,t2351,t2352,t2356,t2357,t2359,t236,t2360,t2363,t2365,t2369,t237,t2370,t2372,t2374,t2375,t2376,t2379,t238,t2380,t2382,t2383,t2384,t2385,t2387,t2388,t239,t2392,t2393,t2395,t2399,t24,t2400,t2402,t2404,t2407,t2411,t2418,t2429,t243,t2435,t2439,t244,t2444,t2445,t2447,t2455,t2456,t2460,t2462,t2463,t2466,t2467,t2477,t2482,t2483,t2488,t2496,t25,t2501,t2503,t2507,t2513,t2514,t2516,t252,t2521,t2522,t2523,t253,t2533,t2536,t2537,t254,t2541,t2554,t2558,t2560,t2561,t2563,t2569,t2570,t2571,t2576,t2581,t2584,t2585,t2587,t259,t2590,t2591,t26,t2601,t2602,t2604,t2609,t2610,t2611,t2612,t2613,t2614,t2615,t2617,t2618,t2620,t2621,t2624,t2627,t2631,t2634,t2635,t2637,t2638,t2647,t2648,t2651,t2652,t2653,t2654,t2655,t2656,t2659,t2661,t2662,t2663,t2664,t2667,t2670,t2671,t2672,t2674,t2675,t2677,t2679,t268,t2684,t2687,t2689,t269,t2690,t2691,t2692,t2693,t2697,t2698,t2699,t27,t2700,t2701,t2703,t2707,t2708,t2710,t2711,t2714,t2720,t2721,t2722,t2723,t2726,t2727,t2728,t2729,t2732,t2734,t2735,t2737,t2738,t2739,t2740,t2741,t2742,t2743,t2744,t2747,t2751,t2753,t2754,t2756,t2765,t2781,t2783,t2788,t2789,t279,t2790,t2792,t2795,t2796,t2797,t2798,t2799,t28,t280,t2801,t2803,t2804,t2807,t2810,t2811,t2813,t2814,t2816,t2817,t2818,t2823,t2825,t2828,t2829,t2832,t2837,t2838,t2839,t284,t2840,t2841,t2842,t2844,t2854,t2857,t2861,t2864,t2868,t287,t2883,t2884,t2891,t29,t290,t2900,t2907,t2914,t2922,t2923,t2925,t293,t2930,t2931,t2935,t2936,t2939,t2941,t2942,t2943,t2944,t2945,t2946,t2948,t2949,t295,t2950,t2953,t2954,t2955,t2956,t2957,t296,t2960,t2961,t2962,t297,t2972,t2974,t298,t2989,t2991,t2996,t2997,t2998,t2999,t3,t30,t3008,t3009,t301,t3011,t3020,t3031,t3035,t3038,t3039,t3040,t3041,t3042,t3045,t3047,t3048,t3051,t3052,t3060,t3066,t3067,t3071,t3075,t3076,t3082,t3083,t3085,t3086,t3088,t3092,t3097,t3098,t3099,t31,t3104,t3107,t3112,t3113,t3120,t3121,t3122,t3124,t3126,t3128,t3130,t3131,t3132,t3133,t3140,t3141,t3142,t3143,t3148,t3152,t3153,t3154,t3155,t3159,t3161,t3162,t3163,t3165,t3166,t3168,t317,t3170,t3171,t3172,t3175,t3179,t318,t3181,t3186,t319,t3190,t3192,t3193,t3194,t3195,t3196,t32,t320,t3201,t3202,t3203,t3204,t3205,t3215,t3226,t3229,t3232,t3235,t3238,t3246,t3248,t3249,t3252,t3253,t3255,t3257,t3260,t3261,t3262,t3263,t3264,t3268,t3269,t3272,t3273,t3277,t3279,t3280,t3284,t3288,t3289,t329,t3290,t3291,t3292,t3293,t3294,t3295,t3296,t33,t330,t3301,t331,t3311,t3312,t3313,t3315,t3316,t3321,t3324,t3336,t3340,t3342,t3356,t3357,t3358,t3359,t3360,t3361,t3362,t3363,t3364,t3365,t3366,t3369,t3372,t3375,t3377,t3382,t3384,t3386,t3388,t3392,t3393,t3395,t3397,t3398,t34,t3400,t3402,t3403,t3406,t3407,t3411,t3413,t3414,t3417,t3418,t342,t3421,t3422,t3424,t3426,t3429,t3433,t3436,t3437,t3438,t3440,t3443,t3444,t3452,t346,t3460,t3468,t3470,t3476,t3479,t3480,t3481,t3482,t3483,t3486,t3488,t3489,t349,t3490,t3491,t3492,t3495,t3498,t35,t3502,t3504,t3506,t3514,t3526,t3527,t3528,t3535,t3536,t3537,t3538,t3540,t3542,t3544,t3546,t3547,t3551,t3555,t3556,t3559,t3561,t36,t3610,t3617,t3618,t3619,t3620,t3625,t3626,t3627,t3628,t3640,t3641,t3642,t3643,t3644,t3645,t3646,t3648,t3649,t3651,t3652,t3653,t3654,t3655,t3658,t3660,t3661,t3662,t3663,t3664,t3665,t3666,t3667,t3668,t3669,t3670,t3671,t3672,t3673,t3674,t3679,t3685,t37,t3720,t3751,t3776,t3779,t3780,t3781,t3782,t3783,t3784,t3786,t3788,t3789,t3790,t3796,t3798,t3811,t3812,t3816,t3818,t3820,t3821,t3823,t3824,t3825,t3826,t3828,t3829,t3833,t3835,t3838,t3839,t3840,t3841,t3842,t3843,t3844,t3845,t39,t4,t40,t431,t433,t436,t448,t45,t451,t452,t455,t456,t457,t458,t46,t460,t461,t463,t469,t49,t5,t50,t51,t512,t515,t516,t517,t518,t522,t523,t525,t527,t528,t529,t530,t535,t536,t537,t542,t547,t548,t55,t554,t567,t568,t569,t57,t570,t571,t572,t573,t574,t58,t580,t581,t583,t6,t600,t601,t602,t603,t604,t605,t606,t607,t608,t609,t61,t612,t613,t614,t615,t616,t617,t618,t619,t621,t624,t626,t629,t631,t632,t633,t634,t635,t637,t639,t640,t642,t643,t644,t646,t647,t648,t649,t650,t651,t652,t653,t654,t656,t657,t660,t661,t662,t663,t664,t665,t667,t67,t673,t676,t677,t678,t685,t687,t689,t69,t691,t692,t693,t694,t696,t697,t698,t7,t70,t702,t703,t704,t705,t708,t71,t72,t721,t725,t726,t729,t73,t730,t731,t735,t743,t754,t755,t756,t76,t760,t762,t77,t773,t774,t776,t777,t778,t786,t788,t79,t791,t792,t795,t796,t797,t8,t800,t805,t806,t813,t815,t817,t818,t819,t82,t827,t831,t835,t836,t838,t839,t84,t840,t841,t842,t843,t846,t847,t85,t853,t855,t857,t859,t86,t860,t863,t864,t866,t870,t871,t876,t877,t878,t88,t880,t881,t882,t884,t885,t888,t889,t89,t891,t896,t898,t899,t9,t90,t902,t907,t908,t91,t911,t92,t921,t926,t927,t928,t930,t932,t933,t935,t939,t940,t942,t948,t949,t952,t958,t959,t966,t969,t974,t975,t982,t983,t984,t987,t988,t992,t994});
end
function C = ft_9(ct)
dq1 = ct{1};
dq2 = ct{2};
dq3 = ct{3};
dq4 = ct{4};
dq5 = ct{5};
dq6 = ct{6};
dq7 = ct{7};
et217 = ct{8};
et218 = ct{9};
et219 = ct{10};
et220 = ct{11};
et221 = ct{12};
et222 = ct{13};
et223 = ct{14};
et224 = ct{15};
et225 = ct{16};
et226 = ct{17};
et227 = ct{18};
et228 = ct{19};
et229 = ct{20};
et230 = ct{21};
et231 = ct{22};
et232 = ct{23};
et233 = ct{24};
et234 = ct{25};
et235 = ct{26};
et236 = ct{27};
et237 = ct{28};
et238 = ct{29};
et239 = ct{30};
et240 = ct{31};
et241 = ct{32};
et242 = ct{33};
et243 = ct{34};
et244 = ct{35};
et245 = ct{36};
et246 = ct{37};
et247 = ct{38};
et248 = ct{39};
et249 = ct{40};
et250 = ct{41};
et251 = ct{42};
et252 = ct{43};
et253 = ct{44};
et254 = ct{45};
et255 = ct{46};
et256 = ct{47};
et257 = ct{48};
et258 = ct{49};
et259 = ct{50};
et260 = ct{51};
et261 = ct{52};
et262 = ct{53};
et263 = ct{54};
et264 = ct{55};
et265 = ct{56};
et266 = ct{57};
et267 = ct{58};
et268 = ct{59};
et269 = ct{60};
et270 = ct{61};
et271 = ct{62};
et272 = ct{63};
et273 = ct{64};
et274 = ct{65};
et275 = ct{66};
et276 = ct{67};
et277 = ct{68};
et278 = ct{69};
et279 = ct{70};
et280 = ct{71};
et281 = ct{72};
et282 = ct{73};
et283 = ct{74};
et284 = ct{75};
et285 = ct{76};
et286 = ct{77};
et287 = ct{78};
et288 = ct{79};
et289 = ct{80};
et290 = ct{81};
et291 = ct{82};
et292 = ct{83};
et293 = ct{84};
et294 = ct{85};
et295 = ct{86};
et296 = ct{87};
et297 = ct{88};
et298 = ct{89};
et299 = ct{90};
et300 = ct{91};
et301 = ct{92};
et302 = ct{93};
et303 = ct{94};
et304 = ct{95};
et305 = ct{96};
et306 = ct{97};
et307 = ct{98};
et308 = ct{99};
et309 = ct{100};
et310 = ct{101};
et311 = ct{102};
et312 = ct{103};
et313 = ct{104};
et314 = ct{105};
et315 = ct{106};
et316 = ct{107};
et317 = ct{108};
et318 = ct{109};
et319 = ct{110};
et320 = ct{111};
et321 = ct{112};
et322 = ct{113};
et323 = ct{114};
et324 = ct{115};
et325 = ct{116};
et326 = ct{117};
et327 = ct{118};
et328 = ct{119};
et329 = ct{120};
et330 = ct{121};
et331 = ct{122};
et332 = ct{123};
et333 = ct{124};
et334 = ct{125};
et335 = ct{126};
et336 = ct{127};
et337 = ct{128};
et338 = ct{129};
et339 = ct{130};
et340 = ct{131};
et341 = ct{132};
et342 = ct{133};
et343 = ct{134};
et344 = ct{135};
et345 = ct{136};
et346 = ct{137};
et347 = ct{138};
et348 = ct{139};
et349 = ct{140};
et350 = ct{141};
et351 = ct{142};
et352 = ct{143};
et353 = ct{144};
et354 = ct{145};
et355 = ct{146};
et356 = ct{147};
et357 = ct{148};
et358 = ct{149};
et359 = ct{150};
et360 = ct{151};
et361 = ct{152};
et362 = ct{153};
et363 = ct{154};
et364 = ct{155};
et365 = ct{156};
et366 = ct{157};
et367 = ct{158};
et368 = ct{159};
et369 = ct{160};
et370 = ct{161};
et371 = ct{162};
et372 = ct{163};
et373 = ct{164};
et374 = ct{165};
et375 = ct{166};
et376 = ct{167};
et377 = ct{168};
et378 = ct{169};
et379 = ct{170};
et380 = ct{171};
et381 = ct{172};
et382 = ct{173};
et383 = ct{174};
et384 = ct{175};
et385 = ct{176};
et386 = ct{177};
et387 = ct{178};
et388 = ct{179};
et389 = ct{180};
et390 = ct{181};
et391 = ct{182};
et392 = ct{183};
et393 = ct{184};
et394 = ct{185};
et395 = ct{186};
et396 = ct{187};
et397 = ct{188};
et398 = ct{189};
et399 = ct{190};
et400 = ct{191};
et401 = ct{192};
et402 = ct{193};
et403 = ct{194};
et404 = ct{195};
et405 = ct{196};
et406 = ct{197};
et407 = ct{198};
et408 = ct{199};
et409 = ct{200};
et410 = ct{201};
et411 = ct{202};
et412 = ct{203};
et413 = ct{204};
et414 = ct{205};
et415 = ct{206};
et416 = ct{207};
et417 = ct{208};
et418 = ct{209};
et419 = ct{210};
et420 = ct{211};
et421 = ct{212};
et422 = ct{213};
et423 = ct{214};
et424 = ct{215};
et425 = ct{216};
et426 = ct{217};
et427 = ct{218};
et428 = ct{219};
et429 = ct{220};
et430 = ct{221};
et431 = ct{222};
et432 = ct{223};
et433 = ct{224};
et434 = ct{225};
et435 = ct{226};
et436 = ct{227};
et437 = ct{228};
et438 = ct{229};
et439 = ct{230};
et440 = ct{231};
et441 = ct{232};
et442 = ct{233};
et443 = ct{234};
et444 = ct{235};
et445 = ct{236};
et446 = ct{237};
et447 = ct{238};
et448 = ct{239};
et449 = ct{240};
et450 = ct{241};
et451 = ct{242};
et452 = ct{243};
et453 = ct{244};
et454 = ct{245};
et455 = ct{246};
et456 = ct{247};
et457 = ct{248};
et458 = ct{249};
et459 = ct{250};
et460 = ct{251};
et461 = ct{252};
et462 = ct{253};
et463 = ct{254};
et464 = ct{255};
et465 = ct{256};
et466 = ct{257};
et467 = ct{258};
et468 = ct{259};
et469 = ct{260};
et470 = ct{261};
et471 = ct{262};
et472 = ct{263};
et473 = ct{264};
et474 = ct{265};
et475 = ct{266};
et476 = ct{267};
et477 = ct{268};
et478 = ct{269};
et479 = ct{270};
et480 = ct{271};
et481 = ct{272};
et482 = ct{273};
et483 = ct{274};
et484 = ct{275};
et485 = ct{276};
et486 = ct{277};
et487 = ct{278};
et488 = ct{279};
et489 = ct{280};
et490 = ct{281};
et491 = ct{282};
et492 = ct{283};
et493 = ct{284};
et494 = ct{285};
et495 = ct{286};
et496 = ct{287};
et497 = ct{288};
et498 = ct{289};
et499 = ct{290};
et500 = ct{291};
et501 = ct{292};
et502 = ct{293};
et503 = ct{294};
et504 = ct{295};
et505 = ct{296};
et506 = ct{297};
et507 = ct{298};
et508 = ct{299};
et509 = ct{300};
et510 = ct{301};
et511 = ct{302};
et512 = ct{303};
et513 = ct{304};
et514 = ct{305};
et515 = ct{306};
et516 = ct{307};
et517 = ct{308};
et518 = ct{309};
et519 = ct{310};
et520 = ct{311};
et521 = ct{312};
et522 = ct{313};
et523 = ct{314};
et524 = ct{315};
et525 = ct{316};
et526 = ct{317};
et527 = ct{318};
et528 = ct{319};
et529 = ct{320};
et530 = ct{321};
et531 = ct{322};
et532 = ct{323};
et533 = ct{324};
et534 = ct{325};
et535 = ct{326};
et536 = ct{327};
et537 = ct{328};
et538 = ct{329};
et539 = ct{330};
et540 = ct{331};
et541 = ct{332};
et542 = ct{333};
et543 = ct{334};
et544 = ct{335};
et545 = ct{336};
et546 = ct{337};
et547 = ct{338};
et548 = ct{339};
et549 = ct{340};
et550 = ct{341};
et551 = ct{342};
et552 = ct{343};
et553 = ct{344};
et554 = ct{345};
et555 = ct{346};
et556 = ct{347};
et557 = ct{348};
et558 = ct{349};
et559 = ct{350};
et560 = ct{351};
et561 = ct{352};
et562 = ct{353};
et563 = ct{354};
et564 = ct{355};
et565 = ct{356};
et566 = ct{357};
et567 = ct{358};
et568 = ct{359};
et569 = ct{360};
et570 = ct{361};
et571 = ct{362};
et572 = ct{363};
et573 = ct{364};
et574 = ct{365};
et575 = ct{366};
et576 = ct{367};
et577 = ct{368};
et578 = ct{369};
et579 = ct{370};
et580 = ct{371};
et581 = ct{372};
et582 = ct{373};
et583 = ct{374};
et584 = ct{375};
et585 = ct{376};
et586 = ct{377};
et587 = ct{378};
et588 = ct{379};
et589 = ct{380};
et590 = ct{381};
et591 = ct{382};
et592 = ct{383};
et593 = ct{384};
et594 = ct{385};
